simulink model "KUKA_LBR_Simulink_model_flatness_based_control"  (R2017a)
(part 8 of 19)

dblMassInertFullRow5Col2 = -(sin(q1)*(KUKA_LBR_param_.dblLink7InertXY*cos(q4)*sin(q1)*sin(q2) + KUKA_LBR_param_.dblLink7InertXZ*cos(q3)*sin(q2)*sin(q4) + KUKA_LBR_param_.dblLink7InertXX*sin(q1)*sin(q3)*sin(q4) + cos(q2)*(KUKA_LBR_param_.dblLink7InertXZ*cos(q4) - cos(q3)*(KUKA_LBR_param_.dblLink7InertXX*cos(q1) + KUKA_LBR_param_.dblLink7InertXY*sin(q1))*sin(q4)) + cos(q1)*(KUKA_LBR_param_.dblLink7InertXX*cos(q4)*sin(q2) - KUKA_LBR_param_.dblLink7InertXY*sin(q3)*sin(q4)))) + cos(q1)*(KUKA_LBR_param_.dblLink7InertYY*cos(q4)*sin(q1)*sin(q2) + KUKA_LBR_param_.dblLink7InertYZ*cos(q3)*sin(q2)*sin(q4) + KUKA_LBR_param_.dblLink7InertXY*sin(q1)*sin(q3)*sin(q4) + cos(q2)*(KUKA_LBR_param_.dblLink7InertYZ*cos(q4) - cos(q3)*(KUKA_LBR_param_.dblLink7InertXY*cos(q1) + KUKA_LBR_param_.dblLink7InertYY*sin(q1))*sin(q4)) + cos(q1)*(KUKA_LBR_param_.dblLink7InertXY*cos(q4)*sin(q2) - KUKA_LBR_param_.dblLink7InertYY*sin(q3)*sin(q4))) + (-2*KUKA_LBR_param_.dblLink5InertXZ*cos(q2)*cos(q4)*sin(q1) - 2*KUKA_LBR_param_.dblLink5InertXY*cos(q4)*power(sin(q1),2)*sin(q2) + 2*KUKA_LBR_param_.dblLink23Len*KUKA_LBR_param_.dblLink5CogX*KUKA_LBR_param_.dblLink5Mass*cos(q5)*sin(q3) + 2*KUKA_LBR_param_.dblLink45Len*KUKA_LBR_param_.dblLink5CogX*KUKA_LBR_param_.dblLink5Mass*cos(q4)*cos(q5)*sin(q3) + 2*KUKA_LBR_param_.dblLink5CogX*KUKA_LBR_param_.dblLink5CogZ*KUKA_LBR_param_.dblLink5Mass*cos(q4)*cos(q5)*sin(q3) - KUKA_LBR_param_.dblLink5InertXX*sin(q3)*sin(q4) - KUKA_LBR_param_.dblLink5InertYY*sin(q3)*sin(q4) - 2*power(KUKA_LBR_param_.dblLink5CogX,2)*KUKA_LBR_param_.dblLink5Mass*sin(q3)*sin(q4) - 2*power(KUKA_LBR_param_.dblLink5CogY,2)*KUKA_LBR_param_.dblLink5Mass*sin(q3)*sin(q4) - KUKA_LBR_param_.dblLink5InertXX*power(sin(q1),2)*sin(q3)*sin(q4) + KUKA_LBR_param_.dblLink5InertYY*power(sin(q1),2)*sin(q3)*sin(q4) + 2*KUKA_LBR_param_.dblLink5InertXY*sin(2*q1)*sin(q3)*sin(q4) + power(cos(q1),2)*(2*KUKA_LBR_param_.dblLink5InertXY*cos(q4)*sin(q2) + (-2*KUKA_LBR_param_.dblLink5InertXY*cos(q2)*cos(q3) + (KUKA_LBR_param_.dblLink5InertXX - KUKA_LBR_param_.dblLink5InertYY)*sin(q3))*sin(q4)) + 2*cos(q1)*(sin(q2)*(-((KUKA_LBR_param_.dblLink5InertXX - KUKA_LBR_param_.dblLink5InertYY)*cos(q4)*sin(q1)) + KUKA_LBR_param_.dblLink5InertYZ*cos(q3)*sin(q4)) + cos(q2)*(KUKA_LBR_param_.dblLink5InertYZ*cos(q4) + (KUKA_LBR_param_.dblLink5InertXX - KUKA_LBR_param_.dblLink5InertYY)*cos(q3)*sin(q1)*sin(q4))) - 2*KUKA_LBR_param_.dblLink23Len*KUKA_LBR_param_.dblLink5CogY*KUKA_LBR_param_.dblLink5Mass*sin(q3)*sin(q5) - 2*KUKA_LBR_param_.dblLink45Len*KUKA_LBR_param_.dblLink5CogY*KUKA_LBR_param_.dblLink5Mass*cos(q4)*sin(q3)*sin(q5) - 2*KUKA_LBR_param_.dblLink5CogY*KUKA_LBR_param_.dblLink5CogZ*KUKA_LBR_param_.dblLink5Mass*cos(q4)*sin(q3)*sin(q5) + 2*cos(q3)*(KUKA_LBR_param_.dblLink5CogY*KUKA_LBR_param_.dblLink5Mass*(KUKA_LBR_param_.dblLink45Len + KUKA_LBR_param_.dblLink5CogZ + KUKA_LBR_param_.dblLink23Len*cos(q4))*cos(q5) + KUKA_LBR_param_.dblLink5InertXY*cos(q2)*power(sin(q1),2)*sin(q4) - KUKA_LBR_param_.dblLink5InertXZ*sin(q1)*sin(q2)*sin(q4) + KUKA_LBR_param_.dblLink45Len*KUKA_LBR_param_.dblLink5CogX*KUKA_LBR_param_.dblLink5Mass*sin(q5) + KUKA_LBR_param_.dblLink5CogX*KUKA_LBR_param_.dblLink5CogZ*KUKA_LBR_param_.dblLink5Mass*sin(q5) + KUKA_LBR_param_.dblLink23Len*KUKA_LBR_param_.dblLink5CogX*KUKA_LBR_param_.dblLink5Mass*cos(q4)*sin(q5)))/2.0 + (-2*KUKA_LBR_param_.dblLink6InertXZ*cos(q2)*cos(q4)*sin(q1) - 2*KUKA_LBR_param_.dblLink6InertXY*cos(q4)*power(sin(q1),2)*sin(q2) + KUKA_LBR_param_.dblLink6InertYY*cos(q4)*sin(2*q1)*sin(q2) + 2*KUKA_LBR_param_.dblLink23Len*KUKA_LBR_param_.dblLink6CogX*KUKA_LBR_param_.dblLink6Mass*cos(q5)*cos(q6)*sin(q3) + 2*KUKA_LBR_param_.dblLink45Len*KUKA_LBR_param_.dblLink6CogX*KUKA_LBR_param_.dblLink6Mass*cos(q4)*cos(q5)*cos(q6)*sin(q3) + 2*KUKA_LBR_param_.dblLink6CogX*KUKA_LBR_param_.dblLink6CogY*KUKA_LBR_param_.dblLink6Mass*cos(q4)*cos(q5)*power(cos(q6),2)*sin(q3) - KUKA_LBR_param_.dblLink6InertXX*sin(q3)*sin(q4) - KUKA_LBR_param_.dblLink6InertYY*sin(q3)*sin(q4) - power(KUKA_LBR_param_.dblLink6CogX,2)*KUKA_LBR_param_.dblLink6Mass*sin(q3)*sin(q4) - power(KUKA_LBR_param_.dblLink6CogY,2)*KUKA_LBR_param_.dblLink6Mass*sin(q3)*sin(q4) - 2*power(KUKA_LBR_param_.dblLink6CogZ,2)*KUKA_LBR_param_.dblLink6Mass*sin(q3)*sin(q4) - power(KUKA_LBR_param_.dblLink6CogX,2)*KUKA_LBR_param_.dblLink6Mass*power(cos(q6),2)*sin(q3)*sin(q4) + power(KUKA_LBR_param_.dblLink6CogY,2)*KUKA_LBR_param_.dblLink6Mass*power(cos(q6),2)*sin(q3)*sin(q4) - KUKA_LBR_param_.dblLink6InertXX*power(sin(q1),2)*sin(q3)*sin(q4) + KUKA_LBR_param_.dblLink6InertYY*power(sin(q1),2)*sin(q3)*sin(q4) + power(cos(q1),2)*(2*KUKA_LBR_param_.dblLink6InertXY*cos(q4)*sin(q2) + (-2*KUKA_LBR_param_.dblLink6InertXY*cos(q2)*cos(q3) + (KUKA_LBR_param_.dblLink6InertXX - KUKA_LBR_param_.dblLink6InertYY)*sin(q3))*sin(q4)) + 2*cos(q1)*(-(KUKA_LBR_param_.dblLink6InertXX*cos(q4)*sin(q1)*sin(q2)) + KUKA_LBR_param_.dblLink6InertYZ*cos(q3)*sin(q2)*sin(q4) + 2*KUKA_LBR_param_.dblLink6InertXY*sin(q1)*sin(q3)*sin(q4) + cos(q2)*(KUKA_LBR_param_.dblLink6InertYZ*cos(q4) + (KUKA_LBR_param_.dblLink6InertXX - KUKA_LBR_param_.dblLink6InertYY)*cos(q3)*sin(q1)*sin(q4))) + 2*KUKA_LBR_param_.dblLink23Len*KUKA_LBR_param_.dblLink6CogZ*KUKA_LBR_param_.dblLink6Mass*sin(q3)*sin(q5) + 2*KUKA_LBR_param_.dblLink45Len*KUKA_LBR_param_.dblLink6CogZ*KUKA_LBR_param_.dblLink6Mass*cos(q4)*sin(q3)*sin(q5) + 2*KUKA_LBR_param_.dblLink6CogY*KUKA_LBR_param_.dblLink6CogZ*KUKA_LBR_param_.dblLink6Mass*cos(q4)*cos(q6)*sin(q3)*sin(q5) - 2*KUKA_LBR_param_.dblLink23Len*KUKA_LBR_param_.dblLink6CogY*KUKA_LBR_param_.dblLink6Mass*cos(q5)*sin(q3)*sin(q6) - 2*KUKA_LBR_param_.dblLink45Len*KUKA_LBR_param_.dblLink6CogY*KUKA_LBR_param_.dblLink6Mass*cos(q4)*cos(q5)*sin(q3)*sin(q6) - 2*power(KUKA_LBR_param_.dblLink6CogY,2)*KUKA_LBR_param_.dblLink6Mass*cos(q4)*cos(q5)*cos(q6)*sin(q3)*sin(q6) + 4*KUKA_LBR_param_.dblLink6CogX*KUKA_LBR_param_.dblLink6CogY*KUKA_LBR_param_.dblLink6Mass*cos(q6)*sin(q3)*sin(q4)*sin(q6) + 2*KUKA_LBR_param_.dblLink6CogX*KUKA_LBR_param_.dblLink6CogZ*KUKA_LBR_param_.dblLink6Mass*cos(q4)*sin(q3)*sin(q5)*sin(q6) - 2*KUKA_LBR_param_.dblLink6CogX*KUKA_LBR_param_.dblLink6CogY*KUKA_LBR_param_.dblLink6Mass*cos(q4)*cos(q5)*sin(q3)*power(sin(q6),2) + power(KUKA_LBR_param_.dblLink6CogX,2)*KUKA_LBR_param_.dblLink6Mass*sin(q3)*sin(q4)*power(sin(q6),2) - power(KUKA_LBR_param_.dblLink6CogY,2)*KUKA_LBR_param_.dblLink6Mass*sin(q3)*sin(q4)*power(sin(q6),2) + power(KUKA_LBR_param_.dblLink6CogX,2)*KUKA_LBR_param_.dblLink6Mass*cos(q4)*cos(q5)*sin(q3)*sin(2*q6) - cos(q3)*(-2*KUKA_LBR_param_.dblLink6InertXY*cos(q2)*power(sin(q1),2)*sin(q4) + 2*KUKA_LBR_param_.dblLink6InertXZ*sin(q1)*sin(q2)*sin(q4) - 2*KUKA_LBR_param_.dblLink45Len*KUKA_LBR_param_.dblLink6CogX*KUKA_LBR_param_.dblLink6Mass*cos(q6)*sin(q5) - 2*KUKA_LBR_param_.dblLink23Len*KUKA_LBR_param_.dblLink6CogX*KUKA_LBR_param_.dblLink6Mass*cos(q4)*cos(q6)*sin(q5) - 2*KUKA_LBR_param_.dblLink6CogX*KUKA_LBR_param_.dblLink6CogY*KUKA_LBR_param_.dblLink6Mass*power(cos(q6),2)*sin(q5) + 2*KUKA_LBR_param_.dblLink45Len*KUKA_LBR_param_.dblLink6CogY*KUKA_LBR_param_.dblLink6Mass*sin(q5)*sin(q6) + 2*KUKA_LBR_param_.dblLink23Len*KUKA_LBR_param_.dblLink6CogY*KUKA_LBR_param_.dblLink6Mass*cos(q4)*sin(q5)*sin(q6) + 2*KUKA_LBR_param_.dblLink6CogX*KUKA_LBR_param_.dblLink6CogY*KUKA_LBR_param_.dblLink6Mass*sin(q5)*power(sin(q6),2) + 2*KUKA_LBR_param_.dblLink6CogZ*KUKA_LBR_param_.dblLink6Mass*cos(q5)*(KUKA_LBR_param_.dblLink45Len + KUKA_LBR_param_.dblLink23Len*cos(q4) + KUKA_LBR_param_.dblLink6CogY*cos(q6) + KUKA_LBR_param_.dblLink6CogX*sin(q6)) - power(KUKA_LBR_param_.dblLink6CogX,2)*KUKA_LBR_param_.dblLink6Mass*sin(q5)*sin(2*q6) + power(KUKA_LBR_param_.dblLink6CogY,2)*KUKA_LBR_param_.dblLink6Mass*sin(q5)*sin(2*q6)))/2.0 - KUKA_LBR_param_.dblLink7Mass*(cos(q5)*(KUKA_LBR_param_.dblLink7CogZ*sin(q2)*sin(q3)*sin(q6) + cos(q2)*sin(q4)*(KUKA_LBR_param_.dblLink7CogY*cos(q7) + KUKA_LBR_param_.dblLink7CogX*sin(q7)) - cos(q6)*sin(q2)*sin(q3)*(KUKA_LBR_param_.dblLink7CogX*cos(q7) - KUKA_LBR_param_.dblLink7CogY*sin(q7))) + sin(q5)*(cos(q7)*(KUKA_LBR_param_.dblLink7CogY*sin(q2)*sin(q3) + KUKA_LBR_param_.dblLink7CogX*cos(q2)*cos(q6)*sin(q4)) + KUKA_LBR_param_.dblLink7CogX*sin(q2)*sin(q3)*sin(q7) - cos(q2)*sin(q4)*(KUKA_LBR_param_.dblLink7CogZ*sin(q6) + KUKA_LBR_param_.dblLink7CogY*cos(q6)*sin(q7))) - cos(q3)*cos(q4)*sin(q2)*(cos(q5)*(KUKA_LBR_param_.dblLink7CogY*cos(q7) + KUKA_LBR_param_.dblLink7CogX*sin(q7)) - sin(q5)*(KUKA_LBR_param_.dblLink7CogZ*sin(q6) + cos(q6)*(-(KUKA_LBR_param_.dblLink7CogX*cos(q7)) + KUKA_LBR_param_.dblLink7CogY*sin(q7)))))*(sin(q2)*(KUKA_LBR_param_.dblLink23Len + KUKA_LBR_param_.dblLink7CogY*cos(q7)*sin(q4)*sin(q5) + KUKA_LBR_param_.dblLink7CogX*sin(q4)*sin(q5)*sin(q7) + cos(q5)*sin(q4)*(-(KUKA_LBR_param_.dblLink7CogX*cos(q6)*cos(q7)) + KUKA_LBR_param_.dblLink7CogZ*sin(q6) + KUKA_LBR_param_.dblLink7CogY*cos(q6)*sin(q7)) + cos(q4)*(KUKA_LBR_param_.dblLink45Len + KUKA_LBR_param_.dblLink7CogZ*cos(q6) + KUKA_LBR_param_.dblLink7CogX*cos(q7)*sin(q6) - KUKA_LBR_param_.dblLink7CogY*sin(q6)*sin(q7))) + cos(q2)*(sin(q3)*(cos(q5)*(KUKA_LBR_param_.dblLink7CogY*cos(q7) + KUKA_LBR_param_.dblLink7CogX*sin(q7)) + sin(q5)*(KUKA_LBR_param_.dblLink7CogX*cos(q6)*cos(q7) - KUKA_LBR_param_.dblLink7CogZ*sin(q6) - KUKA_LBR_param_.dblLink7CogY*cos(q6)*sin(q7))) + cos(q3)*(-(sin(q4)*(KUKA_LBR_param_.dblLink45Len + KUKA_LBR_param_.dblLink7CogZ*cos(q6) + KUKA_LBR_param_.dblLink7CogX*cos(q7)*sin(q6) - KUKA_LBR_param_.dblLink7CogY*sin(q6)*sin(q7))) + cos(q4)*(sin(q5)*(KUKA_LBR_param_.dblLink7CogY*cos(q7) + KUKA_LBR_param_.dblLink7CogX*sin(q7)) + cos(q5)*(-(KUKA_LBR_param_.dblLink7CogX*cos(q6)*cos(q7)) + KUKA_LBR_param_.dblLink7CogZ*sin(q6) + KUKA_LBR_param_.dblLink7CogY*cos(q6)*sin(q7)))))) + KUKA_LBR_param_.dblLink7Mass*cos(q1)*(cos(q2)*(KUKA_LBR_param_.dblLink23Len + KUKA_LBR_param_.dblLink7CogY*cos(q7)*sin(q4)*sin(q5) + KUKA_LBR_param_.dblLink7CogX*sin(q4)*sin(q5)*sin(q7) + cos(q5)*sin(q4)*(-(KUKA_LBR_param_.dblLink7CogX*cos(q6)*cos(q7)) + KUKA_LBR_param_.dblLink7CogZ*sin(q6) + KUKA_LBR_param_.dblLink7CogY*cos(q6)*sin(q7)) + cos(q4)*(KUKA_LBR_param_.dblLink45Len + KUKA_LBR_param_.dblLink7CogZ*cos(q6) + KUKA_LBR_param_.dblLink7CogX*cos(q7)*sin(q6) - KUKA_LBR_param_.dblLink7CogY*sin(q6)*sin(q7))) + sin(q2)*(-(sin(q3)*(cos(q5)*(KUKA_LBR_param_.dblLink7CogY*cos(q7) + KUKA_LBR_param_.dblLink7CogX*sin(q7)) + sin(q5)*(KUKA_LBR_param_.dblLink7CogX*cos(q6)*cos(q7) - KUKA_LBR_param_.dblLink7CogZ*sin(q6) - KUKA_LBR_param_.dblLink7CogY*cos(q6)*sin(q7)))) + cos(q3)*(sin(q4)*(KUKA_LBR_param_.dblLink45Len + KUKA_LBR_param_.dblLink7CogZ*cos(q6) + KUKA_LBR_param_.dblLink7CogX*cos(q7)*sin(q6) - KUKA_LBR_param_.dblLink7CogY*sin(q6)*sin(q7)) - cos(q4)*(sin(q5)*(KUKA_LBR_param_.dblLink7CogY*cos(q7) + KUKA_LBR_param_.dblLink7CogX*sin(q7)) + cos(q5)*(-(KUKA_LBR_param_.dblLink7CogX*cos(q6)*cos(q7)) + KUKA_LBR_param_.dblLink7CogZ*sin(q6) + KUKA_LBR_param_.dblLink7CogY*cos(q6)*sin(q7))))))*(sin(q1)*(-(cos(q4)*sin(q3)*(cos(q5)*(KUKA_LBR_param_.dblLink7CogY*cos(q7) + KUKA_LBR_param_.dblLink7CogX*sin(q7)) + sin(q5)*(KUKA_LBR_param_.dblLink7CogX*cos(q6)*cos(q7) - KUKA_LBR_param_.dblLink7CogZ*sin(q6) - KUKA_LBR_param_.dblLink7CogY*cos(q6)*sin(q7)))) - cos(q3)*(sin(q5)*(KUKA_LBR_param_.dblLink7CogY*cos(q7) + KUKA_LBR_param_.dblLink7CogX*sin(q7)) + cos(q5)*(-(KUKA_LBR_param_.dblLink7CogX*cos(q6)*cos(q7)) + KUKA_LBR_param_.dblLink7CogZ*sin(q6) + KUKA_LBR_param_.dblLink7CogY*cos(q6)*sin(q7)))) + cos(q1)*(sin(q2)*sin(q4)*(cos(q5)*(KUKA_LBR_param_.dblLink7CogY*cos(q7) + KUKA_LBR_param_.dblLink7CogX*sin(q7)) + sin(q5)*(KUKA_LBR_param_.dblLink7CogX*cos(q6)*cos(q7) - KUKA_LBR_param_.dblLink7CogZ*sin(q6) - KUKA_LBR_param_.dblLink7CogY*cos(q6)*sin(q7))) + cos(q2)*(cos(q3)*cos(q4)*(cos(q5)*(KUKA_LBR_param_.dblLink7CogY*cos(q7) + KUKA_LBR_param_.dblLink7CogX*sin(q7)) + sin(q5)*(KUKA_LBR_param_.dblLink7CogX*cos(q6)*cos(q7) - KUKA_LBR_param_.dblLink7CogZ*sin(q6) - KUKA_LBR_param_.dblLink7CogY*cos(q6)*sin(q7))) - sin(q3)*(sin(q5)*(KUKA_LBR_param_.dblLink7CogY*cos(q7) + KUKA_LBR_param_.dblLink7CogX*sin(q7)) + cos(q5)*(-(KUKA_LBR_param_.dblLink7CogX*cos(q6)*cos(q7)) + KUKA_LBR_param_.dblLink7CogZ*sin(q6) + KUKA_LBR_param_.dblLink7CogY*cos(q6)*sin(q7)))))) + KUKA_LBR_param_.dblLink7Mass*sin(q1)*(cos(q2)*(KUKA_LBR_param_.dblLink23Len + KUKA_LBR_param_.dblLink7CogY*cos(q7)*sin(q4)*sin(q5) + KUKA_LBR_param_.dblLink7CogX*sin(q4)*sin(q5)*sin(q7) + cos(q5)*sin(q4)*(-(KUKA_LBR_param_.dblLink7CogX*cos(q6)*cos(q7)) + KUKA_LBR_param_.dblLink7CogZ*sin(q6) + KUKA_LBR_param_.dblLink7CogY*cos(q6)*sin(q7)) + cos(q4)*(KUKA_LBR_param_.dblLink45Len + KUKA_LBR_param_.dblLink7CogZ*cos(q6) + KUKA_LBR_param_.dblLink7CogX*cos(q7)*sin(q6) - KUKA_LBR_param_.dblLink7CogY*sin(q6)*sin(q7))) + sin(q2)*(-(sin(q3)*(cos(q5)*(KUKA_LBR_param_.dblLink7CogY*cos(q7) + KUKA_LBR_param_.dblLink7CogX*sin(q7)) + sin(q5)*(KUKA_LBR_param_.dblLink7CogX*cos(q6)*cos(q7) - KUKA_LBR_param_.dblLink7CogZ*sin(q6) - KUKA_LBR_param_.dblLink7CogY*cos(q6)*sin(q7)))) + cos(q3)*(sin(q4)*(KUKA_LBR_param_.dblLink45Len + KUKA_LBR_param_.dblLink7CogZ*cos(q6) + KUKA_LBR_param_.dblLink7CogX*cos(q7)*sin(q6) - KUKA_LBR_param_.dblLink7CogY*sin(q6)*sin(q7)) - cos(q4)*(sin(q5)*(KUKA_LBR_param_.dblLink7CogY*cos(q7) + KUKA_LBR_param_.dblLink7CogX*sin(q7)) + cos(q5)*(-(KUKA_LBR_param_.dblLink7CogX*cos(q6)*cos(q7)) + KUKA_LBR_param_.dblLink7CogZ*sin(q6) + KUKA_LBR_param_.dblLink7CogY*cos(q6)*sin(q7))))))*(cos(q1)*(cos(q4)*sin(q3)*(cos(q5)*(KUKA_LBR_param_.dblLink7CogY*cos(q7) + KUKA_LBR_param_.dblLink7CogX*sin(q7)) + sin(q5)*(KUKA_LBR_param_.dblLink7CogX*cos(q6)*cos(q7) - KUKA_LBR_param_.dblLink7CogZ*sin(q6) - KUKA_LBR_param_.dblLink7CogY*cos(q6)*sin(q7))) + cos(q3)*(sin(q5)*(KUKA_LBR_param_.dblLink7CogY*cos(q7) + KUKA_LBR_param_.dblLink7CogX*sin(q7)) + cos(q5)*(-(KUKA_LBR_param_.dblLink7CogX*cos(q6)*cos(q7)) + KUKA_LBR_param_.dblLink7CogZ*sin(q6) + KUKA_LBR_param_.dblLink7CogY*cos(q6)*sin(q7)))) + sin(q1)*(sin(q2)*sin(q4)*(cos(q5)*(KUKA_LBR_param_.dblLink7CogY*cos(q7) + KUKA_LBR_param_.dblLink7CogX*sin(q7)) + sin(q5)*(KUKA_LBR_param_.dblLink7CogX*cos(q6)*cos(q7) - KUKA_LBR_param_.dblLink7CogZ*sin(q6) - KUKA_LBR_param_.dblLink7CogY*cos(q6)*sin(q7))) + cos(q2)*(cos(q3)*cos(q4)*(cos(q5)*(KUKA_LBR_param_.dblLink7CogY*cos(q7) + KUKA_LBR_param_.dblLink7CogX*sin(q7)) + sin(q5)*(KUKA_LBR_param_.dblLink7CogX*cos(q6)*cos(q7) - KUKA_LBR_param_.dblLink7CogZ*sin(q6) - KUKA_LBR_param_.dblLink7CogY*cos(q6)*sin(q7))) - sin(q3)*(sin(q5)*(KUKA_LBR_param_.dblLink7CogY*cos(q7) + KUKA_LBR_param_.dblLink7CogX*sin(q7)) + cos(q5)*(-(KUKA_LBR_param_.dblLink7CogX*cos(q6)*cos(q7)) + KUKA_LBR_param_.dblLink7CogZ*sin(q6) + KUKA_LBR_param_.dblLink7CogY*cos(q6)*sin(q7))))));
dblMassInertFullRow5Col3 = cos(q1)*sin(q2)*(KUKA_LBR_param_.dblLink7InertXY*cos(q4)*sin(q1)*sin(q2) + KUKA_LBR_param_.dblLink7InertXZ*cos(q3)*sin(q2)*sin(q4) + KUKA_LBR_param_.dblLink7InertXX*sin(q1)*sin(q3)*sin(q4) + cos(q2)*(KUKA_LBR_param_.dblLink7InertXZ*cos(q4) - cos(q3)*(KUKA_LBR_param_.dblLink7InertXX*cos(q1) + KUKA_LBR_param_.dblLink7InertXY*sin(q1))*sin(q4)) + cos(q1)*(KUKA_LBR_param_.dblLink7InertXX*cos(q4)*sin(q2) - KUKA_LBR_param_.dblLink7InertXY*sin(q3)*sin(q4))) + sin(q1)*sin(q2)*(KUKA_LBR_param_.dblLink7InertYY*cos(q4)*sin(q1)*sin(q2) + KUKA_LBR_param_.dblLink7InertYZ*cos(q3)*sin(q2)*sin(q4) + KUKA_LBR_param_.dblLink7InertXY*sin(q1)*sin(q3)*sin(q4) + cos(q2)*(KUKA_LBR_param_.dblLink7InertYZ*cos(q4) - cos(q3)*(KUKA_LBR_param_.dblLink7InertXY*cos(q1) + KUKA_LBR_param_.dblLink7InertYY*sin(q1))*sin(q4)) + cos(q1)*(KUKA_LBR_param_.dblLink7InertXY*cos(q4)*sin(q2) - KUKA_LBR_param_.dblLink7InertYY*sin(q3)*sin(q4))) + cos(q2)*(KUKA_LBR_param_.dblLink7InertYZ*cos(q4)*sin(q1)*sin(q2) + KUKA_LBR_param_.dblLink7InertZZ*cos(q3)*sin(q2)*sin(q4) + KUKA_LBR_param_.dblLink7InertXZ*sin(q1)*sin(q3)*sin(q4) + cos(q2)*(KUKA_LBR_param_.dblLink7InertZZ*cos(q4) - cos(q3)*(KUKA_LBR_param_.dblLink7InertXZ*cos(q1) + KUKA_LBR_param_.dblLink7InertYZ*sin(q1))*sin(q4)) + cos(q1)*(KUKA_LBR_param_.dblLink7InertXZ*cos(q4)*sin(q2) - KUKA_LBR_param_.dblLink7InertYZ*sin(q3)*sin(q4))) + (cos(q4)*(2*KUKA_LBR_param_.dblLink5InertXX + 2*KUKA_LBR_param_.dblLink5InertYY + 4*KUKA_LBR_param_.dblLink5InertZZ + 8*power(KUKA_LBR_param_.dblLink5CogX,2)*KUKA_LBR_param_.dblLink5Mass + 8*power(KUKA_LBR_param_.dblLink5CogY,2)*KUKA_LBR_param_.dblLink5Mass + 2*(KUKA_LBR_param_.dblLink5InertXX - KUKA_LBR_param_.dblLink5InertYY)*cos(2*q1) + 4*KUKA_LBR_param_.dblLink5InertYZ*cos(q1 - 2*q2) - KUKA_LBR_param_.dblLink5InertXX*cos(2*(q1 - q2)) + KUKA_LBR_param_.dblLink5InertYY*cos(2*(q1 - q2)) - 2*KUKA_LBR_param_.dblLink5InertXX*cos(2*q2) - 2*KUKA_LBR_param_.dblLink5InertYY*cos(2*q2) + 4*KUKA_LBR_param_.dblLink5InertZZ*cos(2*q2) - KUKA_LBR_param_.dblLink5InertXX*cos(2*(q1 + q2)) + KUKA_LBR_param_.dblLink5InertYY*cos(2*(q1 + q2)) - 4*KUKA_LBR_param_.dblLink5InertYZ*cos(q1 + 2*q2) + 4*KUKA_LBR_param_.dblLink5InertXY*sin(2*q1) - 4*KUKA_LBR_param_.dblLink5InertXZ*sin(q1 - 2*q2) - 2*KUKA_LBR_param_.dblLink5InertXY*sin(2*(q1 - q2)) - 2*KUKA_LBR_param_.dblLink5InertXY*sin(2*(q1 + q2)) + 4*KUKA_LBR_param_.dblLink5InertXZ*sin(q1 + 2*q2)) - 4*sin(q4)*(-2*KUKA_LBR_param_.dblLink5CogX*(KUKA_LBR_param_.dblLink45Len + KUKA_LBR_param_.dblLink5CogZ)*KUKA_LBR_param_.dblLink5Mass*cos(q5) + 2*KUKA_LBR_param_.dblLink5InertYZ*power(cos(q2),2)*cos(q3)*sin(q1) + KUKA_LBR_param_.dblLink5InertXX*cos(q2)*cos(q3)*sin(q2) + KUKA_LBR_param_.dblLink5InertYY*cos(q2)*cos(q3)*sin(q2) - 2*KUKA_LBR_param_.dblLink5InertZZ*cos(q2)*cos(q3)*sin(q2) - KUKA_LBR_param_.dblLink5InertXX*cos(q2)*cos(q3)*power(sin(q1),2)*sin(q2) + KUKA_LBR_param_.dblLink5InertYY*cos(q2)*cos(q3)*power(sin(q1),2)*sin(q2) - 2*KUKA_LBR_param_.dblLink5InertYZ*cos(q3)*sin(q1)*power(sin(q2),2) + KUKA_LBR_param_.dblLink5InertXY*cos(q3)*sin(2*q1)*sin(2*q2) - 2*KUKA_LBR_param_.dblLink5InertXZ*cos(q2)*sin(q1)*sin(q3) - 2*KUKA_LBR_param_.dblLink5InertXY*power(sin(q1),2)*sin(q2)*sin(q3) + KUKA_LBR_param_.dblLink5InertYY*sin(2*q1)*sin(q2)*sin(q3) + power(cos(q1),2)*sin(q2)*((KUKA_LBR_param_.dblLink5InertXX - KUKA_LBR_param_.dblLink5InertYY)*cos(q2)*cos(q3) + 2*KUKA_LBR_param_.dblLink5InertXY*sin(q3)) + 2*cos(q1)*(KUKA_LBR_param_.dblLink5InertXZ*power(cos(q2),2)*cos(q3) + KUKA_LBR_param_.dblLink5InertYZ*cos(q2)*sin(q3) - sin(q2)*(KUKA_LBR_param_.dblLink5InertXZ*cos(q3)*sin(q2) + KUKA_LBR_param_.dblLink5InertXX*sin(q1)*sin(q3))) + 2*KUKA_LBR_param_.dblLink45Len*KUKA_LBR_param_.dblLink5CogY*KUKA_LBR_param_.dblLink5Mass*sin(q5) + 2*KUKA_LBR_param_.dblLink5CogY*KUKA_LBR_param_.dblLink5CogZ*KUKA_LBR_param_.dblLink5Mass*sin(q5)))/8.0 + (2*sin(q4)*(-4*KUKA_LBR_param_.dblLink6InertYZ*power(cos(q2),2)*cos(q3)*sin(q1) - 2*KUKA_LBR_param_.dblLink6InertXX*cos(q2)*cos(q3)*sin(q2) - 2*KUKA_LBR_param_.dblLink6InertYY*cos(q2)*cos(q3)*sin(q2) + 4*KUKA_LBR_param_.dblLink6InertZZ*cos(q2)*cos(q3)*sin(q2) - 2*KUKA_LBR_param_.dblLink6InertYY*cos(q2)*cos(q3)*power(sin(q1),2)*sin(q2) + 4*KUKA_LBR_param_.dblLink6InertYZ*cos(q3)*sin(q1)*power(sin(q2),2) + KUKA_LBR_param_.dblLink6InertXX*cos(q3)*power(sin(q1),2)*sin(2*q2) + 4*KUKA_LBR_param_.dblLink6InertXZ*cos(q2)*sin(q1)*sin(q3) + 4*KUKA_LBR_param_.dblLink6InertXY*power(sin(q1),2)*sin(q2)*sin(q3) + power(cos(q1),2)*(-2*KUKA_LBR_param_.dblLink6InertXX*cos(q2)*cos(q3)*sin(q2) + KUKA_LBR_param_.dblLink6InertYY*cos(q3)*sin(2*q2) - 4*KUKA_LBR_param_.dblLink6InertXY*sin(q2)*sin(q3)) - 4*cos(q1)*(KUKA_LBR_param_.dblLink6InertXZ*power(cos(q2),2)*cos(q3) + cos(q3)*(-(KUKA_LBR_param_.dblLink6InertXZ*power(sin(q2),2)) + KUKA_LBR_param_.dblLink6InertXY*sin(q1)*sin(2*q2)) + KUKA_LBR_param_.dblLink6InertYZ*cos(q2)*sin(q3) + (-KUKA_LBR_param_.dblLink6InertXX + KUKA_LBR_param_.dblLink6InertYY)*sin(q1)*sin(q2)*sin(q3)) + 4*KUKA_LBR_param_.dblLink45Len*KUKA_LBR_param_.dblLink6CogZ*KUKA_LBR_param_.dblLink6Mass*sin(q5) + 4*KUKA_LBR_param_.dblLink6CogY*KUKA_LBR_param_.dblLink6CogZ*KUKA_LBR_param_.dblLink6Mass*cos(q6)*sin(q5) + 4*KUKA_LBR_param_.dblLink6CogX*KUKA_LBR_param_.dblLink6CogZ*KUKA_LBR_param_.dblLink6Mass*sin(q5)*sin(q6) + 4*KUKA_LBR_param_.dblLink6Mass*cos(q5)*(KUKA_LBR_param_.dblLink45Len + KUKA_LBR_param_.dblLink6CogY*cos(q6) + KUKA_LBR_param_.dblLink6CogX*sin(q6))*(KUKA_LBR_param_.dblLink6CogX*cos(q6) - KUKA_LBR_param_.dblLink6CogY*sin(q6))) + cos(q4)*(2*KUKA_LBR_param_.dblLink6InertXX + 2*KUKA_LBR_param_.dblLink6InertYY + 4*KUKA_LBR_param_.dblLink6InertZZ + 4*power(KUKA_LBR_param_.dblLink6CogX,2)*KUKA_LBR_param_.dblLink6Mass + 4*power(KUKA_LBR_param_.dblLink6CogY,2)*KUKA_LBR_param_.dblLink6Mass + 8*power(KUKA_LBR_param_.dblLink6CogZ,2)*KUKA_LBR_param_.dblLink6Mass + 2*(KUKA_LBR_param_.dblLink6InertXX - KUKA_LBR_param_.dblLink6InertYY)*cos(2*q1) + 4*KUKA_LBR_param_.dblLink6InertYZ*cos(q1 - 2*q2) - KUKA_LBR_param_.dblLink6InertXX*cos(2*(q1 - q2)) + KUKA_LBR_param_.dblLink6InertYY*cos(2*(q1 - q2)) - 2*KUKA_LBR_param_.dblLink6InertXX*cos(2*q2) - 2*KUKA_LBR_param_.dblLink6InertYY*cos(2*q2) + 4*KUKA_LBR_param_.dblLink6InertZZ*cos(2*q2) - KUKA_LBR_param_.dblLink6InertXX*cos(2*(q1 + q2)) + KUKA_LBR_param_.dblLink6InertYY*cos(2*(q1 + q2)) - 4*KUKA_LBR_param_.dblLink6InertYZ*cos(q1 + 2*q2) + 4*power(KUKA_LBR_param_.dblLink6CogX,2)*KUKA_LBR_param_.dblLink6Mass*cos(2*q6) - 4*power(KUKA_LBR_param_.dblLink6CogY,2)*KUKA_LBR_param_.dblLink6Mass*cos(2*q6) + 4*KUKA_LBR_param_.dblLink6InertXY*sin(2*q1) - 4*KUKA_LBR_param_.dblLink6InertXZ*sin(q1 - 2*q2) - 2*KUKA_LBR_param_.dblLink6InertXY*sin(2*(q1 - q2)) - 2*KUKA_LBR_param_.dblLink6InertXY*sin(2*(q1 + q2)) + 4*KUKA_LBR_param_.dblLink6InertXZ*sin(q1 + 2*q2) - 8*KUKA_LBR_param_.dblLink6CogX*KUKA_LBR_param_.dblLink6CogY*KUKA_LBR_param_.dblLink6Mass*sin(2*q6)))/8.0 + KUKA_LBR_param_.dblLink7Mass*sin(q2)*(cos(q5)*(KUKA_LBR_param_.dblLink7CogZ*sin(q2)*sin(q3)*sin(q6) + cos(q2)*sin(q4)*(KUKA_LBR_param_.dblLink7CogY*cos(q7) + KUKA_LBR_param_.dblLink7CogX*sin(q7)) - cos(q6)*sin(q2)*sin(q3)*(KUKA_LBR_param_.dblLink7CogX*cos(q7) - KUKA_LBR_param_.dblLink7CogY*sin(q7))) + sin(q5)*(cos(q7)*(KUKA_LBR_param_.dblLink7CogY*sin(q2)*sin(q3) + KUKA_LBR_param_.dblLink7CogX*cos(q2)*cos(q6)*sin(q4)) + KUKA_LBR_param_.dblLink7CogX*sin(q2)*sin(q3)*sin(q7) - cos(q2)*sin(q4)*(KUKA_LBR_param_.dblLink7CogZ*sin(q6) + KUKA_LBR_param_.dblLink7CogY*cos(q6)*sin(q7))) - cos(q3)*cos(q4)*sin(q2)*(cos(q5)*(KUKA_LBR_param_.dblLink7CogY*cos(q7) + KUKA_LBR_param_.dblLink7CogX*sin(q7)) - sin(q5)*(KUKA_LBR_param_.dblLink7CogZ*sin(q6) + cos(q6)*(-(KUKA_LBR_param_.dblLink7CogX*cos(q7)) + KUKA_LBR_param_.dblLink7CogY*sin(q7)))))*(-(cos(q3)*(cos(q5)*(KUKA_LBR_param_.dblLink7CogY*cos(q7) + KUKA_LBR_param_.dblLink7CogX*sin(q7)) + sin(q5)*(KUKA_LBR_param_.dblLink7CogX*cos(q6)*cos(q7) - KUKA_LBR_param_.dblLink7CogZ*sin(q6) - KUKA_LBR_param_.dblLink7CogY*cos(q6)*sin(q7)))) + sin(q3)*(-(sin(q4)*(KUKA_LBR_param_.dblLink45Len + KUKA_LBR_param_.dblLink7CogZ*cos(q6) + KUKA_LBR_param_.dblLink7CogX*cos(q7)*sin(q6) - KUKA_LBR_param_.dblLink7CogY*sin(q6)*sin(q7))) + cos(q4)*(sin(q5)*(KUKA_LBR_param_.dblLink7CogY*cos(q7) + KUKA_LBR_param_.dblLink7CogX*sin(q7)) + cos(q5)*(-(KUKA_LBR_param_.dblLink7CogX*cos(q6)*cos(q7)) + KUKA_LBR_param_.dblLink7CogZ*sin(q6) + KUKA_LBR_param_.dblLink7CogY*cos(q6)*sin(q7))))) + KUKA_LBR_param_.dblLink7Mass*(sin(q1)*(-(sin(q3)*(cos(q5)*(KUKA_LBR_param_.dblLink7CogY*cos(q7) + KUKA_LBR_param_.dblLink7CogX*sin(q7)) + sin(q5)*(KUKA_LBR_param_.dblLink7CogX*cos(q6)*cos(q7) - KUKA_LBR_param_.dblLink7CogZ*sin(q6) - KUKA_LBR_param_.dblLink7CogY*cos(q6)*sin(q7)))) + cos(q3)*(sin(q4)*(KUKA_LBR_param_.dblLink45Len + KUKA_LBR_param_.dblLink7CogZ*cos(q6) + KUKA_LBR_param_.dblLink7CogX*cos(q7)*sin(q6) - KUKA_LBR_param_.dblLink7CogY*sin(q6)*sin(q7)) - cos(q4)*(sin(q5)*(KUKA_LBR_param_.dblLink7CogY*cos(q7) + KUKA_LBR_param_.dblLink7CogX*sin(q7)) + cos(q5)*(-(KUKA_LBR_param_.dblLink7CogX*cos(q6)*cos(q7)) + KUKA_LBR_param_.dblLink7CogZ*sin(q6) + KUKA_LBR_param_.dblLink7CogY*cos(q6)*sin(q7))))) + cos(q1)*cos(q2)*(cos(q3)*(cos(q5)*(KUKA_LBR_param_.dblLink7CogY*cos(q7) + KUKA_LBR_param_.dblLink7CogX*sin(q7)) + sin(q5)*(KUKA_LBR_param_.dblLink7CogX*cos(q6)*cos(q7) - KUKA_LBR_param_.dblLink7CogZ*sin(q6) - KUKA_LBR_param_.dblLink7CogY*cos(q6)*sin(q7))) + sin(q3)*(sin(q4)*(KUKA_LBR_param_.dblLink45Len + KUKA_LBR_param_.dblLink7CogZ*cos(q6) + KUKA_LBR_param_.dblLink7CogX*cos(q7)*sin(q6) - KUKA_LBR_param_.dblLink7CogY*sin(q6)*sin(q7)) - cos(q4)*(sin(q5)*(KUKA_LBR_param_.dblLink7CogY*cos(q7) + KUKA_LBR_param_.dblLink7CogX*sin(q7)) + cos(q5)*(-(KUKA_LBR_param_.dblLink7CogX*cos(q6)*cos(q7)) + KUKA_LBR_param_.dblLink7CogZ*sin(q6) + KUKA_LBR_param_.dblLink7CogY*cos(q6)*sin(q7))))))*(sin(q1)*(-(cos(q4)*sin(q3)*(cos(q5)*(KUKA_LBR_param_.dblLink7CogY*cos(q7) + KUKA_LBR_param_.dblLink7CogX*sin(q7)) + sin(q5)*(KUKA_LBR_param_.dblLink7CogX*cos(q6)*cos(q7) - KUKA_LBR_param_.dblLink7CogZ*sin(q6) - KUKA_LBR_param_.dblLink7CogY*cos(q6)*sin(q7)))) - cos(q3)*(sin(q5)*(KUKA_LBR_param_.dblLink7CogY*cos(q7) + KUKA_LBR_param_.dblLink7CogX*sin(q7)) + cos(q5)*(-(KUKA_LBR_param_.dblLink7CogX*cos(q6)*cos(q7)) + KUKA_LBR_param_.dblLink7CogZ*sin(q6) + KUKA_LBR_param_.dblLink7CogY*cos(q6)*sin(q7)))) + cos(q1)*(sin(q2)*sin(q4)*(cos(q5)*(KUKA_LBR_param_.dblLink7CogY*cos(q7) + KUKA_LBR_param_.dblLink7CogX*sin(q7)) + sin(q5)*(KUKA_LBR_param_.dblLink7CogX*cos(q6)*cos(q7) - KUKA_LBR_param_.dblLink7CogZ*sin(q6) - KUKA_LBR_param_.dblLink7CogY*cos(q6)*sin(q7))) + cos(q2)*(cos(q3)*cos(q4)*(cos(q5)*(KUKA_LBR_param_.dblLink7CogY*cos(q7) + KUKA_LBR_param_.dblLink7CogX*sin(q7)) + sin(q5)*(KUKA_LBR_param_.dblLink7CogX*cos(q6)*cos(q7) - KUKA_LBR_param_.dblLink7CogZ*sin(q6) - KUKA_LBR_param_.dblLink7CogY*cos(q6)*sin(q7))) - sin(q3)*(sin(q5)*(KUKA_LBR_param_.dblLink7CogY*cos(q7) + KUKA_LBR_param_.dblLink7CogX*sin(q7)) + cos(q5)*(-(KUKA_LBR_param_.dblLink7CogX*cos(q6)*cos(q7)) + KUKA_LBR_param_.dblLink7CogZ*sin(q6) + KUKA_LBR_param_.dblLink7CogY*cos(q6)*sin(q7)))))) + KUKA_LBR_param_.dblLink7Mass*(cos(q2)*sin(q1)*(cos(q3)*(cos(q5)*(KUKA_LBR_param_.dblLink7CogY*cos(q7) + KUKA_LBR_param_.dblLink7CogX*sin(q7)) + sin(q5)*(KUKA_LBR_param_.dblLink7CogX*cos(q6)*cos(q7) - KUKA_LBR_param_.dblLink7CogZ*sin(q6) - KUKA_LBR_param_.dblLink7CogY*cos(q6)*sin(q7))) + sin(q3)*(sin(q4)*(KUKA_LBR_param_.dblLink45Len + KUKA_LBR_param_.dblLink7CogZ*cos(q6) + KUKA_LBR_param_.dblLink7CogX*cos(q7)*sin(q6) - KUKA_LBR_param_.dblLink7CogY*sin(q6)*sin(q7)) - cos(q4)*(sin(q5)*(KUKA_LBR_param_.dblLink7CogY*cos(q7) + KUKA_LBR_param_.dblLink7CogX*sin(q7)) + cos(q5)*(-(KUKA_LBR_param_.dblLink7CogX*cos(q6)*cos(q7)) + KUKA_LBR_param_.dblLink7CogZ*sin(q6) + KUKA_LBR_param_.dblLink7CogY*cos(q6)*sin(q7))))) + cos(q1)*(sin(q3)*(cos(q5)*(KUKA_LBR_param_.dblLink7CogY*cos(q7) + KUKA_LBR_param_.dblLink7CogX*sin(q7)) + sin(q5)*(KUKA_LBR_param_.dblLink7CogX*cos(q6)*cos(q7) - KUKA_LBR_param_.dblLink7CogZ*sin(q6) - KUKA_LBR_param_.dblLink7CogY*cos(q6)*sin(q7))) + cos(q3)*(-(sin(q4)*(KUKA_LBR_param_.dblLink45Len + KUKA_LBR_param_.dblLink7CogZ*cos(q6) + KUKA_LBR_param_.dblLink7CogX*cos(q7)*sin(q6) - KUKA_LBR_param_.dblLink7CogY*sin(q6)*sin(q7))) + cos(q4)*(sin(q5)*(KUKA_LBR_param_.dblLink7CogY*cos(q7) + KUKA_LBR_param_.dblLink7CogX*sin(q7)) + cos(q5)*(-(KUKA_LBR_param_.dblLink7CogX*cos(q6)*cos(q7)) + KUKA_LBR_param_.dblLink7CogZ*sin(q6) + KUKA_LBR_param_.dblLink7CogY*cos(q6)*sin(q7))))))*(cos(q1)*(cos(q4)*sin(q3)*(cos(q5)*(KUKA_LBR_param_.dblLink7CogY*cos(q7) + KUKA_LBR_param_.dblLink7CogX*sin(q7)) + sin(q5)*(KUKA_LBR_param_.dblLink7CogX*cos(q6)*cos(q7) - KUKA_LBR_param_.dblLink7CogZ*sin(q6) - KUKA_LBR_param_.dblLink7CogY*cos(q6)*sin(q7))) + cos(q3)*(sin(q5)*(KUKA_LBR_param_.dblLink7CogY*cos(q7) + KUKA_LBR_param_.dblLink7CogX*sin(q7)) + cos(q5)*(-(KUKA_LBR_param_.dblLink7CogX*cos(q6)*cos(q7)) + KUKA_LBR_param_.dblLink7CogZ*sin(q6) + KUKA_LBR_param_.dblLink7CogY*cos(q6)*sin(q7)))) + sin(q1)*(sin(q2)*sin(q4)*(cos(q5)*(KUKA_LBR_param_.dblLink7CogY*cos(q7) + KUKA_LBR_param_.dblLink7CogX*sin(q7)) + sin(q5)*(KUKA_LBR_param_.dblLink7CogX*cos(q6)*cos(q7) - KUKA_LBR_param_.dblLink7CogZ*sin(q6) - KUKA_LBR_param_.dblLink7CogY*cos(q6)*sin(q7))) + cos(q2)*(cos(q3)*cos(q4)*(cos(q5)*(KUKA_LBR_param_.dblLink7CogY*cos(q7) + KUKA_LBR_param_.dblLink7CogX*sin(q7)) + sin(q5)*(KUKA_LBR_param_.dblLink7CogX*cos(q6)*cos(q7) - KUKA_LBR_param_.dblLink7CogZ*sin(q6) - KUKA_LBR_param_.dblLink7CogY*cos(q6)*sin(q7))) - sin(q3)*(sin(q5)*(KUKA_LBR_param_.dblLink7CogY*cos(q7) + KUKA_LBR_param_.dblLink7CogX*sin(q7)) + cos(q5)*(-(KUKA_LBR_param_.dblLink7CogX*cos(q6)*cos(q7)) + KUKA_LBR_param_.dblLink7CogZ*sin(q6) + KUKA_LBR_param_.dblLink7CogY*cos(q6)*sin(q7))))));
dblMassInertFullRow5Col4 = (cos(q3)*sin(q1) + cos(q1)*cos(q2)*sin(q3))*(KUKA_LBR_param_.dblLink7InertXY*cos(q4)*sin(q1)*sin(q2) + KUKA_LBR_param_.dblLink7InertXZ*cos(q3)*sin(q2)*sin(q4) + KUKA_LBR_param_.dblLink7InertXX*sin(q1)*sin(q3)*sin(q4) + cos(q2)*(KUKA_LBR_param_.dblLink7InertXZ*cos(q4) - cos(q3)*(KUKA_LBR_param_.dblLink7InertXX*cos(q1) + KUKA_LBR_param_.dblLink7InertXY*sin(q1))*sin(q4)) + cos(q1)*(KUKA_LBR_param_.dblLink7InertXX*cos(q4)*sin(q2) - KUKA_LBR_param_.dblLink7InertXY*sin(q3)*sin(q4))) + (-(cos(q1)*cos(q3)) + cos(q2)*sin(q1)*sin(q3))*(KUKA_LBR_param_.dblLink7InertYY*cos(q4)*sin(q1)*sin(q2) + KUKA_LBR_param_.dblLink7InertYZ*cos(q3)*sin(q2)*sin(q4) + KUKA_LBR_param_.dblLink7InertXY*sin(q1)*sin(q3)*sin(q4) + cos(q2)*(KUKA_LBR_param_.dblLink7InertYZ*cos(q4) - cos(q3)*(KUKA_LBR_param_.dblLink7InertXY*cos(q1) + KUKA_LBR_param_.dblLink7InertYY*sin(q1))*sin(q4)) + cos(q1)*(KUKA_LBR_param_.dblLink7InertXY*cos(q4)*sin(q2) - KUKA_LBR_param_.dblLink7InertYY*sin(q3)*sin(q4))) - sin(q2)*sin(q3)*(KUKA_LBR_param_.dblLink7InertYZ*cos(q4)*sin(q1)*sin(q2) + KUKA_LBR_param_.dblLink7InertZZ*cos(q3)*sin(q2)*sin(q4) + KUKA_LBR_param_.dblLink7InertXZ*sin(q1)*sin(q3)*sin(q4) + cos(q2)*(KUKA_LBR_param_.dblLink7InertZZ*cos(q4) - cos(q3)*(KUKA_LBR_param_.dblLink7InertXZ*cos(q1) + KUKA_LBR_param_.dblLink7InertYZ*sin(q1))*sin(q4)) + cos(q1)*(KUKA_LBR_param_.dblLink7InertXZ*cos(q4)*sin(q2) - KUKA_LBR_param_.dblLink7InertYZ*sin(q3)*sin(q4))) + (-4*KUKA_LBR_param_.dblLink5CogY*(KUKA_LBR_param_.dblLink45Len + KUKA_LBR_param_.dblLink5CogZ)*KUKA_LBR_param_.dblLink5Mass*cos(q5) + 4*KUKA_LBR_param_.dblLink5InertXZ*cos(q2)*cos(q3)*cos(q4)*sin(q1) + 4*KUKA_LBR_param_.dblLink5InertXY*cos(q3)*cos(q4)*power(sin(q1),2)*sin(q2) + 4*KUKA_LBR_param_.dblLink5InertYZ*power(cos(q2),2)*cos(q4)*sin(q1)*sin(q3) - 4*KUKA_LBR_param_.dblLink5InertZZ*cos(q2)*cos(q4)*sin(q2)*sin(q3) - 2*KUKA_LBR_param_.dblLink5InertXX*cos(q2)*cos(q4)*power(sin(q1),2)*sin(q2)*sin(q3) - 4*KUKA_LBR_param_.dblLink5InertYZ*cos(q4)*sin(q1)*power(sin(q2),2)*sin(q3) + KUKA_LBR_param_.dblLink5InertXX*cos(q4)*sin(2*q2)*sin(q3) + KUKA_LBR_param_.dblLink5InertYY*cos(q4)*sin(2*q2)*sin(q3) + KUKA_LBR_param_.dblLink5InertYY*cos(q4)*power(sin(q1),2)*sin(2*q2)*sin(q3) - 4*KUKA_LBR_param_.dblLink5InertXY*cos(q2)*power(cos(q3),2)*power(sin(q1),2)*sin(q4) + 4*KUKA_LBR_param_.dblLink5InertXZ*power(cos(q3),2)*sin(q1)*sin(q2)*sin(q4) + KUKA_LBR_param_.dblLink5InertXX*cos(q3)*sin(q3)*sin(q4) + KUKA_LBR_param_.dblLink5InertYY*cos(q3)*sin(q3)*sin(q4) - 2*KUKA_LBR_param_.dblLink5InertZZ*cos(q3)*sin(q3)*sin(q4) - KUKA_LBR_param_.dblLink5InertXX*power(cos(q2),2)*cos(q3)*sin(q3)*sin(q4) - KUKA_LBR_param_.dblLink5InertYY*power(cos(q2),2)*cos(q3)*sin(q3)*sin(q4) + 3*KUKA_LBR_param_.dblLink5InertXX*cos(q3)*power(sin(q1),2)*sin(q3)*sin(q4) - 3*KUKA_LBR_param_.dblLink5InertYY*cos(q3)*power(sin(q1),2)*sin(q3)*sin(q4) + KUKA_LBR_param_.dblLink5InertXX*power(cos(q2),2)*cos(q3)*power(sin(q1),2)*sin(q3)*sin(q4) - KUKA_LBR_param_.dblLink5InertYY*power(cos(q2),2)*cos(q3)*power(sin(q1),2)*sin(q3)*sin(q4) + 8*KUKA_LBR_param_.dblLink5InertYZ*cos(q2)*cos(q3)*sin(q1)*sin(q2)*sin(q3)*sin(q4) + KUKA_LBR_param_.dblLink5InertXX*cos(q3)*power(sin(q2),2)*sin(q3)*sin(q4) + KUKA_LBR_param_.dblLink5InertYY*cos(q3)*power(sin(q2),2)*sin(q3)*sin(q4) - 2*KUKA_LBR_param_.dblLink5InertZZ*cos(q3)*power(sin(q2),2)*sin(q3)*sin(q4) - KUKA_LBR_param_.dblLink5InertXX*cos(q3)*power(sin(q1),2)*power(sin(q2),2)*sin(q3)*sin(q4) + KUKA_LBR_param_.dblLink5InertYY*cos(q3)*power(sin(q1),2)*power(sin(q2),2)*sin(q3)*sin(q4) + 4*KUKA_LBR_param_.dblLink5InertXY*cos(q2)*power(sin(q1),2)*power(sin(q3),2)*sin(q4) - 4*KUKA_LBR_param_.dblLink5InertXZ*sin(q1)*sin(q2)*power(sin(q3),2)*sin(q4) + KUKA_LBR_param_.dblLink5InertZZ*power(cos(q2),2)*sin(2*q3)*sin(q4) - 3*KUKA_LBR_param_.dblLink5InertXY*sin(2*q1)*sin(2*q3)*sin(q4) + KUKA_LBR_param_.dblLink5InertXY*sin(2*q1)*power(sin(q2),2)*sin(2*q3)*sin(q4) + power(cos(q1),2)*(4*KUKA_LBR_param_.dblLink5InertXY*cos(q2)*power(cos(q3),2)*sin(q4) + cos(q3)*(-4*KUKA_LBR_param_.dblLink5InertXY*cos(q4)*sin(q2) - (KUKA_LBR_param_.dblLink5InertXX - KUKA_LBR_param_.dblLink5InertYY)*(3 + cos(2*q2))*sin(q3)*sin(q4)) + sin(q3)*(KUKA_LBR_param_.dblLink5InertXX*cos(q4)*sin(2*q2) - 2*cos(q2)*(KUKA_LBR_param_.dblLink5InertYY*cos(q4)*sin(q2) + 2*KUKA_LBR_param_.dblLink5InertXY*sin(q3)*sin(q4)))) - 4*cos(q1)*(power(cos(q2),2)*sin(q3)*(-(KUKA_LBR_param_.dblLink5InertXZ*cos(q4)) + KUKA_LBR_param_.dblLink5InertXY*cos(q3)*sin(q1)*sin(q4)) + sin(q2)*(-((KUKA_LBR_param_.dblLink5InertXX - KUKA_LBR_param_.dblLink5InertYY)*cos(q3)*cos(q4)*sin(q1)) + KUKA_LBR_param_.dblLink5InertYZ*power(cos(q3),2)*sin(q4) + sin(q3)*(KUKA_LBR_param_.dblLink5InertXZ*cos(q4)*sin(q2) - KUKA_LBR_param_.dblLink5InertYZ*sin(q3)*sin(q4))) + cos(q2)*((KUKA_LBR_param_.dblLink5InertXX - KUKA_LBR_param_.dblLink5InertYY)*power(cos(q3),2)*sin(q1)*sin(q4) + sin(q1)*sin(q3)*(-2*KUKA_LBR_param_.dblLink5InertXY*cos(q4)*sin(q2) + (-KUKA_LBR_param_.dblLink5InertXX + KUKA_LBR_param_.dblLink5InertYY)*sin(q3)*sin(q4)) + cos(q3)*(KUKA_LBR_param_.dblLink5InertYZ*cos(q4) - 2*KUKA_LBR_param_.dblLink5InertXZ*sin(q2)*sin(q3)*sin(q4)))) - 4*KUKA_LBR_param_.dblLink45Len*KUKA_LBR_param_.dblLink5CogX*KUKA_LBR_param_.dblLink5Mass*sin(q5) - 4*KUKA_LBR_param_.dblLink5CogX*KUKA_LBR_param_.dblLink5CogZ*KUKA_LBR_param_.dblLink5Mass*sin(q5))/4.0 + (4*KUKA_LBR_param_.dblLink6InertXZ*cos(q2)*cos(q3)*cos(q4)*sin(q1) + 4*KUKA_LBR_param_.dblLink6InertXY*cos(q3)*cos(q4)*power(sin(q1),2)*sin(q2) + 4*KUKA_LBR_param_.dblLink6InertYZ*power(cos(q2),2)*cos(q4)*sin(q1)*sin(q3) - 4*KUKA_LBR_param_.dblLink6InertZZ*cos(q2)*cos(q4)*sin(q2)*sin(q3) - 2*KUKA_LBR_param_.dblLink6InertXX*cos(q2)*cos(q4)*power(sin(q1),2)*sin(q2)*sin(q3) - 4*KUKA_LBR_param_.dblLink6InertYZ*cos(q4)*sin(q1)*power(sin(q2),2)*sin(q3) + KUKA_LBR_param_.dblLink6InertXX*cos(q4)*sin(2*q2)*sin(q3) + KUKA_LBR_param_.dblLink6InertYY*cos(q4)*sin(2*q2)*sin(q3) + KUKA_LBR_param_.dblLink6InertYY*cos(q4)*power(sin(q1),2)*sin(2*q2)*sin(q3) - 4*KUKA_LBR_param_.dblLink6InertXY*cos(q2)*power(cos(q3),2)*power(sin(q1),2)*sin(q4) + 4*KUKA_LBR_param_.dblLink6InertXZ*power(cos(q3),2)*sin(q1)*sin(q2)*sin(q4) + KUKA_LBR_param_.dblLink6InertXX*cos(q3)*sin(q3)*sin(q4) + KUKA_LBR_param_.dblLink6InertYY*cos(q3)*sin(q3)*sin(q4) - 2*KUKA_LBR_param_.dblLink6InertZZ*cos(q3)*sin(q3)*sin(q4) - KUKA_LBR_param_.dblLink6InertXX*power(cos(q2),2)*cos(q3)*sin(q3)*sin(q4) - KUKA_LBR_param_.dblLink6InertYY*power(cos(q2),2)*cos(q3)*sin(q3)*sin(q4) + 3*KUKA_LBR_param_.dblLink6InertXX*cos(q3)*power(sin(q1),2)*sin(q3)*sin(q4) - 3*KUKA_LBR_param_.dblLink6InertYY*cos(q3)*power(sin(q1),2)*sin(q3)*sin(q4) + KUKA_LBR_param_.dblLink6InertXX*power(cos(q2),2)*cos(q3)*power(sin(q1),2)*sin(q3)*sin(q4) - KUKA_LBR_param_.dblLink6InertYY*power(cos(q2),2)*cos(q3)*power(sin(q1),2)*sin(q3)*sin(q4) + 8*KUKA_LBR_param_.dblLink6InertYZ*cos(q2)*cos(q3)*sin(q1)*sin(q2)*sin(q3)*sin(q4) + KUKA_LBR_param_.dblLink6InertXX*cos(q3)*power(sin(q2),2)*sin(q3)*sin(q4) + KUKA_LBR_param_.dblLink6InertYY*cos(q3)*power(sin(q2),2)*sin(q3)*sin(q4) - 2*KUKA_LBR_param_.dblLink6InertZZ*cos(q3)*power(sin(q2),2)*sin(q3)*sin(q4) - KUKA_LBR_param_.dblLink6InertXX*cos(q3)*power(sin(q1),2)*power(sin(q2),2)*sin(q3)*sin(q4) + KUKA_LBR_param_.dblLink6InertYY*cos(q3)*power(sin(q1),2)*power(sin(q2),2)*sin(q3)*sin(q4) + 4*KUKA_LBR_param_.dblLink6InertXY*cos(q2)*power(sin(q1),2)*power(sin(q3),2)*sin(q4) - 4*KUKA_LBR_param_.dblLink6InertXZ*sin(q1)*sin(q2)*power(sin(q3),2)*sin(q4) + KUKA_LBR_param_.dblLink6InertZZ*power(cos(q2),2)*sin(2*q3)*sin(q4) - 3*KUKA_LBR_param_.dblLink6InertXY*sin(2*q1)*sin(2*q3)*sin(q4) + KUKA_LBR_param_.dblLink6InertXY*sin(2*q1)*power(sin(q2),2)*sin(2*q3)*sin(q4) + power(cos(q1),2)*(4*KUKA_LBR_param_.dblLink6InertXY*cos(q2)*power(cos(q3),2)*sin(q4) + cos(q3)*(-4*KUKA_LBR_param_.dblLink6InertXY*cos(q4)*sin(q2) - (KUKA_LBR_param_.dblLink6InertXX - KUKA_LBR_param_.dblLink6InertYY)*(3 + cos(2*q2))*sin(q3)*sin(q4)) + sin(q3)*(KUKA_LBR_param_.dblLink6InertXX*cos(q4)*sin(2*q2) - 2*cos(q2)*(KUKA_LBR_param_.dblLink6InertYY*cos(q4)*sin(q2) + 2*KUKA_LBR_param_.dblLink6InertXY*sin(q3)*sin(q4)))) - 4*cos(q1)*(power(cos(q2),2)*sin(q3)*(-(KUKA_LBR_param_.dblLink6InertXZ*cos(q4)) + KUKA_LBR_param_.dblLink6InertXY*cos(q3)*sin(q1)*sin(q4)) + sin(q2)*(-((KUKA_LBR_param_.dblLink6InertXX - KUKA_LBR_param_.dblLink6InertYY)*cos(q3)*cos(q4)*sin(q1)) + KUKA_LBR_param_.dblLink6InertYZ*power(cos(q3),2)*sin(q4) + sin(q3)*(KUKA_LBR_param_.dblLink6InertXZ*cos(q4)*sin(q2) - KUKA_LBR_param_.dblLink6InertYZ*sin(q3)*sin(q4))) + cos(q2)*((KUKA_LBR_param_.dblLink6InertXX - KUKA_LBR_param_.dblLink6InertYY)*power(cos(q3),2)*sin(q1)*sin(q4) + sin(q1)*sin(q3)*(-2*KUKA_LBR_param_.dblLink6InertXY*cos(q4)*sin(q2) + (-KUKA_LBR_param_.dblLink6InertXX + KUKA_LBR_param_.dblLink6InertYY)*sin(q3)*sin(q4)) + cos(q3)*(KUKA_LBR_param_.dblLink6InertYZ*cos(q4) - 2*KUKA_LBR_param_.dblLink6InertXZ*sin(q2)*sin(q3)*sin(q4)))) - 4*KUKA_LBR_param_.dblLink45Len*KUKA_LBR_param_.dblLink6CogX*KUKA_LBR_param_.dblLink6Mass*cos(q6)*sin(q5) - 4*KUKA_LBR_param_.dblLink6CogX*KUKA_LBR_param_.dblLink6CogY*KUKA_LBR_param_.dblLink6Mass*power(cos(q6),2)*sin(q5) + 4*KUKA_LBR_param_.dblLink45Len*KUKA_LBR_param_.dblLink6CogY*KUKA_LBR_param_.dblLink6Mass*sin(q5)*sin(q6) - 4*power(KUKA_LBR_param_.dblLink6CogX,2)*KUKA_LBR_param_.dblLink6Mass*cos(q6)*sin(q5)*sin(q6) + 4*power(KUKA_LBR_param_.dblLink6CogY,2)*KUKA_LBR_param_.dblLink6Mass*cos(q6)*sin(q5)*sin(q6) + 4*KUKA_LBR_param_.dblLink6CogX*KUKA_LBR_param_.dblLink6CogY*KUKA_LBR_param_.dblLink6Mass*sin(q5)*power(sin(q6),2) + 4*KUKA_LBR_param_.dblLink6CogZ*KUKA_LBR_param_.dblLink6Mass*cos(q5)*(KUKA_LBR_param_.dblLink45Len + KUKA_LBR_param_.dblLink6CogY*cos(q6) + KUKA_LBR_param_.dblLink6CogX*sin(q6)))/4.0 + KUKA_LBR_param_.dblLink7Mass*(cos(q5)*(KUKA_LBR_param_.dblLink7CogZ*sin(q2)*sin(q3)*sin(q6) + cos(q2)*sin(q4)*(KUKA_LBR_param_.dblLink7CogY*cos(q7) + KUKA_LBR_param_.dblLink7CogX*sin(q7)) - cos(q6)*sin(q2)*sin(q3)*(KUKA_LBR_param_.dblLink7CogX*cos(q7) - KUKA_LBR_param_.dblLink7CogY*sin(q7))) + sin(q5)*(cos(q7)*(KUKA_LBR_param_.dblLink7CogY*sin(q2)*sin(q3) + KUKA_LBR_param_.dblLink7CogX*cos(q2)*cos(q6)*sin(q4)) + KUKA_LBR_param_.dblLink7CogX*sin(q2)*sin(q3)*sin(q7) - cos(q2)*sin(q4)*(KUKA_LBR_param_.dblLink7CogZ*sin(q6) + KUKA_LBR_param_.dblLink7CogY*cos(q6)*sin(q7))) - cos(q3)*cos(q4)*sin(q2)*(cos(q5)*(KUKA_LBR_param_.dblLink7CogY*cos(q7) + KUKA_LBR_param_.dblLink7CogX*sin(q7)) - sin(q5)*(KUKA_LBR_param_.dblLink7CogZ*sin(q6) + cos(q6)*(-(KUKA_LBR_param_.dblLink7CogX*cos(q7)) + KUKA_LBR_param_.dblLink7CogY*sin(q7)))))*(cos(q2)*(-(sin(q4)*(KUKA_LBR_param_.dblLink45Len + KUKA_LBR_param_.dblLink7CogZ*cos(q6) + KUKA_LBR_param_.dblLink7CogX*cos(q7)*sin(q6) - KUKA_LBR_param_.dblLink7CogY*sin(q6)*sin(q7))) + cos(q4)*(sin(q5)*(KUKA_LBR_param_.dblLink7CogY*cos(q7) + KUKA_LBR_param_.dblLink7CogX*sin(q7)) + cos(q5)*(-(KUKA_LBR_param_.dblLink7CogX*cos(q6)*cos(q7)) + KUKA_LBR_param_.dblLink7CogZ*sin(q6) + KUKA_LBR_param_.dblLink7CogY*cos(q6)*sin(q7)))) + cos(q3)*sin(q2)*(cos(q4)*(KUKA_LBR_param_.dblLink45Len + KUKA_LBR_param_.dblLink7CogZ*cos(q6) + KUKA_LBR_param_.dblLink7CogX*cos(q7)*sin(q6) - KUKA_LBR_param_.dblLink7CogY*sin(q6)*sin(q7)) + sin(q4)*(sin(q5)*(KUKA_LBR_param_.dblLink7CogY*cos(q7) + KUKA_LBR_param_.dblLink7CogX*sin(q7)) + cos(q5)*(-(KUKA_LBR_param_.dblLink7CogX*cos(q6)*cos(q7)) + KUKA_LBR_param_.dblLink7CogZ*sin(q6) + KUKA_LBR_param_.dblLink7CogY*cos(q6)*sin(q7))))) + KUKA_LBR_param_.dblLink7Mass*(cos(q4)*(-(sin(q1)*sin(q2)*sin(q5)*(KUKA_LBR_param_.dblLink7CogY*cos(q7) + KUKA_LBR_param_.dblLink7CogX*sin(q7))) + cos(q1)*sin(q3)*(KUKA_LBR_param_.dblLink45Len + KUKA_LBR_param_.dblLink7CogZ*cos(q6) + KUKA_LBR_param_.dblLink7CogX*cos(q7)*sin(q6) - KUKA_LBR_param_.dblLink7CogY*sin(q6)*sin(q7)) - cos(q5)*sin(q1)*sin(q2)*(KUKA_LBR_param_.dblLink7CogZ*sin(q6) + cos(q6)*(-(KUKA_LBR_param_.dblLink7CogX*cos(q7)) + KUKA_LBR_param_.dblLink7CogY*sin(q7)))) + sin(q4)*(sin(q1)*sin(q2)*(KUKA_LBR_param_.dblLink45Len + KUKA_LBR_param_.dblLink7CogZ*cos(q6) + KUKA_LBR_param_.dblLink7CogX*cos(q7)*sin(q6) - KUKA_LBR_param_.dblLink7CogY*sin(q6)*sin(q7)) + cos(q1)*sin(q3)*(sin(q5)*(KUKA_LBR_param_.dblLink7CogY*cos(q7) + KUKA_LBR_param_.dblLink7CogX*sin(q7)) + cos(q5)*(-(KUKA_LBR_param_.dblLink7CogX*cos(q6)*cos(q7)) + KUKA_LBR_param_.dblLink7CogZ*sin(q6) + KUKA_LBR_param_.dblLink7CogY*cos(q6)*sin(q7)))) + cos(q2)*cos(q3)*sin(q1)*(cos(q4)*(KUKA_LBR_param_.dblLink45Len + KUKA_LBR_param_.dblLink7CogZ*cos(q6) + KUKA_LBR_param_.dblLink7CogX*cos(q7)*sin(q6) - KUKA_LBR_param_.dblLink7CogY*sin(q6)*sin(q7)) + sin(q4)*(sin(q5)*(KUKA_LBR_param_.dblLink7CogY*cos(q7) + KUKA_LBR_param_.dblLink7CogX*sin(q7)) + cos(q5)*(-(KUKA_LBR_param_.dblLink7CogX*cos(q6)*cos(q7)) + KUKA_LBR_param_.dblLink7CogZ*sin(q6) + KUKA_LBR_param_.dblLink7CogY*cos(q6)*sin(q7)))))*(cos(q1)*(-(cos(q4)*sin(q3)*(cos(q5)*(KUKA_LBR_param_.dblLink7CogY*cos(q7) + KUKA_LBR_param_.dblLink7CogX*sin(q7)) + sin(q5)*(KUKA_LBR_param_.dblLink7CogX*cos(q6)*cos(q7) - KUKA_LBR_param_.dblLink7CogZ*sin(q6) - KUKA_LBR_param_.dblLink7CogY*cos(q6)*sin(q7)))) - cos(q3)*(sin(q5)*(KUKA_LBR_param_.dblLink7CogY*cos(q7) + KUKA_LBR_param_.dblLink7CogX*sin(q7)) + cos(q5)*(-(KUKA_LBR_param_.dblLink7CogX*cos(q6)*cos(q7)) + KUKA_LBR_param_.dblLink7CogZ*sin(q6) + KUKA_LBR_param_.dblLink7CogY*cos(q6)*sin(q7)))) + sin(q1)*(-(sin(q2)*sin(q4)*(cos(q5)*(KUKA_LBR_param_.dblLink7CogY*cos(q7) + KUKA_LBR_param_.dblLink7CogX*sin(q7)) + sin(q5)*(KUKA_LBR_param_.dblLink7CogX*cos(q6)*cos(q7) - KUKA_LBR_param_.dblLink7CogZ*sin(q6) - KUKA_LBR_param_.dblLink7CogY*cos(q6)*sin(q7)))) + cos(q2)*(-(cos(q3)*cos(q4)*(cos(q5)*(KUKA_LBR_param_.dblLink7CogY*cos(q7) + KUKA_LBR_param_.dblLink7CogX*sin(q7)) + sin(q5)*(KUKA_LBR_param_.dblLink7CogX*cos(q6)*cos(q7) - KUKA_LBR_param_.dblLink7CogZ*sin(q6) - KUKA_LBR_param_.dblLink7CogY*cos(q6)*sin(q7)))) + sin(q3)*(sin(q5)*(KUKA_LBR_param_.dblLink7CogY*cos(q7) + KUKA_LBR_param_.dblLink7CogX*sin(q7)) + cos(q5)*(-(KUKA_LBR_param_.dblLink7CogX*cos(q6)*cos(q7)) + KUKA_LBR_param_.dblLink7CogZ*sin(q6) + KUKA_LBR_param_.dblLink7CogY*cos(q6)*sin(q7)))))) + KUKA_LBR_param_.dblLink7Mass*(sin(q1)*(-(cos(q4)*sin(q3)*(cos(q5)*(KUKA_LBR_param_.dblLink7CogY*cos(q7) + KUKA_LBR_param_.dblLink7CogX*sin(q7)) + sin(q5)*(KUKA_LBR_param_.dblLink7CogX*cos(q6)*cos(q7) - KUKA_LBR_param_.dblLink7CogZ*sin(q6) - KUKA_LBR_param_.dblLink7CogY*cos(q6)*sin(q7)))) - cos(q3)*(sin(q5)*(KUKA_LBR_param_.dblLink7CogY*cos(q7) + KUKA_LBR_param_.dblLink7CogX*sin(q7)) + cos(q5)*(-(KUKA_LBR_param_.dblLink7CogX*cos(q6)*cos(q7)) + KUKA_LBR_param_.dblLink7CogZ*sin(q6) + KUKA_LBR_param_.dblLink7CogY*cos(q6)*sin(q7)))) + cos(q1)*(sin(q2)*sin(q4)*(cos(q5)*(KUKA_LBR_param_.dblLink7CogY*cos(q7) + KUKA_LBR_param_.dblLink7CogX*sin(q7)) + sin(q5)*(KUKA_LBR_param_.dblLink7CogX*cos(q6)*cos(q7) - KUKA_LBR_param_.dblLink7CogZ*sin(q6) - KUKA_LBR_param_.dblLink7CogY*cos(q6)*sin(q7))) + cos(q2)*(cos(q3)*cos(q4)*(cos(q5)*(KUKA_LBR_param_.dblLink7CogY*cos(q7) + KUKA_LBR_param_.dblLink7CogX*sin(q7)) + sin(q5)*(KUKA_LBR_param_.dblLink7CogX*cos(q6)*cos(q7) - KUKA_LBR_param_.dblLink7CogZ*sin(q6) - KUKA_LBR_param_.dblLink7CogY*cos(q6)*sin(q7))) - sin(q3)*(sin(q5)*(KUKA_LBR_param_.dblLink7CogY*cos(q7) + KUKA_LBR_param_.dblLink7CogX*sin(q7)) + cos(q5)*(-(KUKA_LBR_param_.dblLink7CogX*cos(q6)*cos(q7)) + KUKA_LBR_param_.dblLink7CogZ*sin(q6) + KUKA_LBR_param_.dblLink7CogY*cos(q6)*sin(q7))))))*(sin(q1)*sin(q3)*(cos(q4)*(KUKA_LBR_param_.dblLink45Len + KUKA_LBR_param_.dblLink7CogZ*cos(q6) + KUKA_LBR_param_.dblLink7CogX*cos(q7)*sin(q6) - KUKA_LBR_param_.dblLink7CogY*sin(q6)*sin(q7)) + sin(q4)*(sin(q5)*(KUKA_LBR_param_.dblLink7CogY*cos(q7) + KUKA_LBR_param_.dblLink7CogX*sin(q7)) + cos(q5)*(-(KUKA_LBR_param_.dblLink7CogX*cos(q6)*cos(q7)) + KUKA_LBR_param_.dblLink7CogZ*sin(q6) + KUKA_LBR_param_.dblLink7CogY*cos(q6)*sin(q7)))) - cos(q1)*(sin(q2)*(sin(q4)*(KUKA_LBR_param_.dblLink45Len + KUKA_LBR_param_.dblLink7CogZ*cos(q6) + KUKA_LBR_param_.dblLink7CogX*cos(q7)*sin(q6) - KUKA_LBR_param_.dblLink7CogY*sin(q6)*sin(q7)) - cos(q4)*(sin(q5)*(KUKA_LBR_param_.dblLink7CogY*cos(q7) + KUKA_LBR_param_.dblLink7CogX*sin(q7)) + cos(q5)*(-(KUKA_LBR_param_.dblLink7CogX*cos(q6)*cos(q7)) + KUKA_LBR_param_.dblLink7CogZ*sin(q6) + KUKA_LBR_param_.dblLink7CogY*cos(q6)*sin(q7)))) + cos(q2)*cos(q3)*(cos(q4)*(KUKA_LBR_param_.dblLink45Len + KUKA_LBR_param_.dblLink7CogZ*cos(q6) + KUKA_LBR_param_.dblLink7CogX*cos(q7)*sin(q6) - KUKA_LBR_param_.dblLink7CogY*sin(q6)*sin(q7)) + sin(q4)*(sin(q5)*(KUKA_LBR_param_.dblLink7CogY*cos(q7) + KUKA_LBR_param_.dblLink7CogX*sin(q7)) + cos(q5)*(-(KUKA_LBR_param_.dblLink7CogX*cos(q6)*cos(q7)) + KUKA_LBR_param_.dblLink7CogZ*sin(q6) + KUKA_LBR_param_.dblLink7CogY*cos(q6)*sin(q7))))));
dblMassInertFullRow5Col5 = (sin(q1)*sin(q3)*sin(q4) + cos(q1)*(cos(q4)*sin(q2) - cos(q2)*cos(q3)*sin(q4)))*(KUKA_LBR_param_.dblLink5InertXY*cos(q4)*sin(q1)*sin(q2) + KUKA_LBR_param_.dblLink5InertXZ*cos(q3)*sin(q2)*sin(q4) + KUKA_LBR_param_.dblLink5InertXX*sin(q1)*sin(q3)*sin(q4) + cos(q2)*(KUKA_LBR_param_.dblLink5InertXZ*cos(q4) - cos(q3)*(KUKA_LBR_param_.dblLink5InertXX*cos(q1) + KUKA_LBR_param_.dblLink5InertXY*sin(q1))*sin(q4)) + cos(q1)*(KUKA_LBR_param_.dblLink5InertXX*cos(q4)*sin(q2) - KUKA_LBR_param_.dblLink5InertXY*sin(q3)*sin(q4))) + (cos(q4)*sin(q1)*sin(q2) - (cos(q2)*cos(q3)*sin(q1) + cos(q1)*sin(q3))*sin(q4))*(KUKA_LBR_param_.dblLink5InertYY*cos(q4)*sin(q1)*sin(q2) + KUKA_LBR_param_.dblLink5InertYZ*cos(q3)*sin(q2)*sin(q4) + KUKA_LBR_param_.dblLink5InertXY*sin(q1)*sin(q3)*sin(q4) + cos(q2)*(KUKA_LBR_param_.dblLink5InertYZ*cos(q4) - cos(q3)*(KUKA_LBR_param_.dblLink5InertXY*cos(q1) + KUKA_LBR_param_.dblLink5InertYY*sin(q1))*sin(q4)) + cos(q1)*(KUKA_LBR_param_.dblLink5InertXY*cos(q4)*sin(q2) - KUKA_LBR_param_.dblLink5InertYY*sin(q3)*sin(q4))) + (cos(q2)*cos(q4) + cos(q3)*sin(q2)*sin(q4))*(KUKA_LBR_param_.dblLink5InertYZ*cos(q4)*sin(q1)*sin(q2) + KUKA_LBR_param_.dblLink5InertZZ*cos(q3)*sin(q2)*sin(q4) + KUKA_LBR_param_.dblLink5InertXZ*sin(q1)*sin(q3)*sin(q4) + cos(q2)*(KUKA_LBR_param_.dblLink5InertZZ*cos(q4) - cos(q3)*(KUKA_LBR_param_.dblLink5InertXZ*cos(q1) + KUKA_LBR_param_.dblLink5InertYZ*sin(q1))*sin(q4)) + cos(q1)*(KUKA_LBR_param_.dblLink5InertXZ*cos(q4)*sin(q2) - KUKA_LBR_param_.dblLink5InertYZ*sin(q3)*sin(q4))) + (sin(q1)*sin(q3)*sin(q4) + cos(q1)*(cos(q4)*sin(q2) - cos(q2)*cos(q3)*sin(q4)))*(KUKA_LBR_param_.dblLink6InertXY*cos(q4)*sin(q1)*sin(q2) + KUKA_LBR_param_.dblLink6InertXZ*cos(q3)*sin(q2)*sin(q4) + KUKA_LBR_param_.dblLink6InertXX*sin(q1)*sin(q3)*sin(q4) + cos(q2)*(KUKA_LBR_param_.dblLink6InertXZ*cos(q4) - cos(q3)*(KUKA_LBR_param_.dblLink6InertXX*cos(q1) + KUKA_LBR_param_.dblLink6InertXY*sin(q1))*sin(q4)) + cos(q1)*(KUKA_LBR_param_.dblLink6InertXX*cos(q4)*sin(q2) - KUKA_LBR_param_.dblLink6InertXY*sin(q3)*sin(q4))) + (cos(q4)*sin(q1)*sin(q2) - (cos(q2)*cos(q3)*sin(q1) + cos(q1)*sin(q3))*sin(q4))*(KUKA_LBR_param_.dblLink6InertYY*cos(q4)*sin(q1)*sin(q2) + KUKA_LBR_param_.dblLink6InertYZ*cos(q3)*sin(q2)*sin(q4) + KUKA_LBR_param_.dblLink6InertXY*sin(q1)*sin(q3)*sin(q4) + cos(q2)*(KUKA_LBR_param_.dblLink6InertYZ*cos(q4) - cos(q3)*(KUKA_LBR_param_.dblLink6InertXY*cos(q1) + KUKA_LBR_param_.dblLink6InertYY*sin(q1))*sin(q4)) + cos(q1)*(KUKA_LBR_param_.dblLink6InertXY*cos(q4)*sin(q2) - KUKA_LBR_param_.dblLink6InertYY*sin(q3)*sin(q4))) + (cos(q2)*cos(q4) + cos(q3)*sin(q2)*sin(q4))*(KUKA_LBR_param_.dblLink6InertYZ*cos(q4)*sin(q1)*sin(q2) + KUKA_LBR_param_.dblLink6InertZZ*cos(q3)*sin(q2)*sin(q4) + KUKA_LBR_param_.dblLink6InertXZ*sin(q1)*sin(q3)*sin(q4) + cos(q2)*(KUKA_LBR_param_.dblLink6InertZZ*cos(q4) - cos(q3)*(KUKA_LBR_param_.dblLink6InertXZ*cos(q1) + KUKA_LBR_param_.dblLink6InertYZ*sin(q1))*sin(q4)) + cos(q1)*(KUKA_LBR_param_.dblLink6InertXZ*cos(q4)*sin(q2) - KUKA_LBR_param_.dblLink6InertYZ*sin(q3)*sin(q4))) + (sin(q1)*sin(q3)*sin(q4) + cos(q1)*(cos(q4)*sin(q2) - cos(q2)*cos(q3)*sin(q4)))*(KUKA_LBR_param_.dblLink7InertXY*cos(q4)*sin(q1)*sin(q2) + KUKA_LBR_param_.dblLink7InertXZ*cos(q3)*sin(q2)*sin(q4) + KUKA_LBR_param_.dblLink7InertXX*sin(q1)*sin(q3)*sin(q4) + cos(q2)*(KUKA_LBR_param_.dblLink7InertXZ*cos(q4) - cos(q3)*(KUKA_LBR_param_.dblLink7InertXX*cos(q1) + KUKA_LBR_param_.dblLink7InertXY*sin(q1))*sin(q4)) + cos(q1)*(KUKA_LBR_param_.dblLink7InertXX*cos(q4)*sin(q2) - KUKA_LBR_param_.dblLink7InertXY*sin(q3)*sin(q4))) + (cos(q4)*sin(q1)*sin(q2) - (cos(q2)*cos(q3)*sin(q1) + cos(q1)*sin(q3))*sin(q4))*(KUKA_LBR_param_.dblLink7InertYY*cos(q4)*sin(q1)*sin(q2) + KUKA_LBR_param_.dblLink7InertYZ*cos(q3)*sin(q2)*sin(q4) + KUKA_LBR_param_.dblLink7InertXY*sin(q1)*sin(q3)*sin(q4) + cos(q2)*(KUKA_LBR_param_.dblLink7InertYZ*cos(q4) - cos(q3)*(KUKA_LBR_param_.dblLink7InertXY*cos(q1) + KUKA_LBR_param_.dblLink7InertYY*sin(q1))*sin(q4)) + cos(q1)*(KUKA_LBR_param_.dblLink7InertXY*cos(q4)*sin(q2) - KUKA_LBR_param_.dblLink7InertYY*sin(q3)*sin(q4))) + (cos(q2)*cos(q4) + cos(q3)*sin(q2)*sin(q4))*(KUKA_LBR_param_.dblLink7InertYZ*cos(q4)*sin(q1)*sin(q2) + KUKA_LBR_param_.dblLink7InertZZ*cos(q3)*sin(q2)*sin(q4) + KUKA_LBR_param_.dblLink7InertXZ*sin(q1)*sin(q3)*sin(q4) + cos(q2)*(KUKA_LBR_param_.dblLink7InertZZ*cos(q4) - cos(q3)*(KUKA_LBR_param_.dblLink7InertXZ*cos(q1) + KUKA_LBR_param_.dblLink7InertYZ*sin(q1))*sin(q4)) + cos(q1)*(KUKA_LBR_param_.dblLink7InertXZ*cos(q4)*sin(q2) - KUKA_LBR_param_.dblLink7InertYZ*sin(q3)*sin(q4))) + KUKA_LBR_param_.dblLink5Mass*power(cos(q5)*(-(KUKA_LBR_param_.dblLink5CogX*sin(q2)*sin(q3)) + KUKA_LBR_param_.dblLink5CogY*cos(q2)*sin(q4)) + (KUKA_LBR_param_.dblLink5CogY*sin(q2)*sin(q3) + KUKA_LBR_param_.dblLink5CogX*cos(q2)*sin(q4))*sin(q5) - cos(q3)*cos(q4)*sin(q2)*(KUKA_LBR_param_.dblLink5CogY*cos(q5) + KUKA_LBR_param_.dblLink5CogX*sin(q5)),2) + KUKA_LBR_param_.dblLink5Mass*power(sin(q1)*(-(cos(q4)*sin(q3)*(KUKA_LBR_param_.dblLink5CogY*cos(q5) + KUKA_LBR_param_.dblLink5CogX*sin(q5))) + cos(q3)*(KUKA_LBR_param_.dblLink5CogX*cos(q5) - KUKA_LBR_param_.dblLink5CogY*sin(q5))) + cos(q1)*(sin(q2)*sin(q4)*(KUKA_LBR_param_.dblLink5CogY*cos(q5) + KUKA_LBR_param_.dblLink5CogX*sin(q5)) + cos(q2)*(cos(q3)*cos(q4)*(KUKA_LBR_param_.dblLink5CogY*cos(q5) + KUKA_LBR_param_.dblLink5CogX*sin(q5)) + sin(q3)*(KUKA_LBR_param_.dblLink5CogX*cos(q5) - KUKA_LBR_param_.dblLink5CogY*sin(q5)))),2) + KUKA_LBR_param_.dblLink5Mass*power(cos(q1)*(cos(q4)*sin(q3)*(KUKA_LBR_param_.dblLink5CogY*cos(q5) + KUKA_LBR_param_.dblLink5CogX*sin(q5)) + cos(q3)*(-(KUKA_LBR_param_.dblLink5CogX*cos(q5)) + KUKA_LBR_param_.dblLink5CogY*sin(q5))) + sin(q1)*(sin(q2)*sin(q4)*(KUKA_LBR_param_.dblLink5CogY*cos(q5) + KUKA_LBR_param_.dblLink5CogX*sin(q5)) + cos(q2)*(cos(q3)*cos(q4)*(KUKA_LBR_param_.dblLink5CogY*cos(q5) + KUKA_LBR_param_.dblLink5CogX*sin(q5)) + sin(q3)*(KUKA_LBR_param_.dblLink5CogX*cos(q5) - KUKA_LBR_param_.dblLink5CogY*sin(q5)))),2) + KUKA_LBR_param_.dblLink6Mass*power(cos(q5)*(KUKA_LBR_param_.dblLink6CogX*cos(q6)*sin(q2)*sin(q3) + KUKA_LBR_param_.dblLink6CogZ*cos(q2)*sin(q4) - KUKA_LBR_param_.dblLink6CogY*sin(q2)*sin(q3)*sin(q6)) + sin(q5)*(KUKA_LBR_param_.dblLink6CogZ*sin(q2)*sin(q3) + cos(q2)*sin(q4)*(-(KUKA_LBR_param_.dblLink6CogX*cos(q6)) + KUKA_LBR_param_.dblLink6CogY*sin(q6))) - cos(q3)*cos(q4)*sin(q2)*(KUKA_LBR_param_.dblLink6CogZ*cos(q5) + sin(q5)*(-(KUKA_LBR_param_.dblLink6CogX*cos(q6)) + KUKA_LBR_param_.dblLink6CogY*sin(q6))),2) + KUKA_LBR_param_.dblLink6Mass*power(sin(q1)*(cos(q3)*(KUKA_LBR_param_.dblLink6CogX*cos(q5)*cos(q6) + KUKA_LBR_param_.dblLink6CogZ*sin(q5) - KUKA_LBR_param_.dblLink6CogY*cos(q5)*sin(q6)) + cos(q4)*sin(q3)*(KUKA_LBR_param_.dblLink6CogZ*cos(q5) - KUKA_LBR_param_.dblLink6CogX*cos(q6)*sin(q5) + KUKA_LBR_param_.dblLink6CogY*sin(q5)*sin(q6))) - cos(q1)*(sin(q2)*sin(q4)*(KUKA_LBR_param_.dblLink6CogZ*cos(q5) + sin(q5)*(-(KUKA_LBR_param_.dblLink6CogX*cos(q6)) + KUKA_LBR_param_.dblLink6CogY*sin(q6))) + cos(q2)*(-(sin(q3)*(KUKA_LBR_param_.dblLink6CogX*cos(q5)*cos(q6) + KUKA_LBR_param_.dblLink6CogZ*sin(q5) - KUKA_LBR_param_.dblLink6CogY*cos(q5)*sin(q6))) + cos(q3)*cos(q4)*(KUKA_LBR_param_.dblLink6CogZ*cos(q5) - KUKA_LBR_param_.dblLink6CogX*cos(q6)*sin(q5) + KUKA_LBR_param_.dblLink6CogY*sin(q5)*sin(q6)))),2) + KUKA_LBR_param_.dblLink6Mass*power(cos(q1)*(cos(q3)*(KUKA_LBR_param_.dblLink6CogX*cos(q5)*cos(q6) + KUKA_LBR_param_.dblLink6CogZ*sin(q5) - KUKA_LBR_param_.dblLink6CogY*cos(q5)*sin(q6)) + cos(q4)*sin(q3)*(KUKA_LBR_param_.dblLink6CogZ*cos(q5) - KUKA_LBR_param_.dblLink6CogX*cos(q6)*sin(q5) + KUKA_LBR_param_.dblLink6CogY*sin(q5)*sin(q6))) + sin(q1)*(sin(q2)*sin(q4)*(KUKA_LBR_param_.dblLink6CogZ*cos(q5) + sin(q5)*(-(KUKA_LBR_param_.dblLink6CogX*cos(q6)) + KUKA_LBR_param_.dblLink6CogY*sin(q6))) + cos(q2)*(-(sin(q3)*(KUKA_LBR_param_.dblLink6CogX*cos(q5)*cos(q6) + KUKA_LBR_param_.dblLink6CogZ*sin(q5) - KUKA_LBR_param_.dblLink6CogY*cos(q5)*sin(q6))) + cos(q3)*cos(q4)*(KUKA_LBR_param_.dblLink6CogZ*cos(q5) - KUKA_LBR_param_.dblLink6CogX*cos(q6)*sin(q5) + KUKA_LBR_param_.dblLink6CogY*sin(q5)*sin(q6)))),2) + KUKA_LBR_param_.dblLink7Mass*power(cos(q5)*(KUKA_LBR_param_.dblLink7CogZ*sin(q2)*sin(q3)*sin(q6) + cos(q2)*sin(q4)*(KUKA_LBR_param_.dblLink7CogY*cos(q7) + KUKA_LBR_param_.dblLink7CogX*sin(q7)) - cos(q6)*sin(q2)*sin(q3)*(KUKA_LBR_param_.dblLink7CogX*cos(q7) - KUKA_LBR_param_.dblLink7CogY*sin(q7))) + sin(q5)*(cos(q7)*(KUKA_LBR_param_.dblLink7CogY*sin(q2)*sin(q3) + KUKA_LBR_param_.dblLink7CogX*cos(q2)*cos(q6)*sin(q4)) + KUKA_LBR_param_.dblLink7CogX*sin(q2)*sin(q3)*sin(q7) - cos(q2)*sin(q4)*(KUKA_LBR_param_.dblLink7CogZ*sin(q6) + KUKA_LBR_param_.dblLink7CogY*cos(q6)*sin(q7))) - cos(q3)*cos(q4)*sin(q2)*(cos(q5)*(KUKA_LBR_param_.dblLink7CogY*cos(q7) + KUKA_LBR_param_.dblLink7CogX*sin(q7)) - sin(q5)*(KUKA_LBR_param_.dblLink7CogZ*sin(q6) + cos(q6)*(-(KUKA_LBR_param_.dblLink7CogX*cos(q7)) + KUKA_LBR_param_.dblLink7CogY*sin(q7)))),2) + KUKA_LBR_param_.dblLink7Mass*power(sin(q1)*(-(cos(q4)*sin(q3)*(cos(q5)*(KUKA_LBR_param_.dblLink7CogY*cos(q7) + KUKA_LBR_param_.dblLink7CogX*sin(q7)) + sin(q5)*(KUKA_LBR_param_.dblLink7CogX*cos(q6)*cos(q7) - KUKA_LBR_param_.dblLink7CogZ*sin(q6) - KUKA_LBR_param_.dblLink7CogY*cos(q6)*sin(q7)))) - cos(q3)*(sin(q5)*(KUKA_LBR_param_.dblLink7CogY*cos(q7) + KUKA_LBR_param_.dblLink7CogX*sin(q7)) + cos(q5)*(-(KUKA_LBR_param_.dblLink7CogX*cos(q6)*cos(q7)) + KUKA_LBR_param_.dblLink7CogZ*sin(q6) + KUKA_LBR_param_.dblLink7CogY*cos(q6)*sin(q7)))) + cos(q1)*(sin(q2)*sin(q4)*(cos(q5)*(KUKA_LBR_param_.dblLink7CogY*cos(q7) + KUKA_LBR_param_.dblLink7CogX*sin(q7)) + sin(q5)*(KUKA_LBR_param_.dblLink7CogX*cos(q6)*cos(q7) - KUKA_LBR_param_.dblLink7CogZ*sin(q6) - KUKA_LBR_param_.dblLink7CogY*cos(q6)*sin(q7))) + cos(q2)*(cos(q3)*cos(q4)*(cos(q5)*(KUKA_LBR_param_.dblLink7CogY*cos(q7) + KUKA_LBR_param_.dblLink7CogX*sin(q7)) + sin(q5)*(KUKA_LBR_param_.dblLink7CogX*cos(q6)*cos(q7) - KUKA_LBR_param_.dblLink7CogZ*sin(q6) - KUKA_LBR_param_.dblLink7CogY*cos(q6)*sin(q7))) - sin(q3)*(sin(q5)*(KUKA_LBR_param_.dblLink7CogY*cos(q7) + KUKA_LBR_param_.dblLink7CogX*sin(q7)) + cos(q5)*(-(KUKA_LBR_param_.dblLink7CogX*cos(q6)*cos(q7)) + KUKA_LBR_param_.dblLink7CogZ*sin(q6) + KUKA_LBR_param_.dblLink7CogY*cos(q6)*sin(q7))))),2) + KUKA_LBR_param_.dblLink7Mass*power(cos(q1)*(cos(q4)*sin(q3)*(cos(q5)*(KUKA_LBR_param_.dblLink7CogY*cos(q7) + KUKA_LBR_param_.dblLink7CogX*sin(q7)) + sin(q5)*(KUKA_LBR_param_.dblLink7CogX*cos(q6)*cos(q7) - KUKA_LBR_param_.dblLink7CogZ*sin(q6) - KUKA_LBR_param_.dblLink7CogY*cos(q6)*sin(q7))) + cos(q3)*(sin(q5)*(KUKA_LBR_param_.dblLink7CogY*cos(q7) + KUKA_LBR_param_.dblLink7CogX*sin(q7)) + cos(q5)*(-(KUKA_LBR_param_.dblLink7CogX*cos(q6)*cos(q7)) + KUKA_LBR_param_.dblLink7CogZ*sin(q6) + KUKA_LBR_param_.dblLink7CogY*cos(q6)*sin(q7)))) + sin(q1)*(sin(q2)*sin(q4)*(cos(q5)*(KUKA_LBR_param_.dblLink7CogY*cos(q7) + KUKA_LBR_param_.dblLink7CogX*sin(q7)) + sin(q5)*(KUKA_LBR_param_.dblLink7CogX*cos(q6)*cos(q7) - KUKA_LBR_param_.dblLink7CogZ*sin(q6) - KUKA_LBR_param_.dblLink7CogY*cos(q6)*sin(q7))) + cos(q2)*(cos(q3)*cos(q4)*(cos(q5)*(KUKA_LBR_param_.dblLink7CogY*cos(q7) + KUKA_LBR_param_.dblLink7CogX*sin(q7)) + sin(q5)*(KUKA_LBR_param_.dblLink7CogX*cos(q6)*cos(q7) - KUKA_LBR_param_.dblLink7CogZ*sin(q6) - KUKA_LBR_param_.dblLink7CogY*cos(q6)*sin(q7))) - sin(q3)*(sin(q5)*(KUKA_LBR_param_.dblLink7CogY*cos(q7) + KUKA_LBR_param_.dblLink7CogX*sin(q7)) + cos(q5)*(-(KUKA_LBR_param_.dblLink7CogX*cos(q6)*cos(q7)) + KUKA_LBR_param_.dblLink7CogZ*sin(q6) + KUKA_LBR_param_.dblLink7CogY*cos(q6)*sin(q7))))),2);
dblMassInertFullRow5Col6 = (KUKA_LBR_param_.dblLink7InertYZ*cos(q4)*sin(q1)*sin(q2) + KUKA_LBR_param_.dblLink7InertZZ*cos(q3)*sin(q2)*sin(q4) + KUKA_LBR_param_.dblLink7InertXZ*sin(q1)*sin(q3)*sin(q4) + cos(q2)*(KUKA_LBR_param_.dblLink7InertZZ*cos(q4) - cos(q3)*(KUKA_LBR_param_.dblLink7InertXZ*cos(q1) + KUKA_LBR_param_.dblLink7InertYZ*sin(q1))*sin(q4)) + cos(q1)*(KUKA_LBR_param_.dblLink7InertXZ*cos(q4)*sin(q2) - KUKA_LBR_param_.dblLink7InertYZ*sin(q3)*sin(q4)))*(cos(q5)*sin(q2)*sin(q3) + (cos(q3)*cos(q4)*sin(q2) - cos(q2)*sin(q4))*sin(q5)) + (KUKA_LBR_param_.dblLink7InertXY*cos(q4)*sin(q1)*sin(q2) + KUKA_LBR_param_.dblLink7InertXZ*cos(q3)*sin(q2)*sin(q4) + KUKA_LBR_param_.dblLink7InertXX*sin(q1)*sin(q3)*sin(q4) + cos(q2)*(KUKA_LBR_param_.dblLink7InertXZ*cos(q4) - cos(q3)*(KUKA_LBR_param_.dblLink7InertXX*cos(q1) + KUKA_LBR_param_.dblLink7InertXY*sin(q1))*sin(q4)) + cos(q1)*(KUKA_LBR_param_.dblLink7InertXX*cos(q4)*sin(q2) - KUKA_LBR_param_.dblLink7InertXY*sin(q3)*sin(q4)))*(-(cos(q5)*(cos(q3)*sin(q1) + cos(q1)*cos(q2)*sin(q3))) + (cos(q4)*sin(q1)*sin(q3) - cos(q1)*(cos(q2)*cos(q3)*cos(q4) + sin(q2)*sin(q4)))*sin(q5)) + (KUKA_LBR_param_.dblLink7InertYY*cos(q4)*sin(q1)*sin(q2) + KUKA_LBR_param_.dblLink7InertYZ*cos(q3)*sin(q2)*sin(q4) + KUKA_LBR_param_.dblLink7InertXY*sin(q1)*sin(q3)*sin(q4) + cos(q2)*(KUKA_LBR_param_.dblLink7InertYZ*cos(q4) - cos(q3)*(KUKA_LBR_param_.dblLink7InertXY*cos(q1) + KUKA_LBR_param_.dblLink7InertYY*sin(q1))*sin(q4)) + cos(q1)*(KUKA_LBR_param_.dblLink7InertXY*cos(q4)*sin(q2) - KUKA_LBR_param_.dblLink7InertYY*sin(q3)*sin(q4)))*(cos(q1)*(cos(q3)*cos(q5) - cos(q4)*sin(q3)*sin(q5)) - sin(q1)*(sin(q2)*sin(q4)*sin(q5) + cos(q2)*(cos(q5)*sin(q3) + cos(q3)*cos(q4)*sin(q5)))) + (power(cos(q1),2)*(32*KUKA_LBR_param_.dblLink6InertXY*cos(q2)*cos(q5)*power(sin(q3),2)*sin(q4) + 10*KUKA_LBR_param_.dblLink6InertXX*cos(q5)*sin(2*q3)*sin(q4) - 14*KUKA_LBR_param_.dblLink6InertYY*cos(q5)*sin(2*q3)*sin(q4) + 4*KUKA_LBR_param_.dblLink6InertXX*power(cos(q2),2)*cos(q5)*sin(2*q3)*sin(q4) + 2*KUKA_LBR_param_.dblLink6InertXX*cos(2*q2)*cos(q5)*sin(2*q3)*sin(q4) - 2*KUKA_LBR_param_.dblLink6InertYY*cos(2*q2)*cos(q5)*sin(2*q3)*sin(q4) + 4*KUKA_LBR_param_.dblLink6InertYY*cos(q5)*power(sin(q2),2)*sin(2*q3)*sin(q4) - 32*KUKA_LBR_param_.dblLink6InertXY*power(cos(q4),2)*sin(q2)*sin(q3)*sin(q5) + 32*KUKA_LBR_param_.dblLink6InertXY*sin(q2)*sin(q3)*power(sin(q4),2)*sin(q5) - 6*KUKA_LBR_param_.dblLink6InertXX*sin(2*q4)*sin(q5) + 6*KUKA_LBR_param_.dblLink6InertYY*sin(2*q4)*sin(q5) + 5*KUKA_LBR_param_.dblLink6InertXX*power(cos(q2),2)*sin(2*q4)*sin(q5) - 5*KUKA_LBR_param_.dblLink6InertYY*power(cos(q2),2)*sin(2*q4)*sin(q5) + KUKA_LBR_param_.dblLink6InertXX*power(cos(q2),2)*cos(2*q3)*sin(2*q4)*sin(q5) - KUKA_LBR_param_.dblLink6InertYY*power(cos(q2),2)*cos(2*q3)*sin(2*q4)*sin(q5) - 6*KUKA_LBR_param_.dblLink6InertXX*power(sin(q2),2)*sin(2*q4)*sin(q5) + 6*KUKA_LBR_param_.dblLink6InertYY*power(sin(q2),2)*sin(2*q4)*sin(q5) - 6*KUKA_LBR_param_.dblLink6InertXX*power(sin(q3),2)*sin(2*q4)*sin(q5) + 6*KUKA_LBR_param_.dblLink6InertYY*power(sin(q3),2)*sin(2*q4)*sin(q5) - 2*KUKA_LBR_param_.dblLink6InertYY*power(sin(q2),2)*power(sin(q3),2)*sin(2*q4)*sin(q5) + 16*KUKA_LBR_param_.dblLink6InertXY*cos(q2)*sin(2*q3)*sin(2*q4)*sin(q5) - 2*power(cos(q3),2)*sin(q4)*(16*KUKA_LBR_param_.dblLink6InertXY*cos(q2)*cos(q5) - 2*(KUKA_LBR_param_.dblLink6InertXX - KUKA_LBR_param_.dblLink6InertYY)*power(cos(q2),2)*cos(q4)*sin(q5) - (KUKA_LBR_param_.dblLink6InertXX - KUKA_LBR_param_.dblLink6InertYY)*(5 + cos(2*q2))*cos(q4)*sin(q5)) + 4*cos(q4)*sin(q3)*(-2*(KUKA_LBR_param_.dblLink6InertXX - KUKA_LBR_param_.dblLink6InertYY)*cos(q5)*sin(2*q2) + KUKA_LBR_param_.dblLink6InertXX*power(sin(q2),2)*sin(q3)*sin(q4)*sin(q5)) + 8*cos(q3)*(4*KUKA_LBR_param_.dblLink6InertXY*cos(q4)*cos(q5)*sin(q2) - (KUKA_LBR_param_.dblLink6InertXX - KUKA_LBR_param_.dblLink6InertYY)*power(cos(q4),2)*sin(2*q2)*sin(q5) + (KUKA_LBR_param_.dblLink6InertXX - KUKA_LBR_param_.dblLink6InertYY)*sin(2*q2)*power(sin(q4),2)*sin(q5))) + 8*cos(q1)*(4*KUKA_LBR_param_.dblLink6InertXZ*cos(q4)*cos(q5)*power(sin(q2),2)*sin(q3) + 4*KUKA_LBR_param_.dblLink6InertYZ*power(cos(q3),2)*cos(q5)*sin(q2)*sin(q4) - 4*KUKA_LBR_param_.dblLink6InertYZ*cos(q5)*sin(q2)*power(sin(q3),2)*sin(q4) - 2*KUKA_LBR_param_.dblLink6InertXZ*cos(q5)*sin(2*q2)*sin(2*q3)*sin(q4) + 4*KUKA_LBR_param_.dblLink6InertXX*power(cos(q4),2)*sin(q1)*sin(q2)*sin(q3)*sin(q5) - 4*KUKA_LBR_param_.dblLink6InertYY*power(cos(q4),2)*sin(q1)*sin(q2)*sin(q3)*sin(q5) - 4*KUKA_LBR_param_.dblLink6InertXX*sin(q1)*sin(q2)*sin(q3)*power(sin(q4),2)*sin(q5) + 4*KUKA_LBR_param_.dblLink6InertYY*sin(q1)*sin(q2)*sin(q3)*power(sin(q4),2)*sin(q5) - 3*KUKA_LBR_param_.dblLink6InertXZ*sin(2*q2)*sin(2*q4)*sin(q5) + KUKA_LBR_param_.dblLink6InertXZ*sin(2*q2)*power(sin(q3),2)*sin(2*q4)*sin(q5) - 2*KUKA_LBR_param_.dblLink6InertYZ*sin(q2)*sin(2*q3)*sin(2*q4)*sin(q5) - 4*KUKA_LBR_param_.dblLink6InertXZ*power(cos(q2),2)*(cos(q4)*cos(q5)*sin(q3) + cos(q3)*power(cos(q4),2)*sin(q5) - cos(q3)*power(sin(q4),2)*sin(q5)) + 4*cos(q3)*sin(q2)*(-((KUKA_LBR_param_.dblLink6InertXX - KUKA_LBR_param_.dblLink6InertYY)*cos(q4)*cos(q5)*sin(q1)) + KUKA_LBR_param_.dblLink6InertXZ*power(cos(q4),2)*sin(q2)*sin(q5) - KUKA_LBR_param_.dblLink6InertXZ*sin(q2)*power(sin(q4),2)*sin(q5)) + 4*cos(q2)*(KUKA_LBR_param_.dblLink6InertYZ*cos(q3)*cos(q4)*cos(q5) - sin(q3)*((KUKA_LBR_param_.dblLink6InertXX - KUKA_LBR_param_.dblLink6InertYY)*cos(q5)*sin(q1)*sin(q3)*sin(q4) + KUKA_LBR_param_.dblLink6InertYZ*cos(2*q4)*sin(q5)) + power(cos(q3),2)*sin(q4)*((KUKA_LBR_param_.dblLink6InertXX - KUKA_LBR_param_.dblLink6InertYY)*cos(q5)*sin(q1) - KUKA_LBR_param_.dblLink6InertXZ*cos(q4)*sin(q2)*sin(q5)))) - 2*(16*KUKA_LBR_param_.dblLink6CogY*KUKA_LBR_param_.dblLink6CogZ*KUKA_LBR_param_.dblLink6Mass*cos(q6) + 16*KUKA_LBR_param_.dblLink6InertXY*cos(q3)*cos(q4)*cos(q5)*power(sin(q1),2)*sin(q2) - 16*KUKA_LBR_param_.dblLink6InertYZ*cos(q4)*cos(q5)*sin(q1)*power(sin(q2),2)*sin(q3) + 4*KUKA_LBR_param_.dblLink6InertXX*cos(q4)*cos(q5)*sin(2*q2)*sin(q3) + 4*KUKA_LBR_param_.dblLink6InertYY*cos(q4)*cos(q5)*sin(2*q2)*sin(q3) - 8*KUKA_LBR_param_.dblLink6InertZZ*cos(q4)*cos(q5)*sin(2*q2)*sin(q3) - 4*KUKA_LBR_param_.dblLink6InertXX*cos(q4)*cos(q5)*power(sin(q1),2)*sin(2*q2)*sin(q3) + 4*KUKA_LBR_param_.dblLink6InertYY*cos(q4)*cos(q5)*power(sin(q1),2)*sin(2*q2)*sin(q3) + 8*KUKA_LBR_param_.dblLink6InertXY*cos(q4)*cos(q5)*sin(2*q1)*sin(2*q2)*sin(q3) + 16*KUKA_LBR_param_.dblLink6InertXZ*power(cos(q3),2)*cos(q5)*sin(q1)*sin(q2)*sin(q4) + 4*KUKA_LBR_param_.dblLink6InertXX*cos(q3)*cos(q5)*sin(q3)*sin(q4) + 4*KUKA_LBR_param_.dblLink6InertYY*cos(q3)*cos(q5)*sin(q3)*sin(q4) + 4*KUKA_LBR_param_.dblLink6InertXX*cos(q3)*cos(q5)*power(sin(q2),2)*sin(q3)*sin(q4) + 4*KUKA_LBR_param_.dblLink6InertYY*cos(q3)*cos(q5)*power(sin(q2),2)*sin(q3)*sin(q4) + 4*KUKA_LBR_param_.dblLink6InertYY*cos(q3)*cos(q5)*power(sin(q1),2)*power(sin(q2),2)*sin(q3)*sin(q4) - 16*KUKA_LBR_param_.dblLink6InertXZ*cos(q5)*sin(q1)*sin(q2)*power(sin(q3),2)*sin(q4) - 4*KUKA_LBR_param_.dblLink6InertZZ*cos(q5)*sin(2*q3)*sin(q4) + 6*KUKA_LBR_param_.dblLink6InertXX*cos(q5)*power(sin(q1),2)*sin(2*q3)*sin(q4) - 6*KUKA_LBR_param_.dblLink6InertYY*cos(q5)*power(sin(q1),2)*sin(2*q3)*sin(q4) - 12*KUKA_LBR_param_.dblLink6InertXY*cos(q5)*sin(2*q1)*sin(2*q3)*sin(q4) - 4*KUKA_LBR_param_.dblLink6InertZZ*cos(q5)*power(sin(q2),2)*sin(2*q3)*sin(q4) - 2*KUKA_LBR_param_.dblLink6InertXX*cos(q5)*power(sin(q1),2)*power(sin(q2),2)*sin(2*q3)*sin(q4) + 4*KUKA_LBR_param_.dblLink6InertXY*cos(q5)*sin(2*q1)*power(sin(q2),2)*sin(2*q3)*sin(q4) + 8*KUKA_LBR_param_.dblLink6InertYZ*cos(q5)*sin(q1)*sin(2*q2)*sin(2*q3)*sin(q4) - 16*KUKA_LBR_param_.dblLink6InertYZ*cos(q3)*power(cos(q4),2)*sin(q1)*power(sin(q2),2)*sin(q5) + 4*KUKA_LBR_param_.dblLink6InertXX*cos(q3)*power(cos(q4),2)*sin(2*q2)*sin(q5) + 4*KUKA_LBR_param_.dblLink6InertYY*cos(q3)*power(cos(q4),2)*sin(2*q2)*sin(q5) - 8*KUKA_LBR_param_.dblLink6InertZZ*cos(q3)*power(cos(q4),2)*sin(2*q2)*sin(q5) - 4*KUKA_LBR_param_.dblLink6InertXX*cos(q3)*power(cos(q4),2)*power(sin(q1),2)*sin(2*q2)*sin(q5) + 4*KUKA_LBR_param_.dblLink6InertYY*cos(q3)*power(cos(q4),2)*power(sin(q1),2)*sin(2*q2)*sin(q5) + 8*KUKA_LBR_param_.dblLink6InertXY*cos(q3)*power(cos(q4),2)*sin(2*q1)*sin(2*q2)*sin(q5) - 16*KUKA_LBR_param_.dblLink6InertXY*power(cos(q4),2)*power(sin(q1),2)*sin(q2)*sin(q3)*sin(q5) - 2*KUKA_LBR_param_.dblLink6InertXX*cos(q4)*sin(q4)*sin(q5) - 2*KUKA_LBR_param_.dblLink6InertYY*cos(q4)*sin(q4)*sin(q5) + 4*KUKA_LBR_param_.dblLink6InertZZ*cos(q4)*sin(q4)*sin(q5) - 2*KUKA_LBR_param_.dblLink6InertXX*power(cos(q3),2)*cos(q4)*power(sin(q1),2)*power(sin(q2),2)*sin(q4)*sin(q5) - 2*KUKA_LBR_param_.dblLink6InertXX*cos(q4)*power(sin(q3),2)*sin(q4)*sin(q5) - 2*KUKA_LBR_param_.dblLink6InertYY*cos(q4)*power(sin(q3),2)*sin(q4)*sin(q5) + 4*KUKA_LBR_param_.dblLink6InertZZ*cos(q4)*power(sin(q3),2)*sin(q4)*sin(q5) - 2*KUKA_LBR_param_.dblLink6InertXX*cos(q4)*power(sin(q2),2)*power(sin(q3),2)*sin(q4)*sin(q5) - 2*KUKA_LBR_param_.dblLink6InertYY*cos(q4)*power(sin(q2),2)*power(sin(q3),2)*sin(q4)*sin(q5) + 4*KUKA_LBR_param_.dblLink6InertZZ*cos(q4)*power(sin(q2),2)*power(sin(q3),2)*sin(q4)*sin(q5) - 2*KUKA_LBR_param_.dblLink6InertYY*cos(q4)*power(sin(q1),2)*power(sin(q2),2)*power(sin(q3),2)*sin(q4)*sin(q5) + 16*KUKA_LBR_param_.dblLink6InertYZ*cos(q3)*sin(q1)*power(sin(q2),2)*power(sin(q4),2)*sin(q5) - 4*KUKA_LBR_param_.dblLink6InertXX*cos(q3)*sin(2*q2)*power(sin(q4),2)*sin(q5) - 4*KUKA_LBR_param_.dblLink6InertYY*cos(q3)*sin(2*q2)*power(sin(q4),2)*sin(q5) + 8*KUKA_LBR_param_.dblLink6InertZZ*cos(q3)*sin(2*q2)*power(sin(q4),2)*sin(q5) + 4*KUKA_LBR_param_.dblLink6InertXX*cos(q3)*power(sin(q1),2)*sin(2*q2)*power(sin(q4),2)*sin(q5) - 4*KUKA_LBR_param_.dblLink6InertYY*cos(q3)*power(sin(q1),2)*sin(2*q2)*power(sin(q4),2)*sin(q5) - 8*KUKA_LBR_param_.dblLink6InertXY*cos(q3)*sin(2*q1)*sin(2*q2)*power(sin(q4),2)*sin(q5) + 16*KUKA_LBR_param_.dblLink6InertXY*power(sin(q1),2)*sin(q2)*sin(q3)*power(sin(q4),2)*sin(q5) + KUKA_LBR_param_.dblLink6InertXX*power(cos(q3),2)*sin(2*q4)*sin(q5) + KUKA_LBR_param_.dblLink6InertYY*power(cos(q3),2)*sin(2*q4)*sin(q5) - 2*KUKA_LBR_param_.dblLink6InertZZ*power(cos(q3),2)*sin(2*q4)*sin(q5) - 3*KUKA_LBR_param_.dblLink6InertXX*power(sin(q1),2)*sin(2*q4)*sin(q5) + 3*KUKA_LBR_param_.dblLink6InertYY*power(sin(q1),2)*sin(2*q4)*sin(q5) + 3*KUKA_LBR_param_.dblLink6InertXX*power(cos(q3),2)*power(sin(q1),2)*sin(2*q4)*sin(q5) - 3*KUKA_LBR_param_.dblLink6InertYY*power(cos(q3),2)*power(sin(q1),2)*sin(2*q4)*sin(q5) + 6*KUKA_LBR_param_.dblLink6InertXY*sin(2*q1)*sin(2*q4)*sin(q5) - 6*KUKA_LBR_param_.dblLink6InertXY*power(cos(q3),2)*sin(2*q1)*sin(2*q4)*sin(q5) + 3*KUKA_LBR_param_.dblLink6InertXX*power(sin(q2),2)*sin(2*q4)*sin(q5) + 3*KUKA_LBR_param_.dblLink6InertYY*power(sin(q2),2)*sin(2*q4)*sin(q5) - 6*KUKA_LBR_param_.dblLink6InertZZ*power(sin(q2),2)*sin(2*q4)*sin(q5) + KUKA_LBR_param_.dblLink6InertXX*power(cos(q3),2)*power(sin(q2),2)*sin(2*q4)*sin(q5) + KUKA_LBR_param_.dblLink6InertYY*power(cos(q3),2)*power(sin(q2),2)*sin(2*q4)*sin(q5) - 2*KUKA_LBR_param_.dblLink6InertZZ*power(cos(q3),2)*power(sin(q2),2)*sin(2*q4)*sin(q5) - 3*KUKA_LBR_param_.dblLink6InertXX*power(sin(q1),2)*power(sin(q2),2)*sin(2*q4)*sin(q5) + 3*KUKA_LBR_param_.dblLink6InertYY*power(sin(q1),2)*power(sin(q2),2)*sin(2*q4)*sin(q5) + KUKA_LBR_param_.dblLink6InertYY*power(cos(q3),2)*power(sin(q1),2)*power(sin(q2),2)*sin(2*q4)*sin(q5) + 6*KUKA_LBR_param_.dblLink6InertXY*sin(2*q1)*power(sin(q2),2)*sin(2*q4)*sin(q5) + 2*KUKA_LBR_param_.dblLink6InertXY*power(cos(q3),2)*sin(2*q1)*power(sin(q2),2)*sin(2*q4)*sin(q5) + 12*KUKA_LBR_param_.dblLink6InertYZ*sin(q1)*sin(2*q2)*sin(2*q4)*sin(q5) + 4*KUKA_LBR_param_.dblLink6InertYZ*power(cos(q3),2)*sin(q1)*sin(2*q2)*sin(2*q4)*sin(q5) - 3*KUKA_LBR_param_.dblLink6InertXX*power(sin(q1),2)*power(sin(q3),2)*sin(2*q4)*sin(q5) + 3*KUKA_LBR_param_.dblLink6InertYY*power(sin(q1),2)*power(sin(q3),2)*sin(2*q4)*sin(q5) + 6*KUKA_LBR_param_.dblLink6InertXY*sin(2*q1)*power(sin(q3),2)*sin(2*q4)*sin(q5) + KUKA_LBR_param_.dblLink6InertXX*power(sin(q1),2)*power(sin(q2),2)*power(sin(q3),2)*sin(2*q4)*sin(q5) - 2*KUKA_LBR_param_.dblLink6InertXY*sin(2*q1)*power(sin(q2),2)*power(sin(q3),2)*sin(2*q4)*sin(q5) - 4*KUKA_LBR_param_.dblLink6InertYZ*sin(q1)*sin(2*q2)*power(sin(q3),2)*sin(2*q4)*sin(q5) - 8*KUKA_LBR_param_.dblLink6InertXZ*sin(q1)*sin(q2)*sin(2*q3)*sin(2*q4)*sin(q5) + 4*cos(q2)*(4*KUKA_LBR_param_.dblLink6InertXZ*cos(q3)*cos(q4)*cos(q5)*sin(q1) - 4*KUKA_LBR_param_.dblLink6InertXY*power(cos(q3),2)*cos(q5)*power(sin(q1),2)*sin(q4) + 4*KUKA_LBR_param_.dblLink6InertXY*cos(q5)*power(sin(q1),2)*power(sin(q3),2)*sin(q4) + (-4*KUKA_LBR_param_.dblLink6InertXZ*power(cos(q4),2)*sin(q1)*sin(q3) + 4*KUKA_LBR_param_.dblLink6InertXZ*sin(q1)*sin(q3)*power(sin(q4),2) + 2*KUKA_LBR_param_.dblLink6InertXY*power(sin(q1),2)*sin(2*q3)*sin(2*q4) + (KUKA_LBR_param_.dblLink6InertXX - KUKA_LBR_param_.dblLink6InertYY)*sin(2*q1)*sin(2*q3)*sin(2*q4))*sin(q5)) + power(cos(q2),2)*(-2*KUKA_LBR_param_.dblLink6InertXX*cos(q5)*sin(2*q3)*sin(q4) - 2*KUKA_LBR_param_.dblLink6InertYY*cos(q5)*sin(2*q3)*sin(q4) + 4*KUKA_LBR_param_.dblLink6InertZZ*cos(q5)*sin(2*q3)*sin(q4) - 2*KUKA_LBR_param_.dblLink6InertYY*cos(q5)*power(sin(q1),2)*sin(2*q3)*sin(q4) - 4*KUKA_LBR_param_.dblLink6InertXY*cos(q5)*sin(2*q1)*sin(2*q3)*sin(q4) + 16*KUKA_LBR_param_.dblLink6InertYZ*cos(q3)*power(cos(q4),2)*sin(q1)*sin(q5) - 3*KUKA_LBR_param_.dblLink6InertXX*sin(2*q4)*sin(q5) - 3*KUKA_LBR_param_.dblLink6InertYY*sin(2*q4)*sin(q5) + 6*KUKA_LBR_param_.dblLink6InertZZ*sin(2*q4)*sin(q5) + 3*KUKA_LBR_param_.dblLink6InertXX*power(sin(q1),2)*sin(2*q4)*sin(q5) - 3*KUKA_LBR_param_.dblLink6InertYY*power(sin(q1),2)*sin(2*q4)*sin(q5) + power(cos(q3),2)*sin(q1)*(-4*KUKA_LBR_param_.dblLink6InertXY*cos(q1) + KUKA_LBR_param_.dblLink6InertXX*sin(q1))*sin(2*q4)*sin(q5) - 6*KUKA_LBR_param_.dblLink6InertXY*sin(2*q1)*sin(2*q4)*sin(q5) + KUKA_LBR_param_.dblLink6InertXX*power(sin(q3),2)*sin(2*q4)*sin(q5) + KUKA_LBR_param_.dblLink6InertYY*power(sin(q3),2)*sin(2*q4)*sin(q5) - 2*KUKA_LBR_param_.dblLink6InertZZ*power(sin(q3),2)*sin(2*q4)*sin(q5) + KUKA_LBR_param_.dblLink6InertYY*power(sin(q1),2)*power(sin(q3),2)*sin(2*q4)*sin(q5) + 2*KUKA_LBR_param_.dblLink6InertXY*sin(2*q1)*power(sin(q3),2)*sin(2*q4)*sin(q5) + 4*cos(q3)*sin(q1)*sin(q4)*(KUKA_LBR_param_.dblLink6InertXX*cos(q5)*sin(q1)*sin(q3) - 4*KUKA_LBR_param_.dblLink6InertYZ*sin(q4)*sin(q5)) + 2*cos(q4)*(8*KUKA_LBR_param_.dblLink6InertYZ*cos(q5)*sin(q1)*sin(q3) - (power(cos(q3),2)*(KUKA_LBR_param_.dblLink6InertXX + KUKA_LBR_param_.dblLink6InertYY - 2*KUKA_LBR_param_.dblLink6InertZZ + KUKA_LBR_param_.dblLink6InertYY*power(sin(q1),2)) + KUKA_LBR_param_.dblLink6InertXX*power(sin(q1),2)*power(sin(q3),2))*sin(q4)*sin(q5))) + 16*KUKA_LBR_param_.dblLink6CogX*KUKA_LBR_param_.dblLink6CogZ*KUKA_LBR_param_.dblLink6Mass*sin(q6)))/32.0 - KUKA_LBR_param_.dblLink7Mass*(cos(q5)*(KUKA_LBR_param_.dblLink7CogZ*sin(q2)*sin(q3)*sin(q6) + cos(q2)*sin(q4)*(KUKA_LBR_param_.dblLink7CogY*cos(q7) + KUKA_LBR_param_.dblLink7CogX*sin(q7)) - cos(q6)*sin(q2)*sin(q3)*(KUKA_LBR_param_.dblLink7CogX*cos(q7) - KUKA_LBR_param_.dblLink7CogY*sin(q7))) + sin(q5)*(cos(q7)*(KUKA_LBR_param_.dblLink7CogY*sin(q2)*sin(q3) + KUKA_LBR_param_.dblLink7CogX*cos(q2)*cos(q6)*sin(q4)) + KUKA_LBR_param_.dblLink7CogX*sin(q2)*sin(q3)*sin(q7) - cos(q2)*sin(q4)*(KUKA_LBR_param_.dblLink7CogZ*sin(q6) + KUKA_LBR_param_.dblLink7CogY*cos(q6)*sin(q7))) - cos(q3)*cos(q4)*sin(q2)*(cos(q5)*(KUKA_LBR_param_.dblLink7CogY*cos(q7) + KUKA_LBR_param_.dblLink7CogX*sin(q7)) - sin(q5)*(KUKA_LBR_param_.dblLink7CogZ*sin(q6) + cos(q6)*(-(KUKA_LBR_param_.dblLink7CogX*cos(q7)) + KUKA_LBR_param_.dblLink7CogY*sin(q7)))))*(cos(q2)*(cos(q4)*(-(KUKA_LBR_param_.dblLink7CogX*cos(q6)*cos(q7)) + KUKA_LBR_param_.dblLink7CogZ*sin(q6) + KUKA_LBR_param_.dblLink7CogY*cos(q6)*sin(q7)) - cos(q5)*sin(q4)*(KUKA_LBR_param_.dblLink7CogZ*cos(q6) + KUKA_LBR_param_.dblLink7CogX*cos(q7)*sin(q6) - KUKA_LBR_param_.dblLink7CogY*sin(q6)*sin(q7))) + sin(q2)*(-(sin(q3)*sin(q5)*(KUKA_LBR_param_.dblLink7CogZ*cos(q6) + sin(q6)*(KUKA_LBR_param_.dblLink7CogX*cos(q7) - KUKA_LBR_param_.dblLink7CogY*sin(q7)))) + cos(q3)*(sin(q4)*(-(KUKA_LBR_param_.dblLink7CogX*cos(q6)*cos(q7)) + KUKA_LBR_param_.dblLink7CogZ*sin(q6) + KUKA_LBR_param_.dblLink7CogY*cos(q6)*sin(q7)) + cos(q4)*cos(q5)*(KUKA_LBR_param_.dblLink7CogZ*cos(q6) + KUKA_LBR_param_.dblLink7CogX*cos(q7)*sin(q6) - KUKA_LBR_param_.dblLink7CogY*sin(q6)*sin(q7))))) + KUKA_LBR_param_.dblLink7Mass*(KUKA_LBR_param_.dblLink7CogZ*cos(q5)*cos(q6)*sin(q1)*sin(q2)*sin(q4) - KUKA_LBR_param_.dblLink7CogX*cos(q1)*cos(q6)*cos(q7)*sin(q3)*sin(q4) + KUKA_LBR_param_.dblLink7CogZ*cos(q1)*cos(q3)*cos(q6)*sin(q5) + KUKA_LBR_param_.dblLink7CogX*cos(q5)*cos(q7)*sin(q1)*sin(q2)*sin(q4)*sin(q6) + KUKA_LBR_param_.dblLink7CogZ*cos(q1)*sin(q3)*sin(q4)*sin(q6) + KUKA_LBR_param_.dblLink7CogX*cos(q1)*cos(q3)*cos(q7)*sin(q5)*sin(q6) + KUKA_LBR_param_.dblLink7CogY*cos(q1)*cos(q6)*sin(q3)*sin(q4)*sin(q7) - KUKA_LBR_param_.dblLink7CogY*cos(q5)*sin(q1)*sin(q2)*sin(q4)*sin(q6)*sin(q7) - KUKA_LBR_param_.dblLink7CogY*cos(q1)*cos(q3)*sin(q5)*sin(q6)*sin(q7) + cos(q4)*(cos(q6)*(KUKA_LBR_param_.dblLink7CogX*cos(q7)*sin(q1)*sin(q2) + KUKA_LBR_param_.dblLink7CogZ*cos(q1)*cos(q5)*sin(q3) - KUKA_LBR_param_.dblLink7CogY*sin(q1)*sin(q2)*sin(q7)) - sin(q6)*(KUKA_LBR_param_.dblLink7CogZ*sin(q1)*sin(q2) + cos(q1)*cos(q5)*sin(q3)*(-(KUKA_LBR_param_.dblLink7CogX*cos(q7)) + KUKA_LBR_param_.dblLink7CogY*sin(q7)))) + cos(q2)*sin(q1)*(-(sin(q3)*sin(q5)*(KUKA_LBR_param_.dblLink7CogZ*cos(q6) + sin(q6)*(KUKA_LBR_param_.dblLink7CogX*cos(q7) - KUKA_LBR_param_.dblLink7CogY*sin(q7)))) + cos(q3)*(sin(q4)*(-(KUKA_LBR_param_.dblLink7CogX*cos(q6)*cos(q7)) + KUKA_LBR_param_.dblLink7CogZ*sin(q6) + KUKA_LBR_param_.dblLink7CogY*cos(q6)*sin(q7)) + cos(q4)*cos(q5)*(KUKA_LBR_param_.dblLink7CogZ*cos(q6) + KUKA_LBR_param_.dblLink7CogX*cos(q7)*sin(q6) - KUKA_LBR_param_.dblLink7CogY*sin(q6)*sin(q7)))))*(cos(q1)*(cos(q4)*sin(q3)*(cos(q5)*(KUKA_LBR_param_.dblLink7CogY*cos(q7) + KUKA_LBR_param_.dblLink7CogX*sin(q7)) + sin(q5)*(KUKA_LBR_param_.dblLink7CogX*cos(q6)*cos(q7) - KUKA_LBR_param_.dblLink7CogZ*sin(q6) - KUKA_LBR_param_.dblLink7CogY*cos(q6)*sin(q7))) + cos(q3)*(sin(q5)*(KUKA_LBR_param_.dblLink7CogY*cos(q7) + KUKA_LBR_param_.dblLink7CogX*sin(q7)) + cos(q5)*(-(KUKA_LBR_param_.dblLink7CogX*cos(q6)*cos(q7)) + KUKA_LBR_param_.dblLink7CogZ*sin(q6) + KUKA_LBR_param_.dblLink7CogY*cos(q6)*sin(q7)))) + sin(q1)*(sin(q2)*sin(q4)*(cos(q5)*(KUKA_LBR_param_.dblLink7CogY*cos(q7) + KUKA_LBR_param_.dblLink7CogX*sin(q7)) + sin(q5)*(KUKA_LBR_param_.dblLink7CogX*cos(q6)*cos(q7) - KUKA_LBR_param_.dblLink7CogZ*sin(q6) - KUKA_LBR_param_.dblLink7CogY*cos(q6)*sin(q7))) + cos(q2)*(cos(q3)*cos(q4)*(cos(q5)*(KUKA_LBR_param_.dblLink7CogY*cos(q7) + KUKA_LBR_param_.dblLink7CogX*sin(q7)) + sin(q5)*(KUKA_LBR_param_.dblLink7CogX*cos(q6)*cos(q7) - KUKA_LBR_param_.dblLink7CogZ*sin(q6) - KUKA_LBR_param_.dblLink7CogY*cos(q6)*sin(q7))) - sin(q3)*(sin(q5)*(KUKA_LBR_param_.dblLink7CogY*cos(q7) + KUKA_LBR_param_.dblLink7CogX*sin(q7)) + cos(q5)*(-(KUKA_LBR_param_.dblLink7CogX*cos(q6)*cos(q7)) + KUKA_LBR_param_.dblLink7CogZ*sin(q6) + KUKA_LBR_param_.dblLink7CogY*cos(q6)*sin(q7)))))) - KUKA_LBR_param_.dblLink7Mass*(sin(q1)*(-(cos(q4)*sin(q3)*(cos(q5)*(KUKA_LBR_param_.dblLink7CogY*cos(q7) + KUKA_LBR_param_.dblLink7CogX*sin(q7)) + sin(q5)*(KUKA_LBR_param_.dblLink7CogX*cos(q6)*cos(q7) - KUKA_LBR_param_.dblLink7CogZ*sin(q6) - KUKA_LBR_param_.dblLink7CogY*cos(q6)*sin(q7)))) - cos(q3)*(sin(q5)*(KUKA_LBR_param_.dblLink7CogY*cos(q7) + KUKA_LBR_param_.dblLink7CogX*sin(q7)) + cos(q5)*(-(KUKA_LBR_param_.dblLink7CogX*cos(q6)*cos(q7)) + KUKA_LBR_param_.dblLink7CogZ*sin(q6) + KUKA_LBR_param_.dblLink7CogY*cos(q6)*sin(q7)))) + cos(q1)*(sin(q2)*sin(q4)*(cos(q5)*(KUKA_LBR_param_.dblLink7CogY*cos(q7) + KUKA_LBR_param_.dblLink7CogX*sin(q7)) + sin(q5)*(KUKA_LBR_param_.dblLink7CogX*cos(q6)*cos(q7) - KUKA_LBR_param_.dblLink7CogZ*sin(q6) - KUKA_LBR_param_.dblLink7CogY*cos(q6)*sin(q7))) + cos(q2)*(cos(q3)*cos(q4)*(cos(q5)*(KUKA_LBR_param_.dblLink7CogY*cos(q7) + KUKA_LBR_param_.dblLink7CogX*sin(q7)) + sin(q5)*(KUKA_LBR_param_.dblLink7CogX*cos(q6)*cos(q7) - KUKA_LBR_param_.dblLink7CogZ*sin(q6) - KUKA_LBR_param_.dblLink7CogY*cos(q6)*sin(q7))) - sin(q3)*(sin(q5)*(KUKA_LBR_param_.dblLink7CogY*cos(q7) + KUKA_LBR_param_.dblLink7CogX*sin(q7)) + cos(q5)*(-(KUKA_LBR_param_.dblLink7CogX*cos(q6)*cos(q7)) + KUKA_LBR_param_.dblLink7CogZ*sin(q6) + KUKA_LBR_param_.dblLink7CogY*cos(q6)*sin(q7))))))*(sin(q1)*(cos(q6)*(-(KUKA_LBR_param_.dblLink7CogX*cos(q7)*sin(q3)*sin(q4)) + KUKA_LBR_param_.dblLink7CogZ*cos(q3)*sin(q5) + KUKA_LBR_param_.dblLink7CogY*sin(q3)*sin(q4)*sin(q7)) + sin(q6)*(KUKA_LBR_param_.dblLink7CogZ*sin(q3)*sin(q4) + cos(q3)*sin(q5)*(KUKA_LBR_param_.dblLink7CogX*cos(q7) - KUKA_LBR_param_.dblLink7CogY*sin(q7))) + cos(q4)*cos(q5)*sin(q3)*(KUKA_LBR_param_.dblLink7CogZ*cos(q6) + sin(q6)*(KUKA_LBR_param_.dblLink7CogX*cos(q7) - KUKA_LBR_param_.dblLink7CogY*sin(q7)))) - cos(q1)*(sin(q2)*(cos(q4)*(KUKA_LBR_param_.dblLink7CogX*cos(q6)*cos(q7) - KUKA_LBR_param_.dblLink7CogZ*sin(q6) - KUKA_LBR_param_.dblLink7CogY*cos(q6)*sin(q7)) + cos(q5)*sin(q4)*(KUKA_LBR_param_.dblLink7CogZ*cos(q6) + KUKA_LBR_param_.dblLink7CogX*cos(q7)*sin(q6) - KUKA_LBR_param_.dblLink7CogY*sin(q6)*sin(q7))) + cos(q2)*(-(sin(q3)*sin(q5)*(KUKA_LBR_param_.dblLink7CogZ*cos(q6) + sin(q6)*(KUKA_LBR_param_.dblLink7CogX*cos(q7) - KUKA_LBR_param_.dblLink7CogY*sin(q7)))) + cos(q3)*(sin(q4)*(-(KUKA_LBR_param_.dblLink7CogX*cos(q6)*cos(q7)) + KUKA_LBR_param_.dblLink7CogZ*sin(q6) + KUKA_LBR_param_.dblLink7CogY*cos(q6)*sin(q7)) + cos(q4)*cos(q5)*(KUKA_LBR_param_.dblLink7CogZ*cos(q6) + KUKA_LBR_param_.dblLink7CogX*cos(q7)*sin(q6) - KUKA_LBR_param_.dblLink7CogY*sin(q6)*sin(q7))))));
dblMassInertFullRow5Col7 = (KUKA_LBR_param_.dblLink7InertXY*cos(q4)*sin(q1)*sin(q2) + KUKA_LBR_param_.dblLink7InertXZ*cos(q3)*sin(q2)*sin(q4) + KUKA_LBR_param_.dblLink7InertXX*sin(q1)*sin(q3)*sin(q4) + cos(q2)*(KUKA_LBR_param_.dblLink7InertXZ*cos(q4) - cos(q3)*(KUKA_LBR_param_.dblLink7InertXX*cos(q1) + KUKA_LBR_param_.dblLink7InertXY*sin(q1))*sin(q4)) + cos(q1)*(KUKA_LBR_param_.dblLink7InertXX*cos(q4)*sin(q2) - KUKA_LBR_param_.dblLink7InertXY*sin(q3)*sin(q4)))*(cos(q6)*(sin(q1)*sin(q3)*sin(q4) + cos(q1)*(cos(q4)*sin(q2) - cos(q2)*cos(q3)*sin(q4))) - (cos(q5)*(cos(q4)*sin(q1)*sin(q3) - cos(q1)*(cos(q2)*cos(q3)*cos(q4) + sin(q2)*sin(q4))) + (cos(q3)*sin(q1) + cos(q1)*cos(q2)*sin(q3))*sin(q5))*sin(q6)) + (KUKA_LBR_param_.dblLink7InertYY*cos(q4)*sin(q1)*sin(q2) + KUKA_LBR_param_.dblLink7InertYZ*cos(q3)*sin(q2)*sin(q4) + KUKA_LBR_param_.dblLink7InertXY*sin(q1)*sin(q3)*sin(q4) + cos(q2)*(KUKA_LBR_param_.dblLink7InertYZ*cos(q4) - cos(q3)*(KUKA_LBR_param_.dblLink7InertXY*cos(q1) + KUKA_LBR_param_.dblLink7InertYY*sin(q1))*sin(q4)) + cos(q1)*(KUKA_LBR_param_.dblLink7InertXY*cos(q4)*sin(q2) - KUKA_LBR_param_.dblLink7InertYY*sin(q3)*sin(q4)))*(cos(q6)*(cos(q4)*sin(q1)*sin(q2) - (cos(q2)*cos(q3)*sin(q1) + cos(q1)*sin(q3))*sin(q4)) + (cos(q5)*sin(q1)*sin(q2)*sin(q4) + cos(q1)*(cos(q4)*cos(q5)*sin(q3) + cos(q3)*sin(q5)) + cos(q2)*sin(q1)*(cos(q3)*cos(q4)*cos(q5) - sin(q3)*sin(q5)))*sin(q6)) + (KUKA_LBR_param_.dblLink7InertYZ*cos(q4)*sin(q1)*sin(q2) + KUKA_LBR_param_.dblLink7InertZZ*cos(q3)*sin(q2)*sin(q4) + KUKA_LBR_param_.dblLink7InertXZ*sin(q1)*sin(q3)*sin(q4) + cos(q2)*(KUKA_LBR_param_.dblLink7InertZZ*cos(q4) - cos(q3)*(KUKA_LBR_param_.dblLink7InertXZ*cos(q1) + KUKA_LBR_param_.dblLink7InertYZ*sin(q1))*sin(q4)) + cos(q1)*(KUKA_LBR_param_.dblLink7InertXZ*cos(q4)*sin(q2) - KUKA_LBR_param_.dblLink7InertYZ*sin(q3)*sin(q4)))*(cos(q2)*(cos(q4)*cos(q6) + cos(q5)*sin(q4)*sin(q6)) + sin(q2)*(sin(q3)*sin(q5)*sin(q6) + cos(q3)*(cos(q6)*sin(q4) - cos(q4)*cos(q5)*sin(q6)))) - KUKA_LBR_param_.dblLink7Mass*(-(KUKA_LBR_param_.dblLink7CogY*cos(q6)*cos(q7)*sin(q2)*sin(q3)*sin(q5)) - KUKA_LBR_param_.dblLink7CogX*cos(q2)*cos(q7)*sin(q4)*sin(q5) + KUKA_LBR_param_.dblLink7CogY*cos(q2)*cos(q4)*cos(q7)*sin(q6) - KUKA_LBR_param_.dblLink7CogX*cos(q6)*sin(q2)*sin(q3)*sin(q5)*sin(q7) + KUKA_LBR_param_.dblLink7CogY*cos(q2)*sin(q4)*sin(q5)*sin(q7) + KUKA_LBR_param_.dblLink7CogX*cos(q2)*cos(q4)*sin(q6)*sin(q7) + cos(q5)*(cos(q7)*(KUKA_LBR_param_.dblLink7CogX*sin(q2)*sin(q3) - KUKA_LBR_param_.dblLink7CogY*cos(q2)*cos(q6)*sin(q4)) - (KUKA_LBR_param_.dblLink7CogY*sin(q2)*sin(q3) + KUKA_LBR_param_.dblLink7CogX*cos(q2)*cos(q6)*sin(q4))*sin(q7)) + cos(q3)*sin(q2)*(sin(q4)*sin(q6)*(KUKA_LBR_param_.dblLink7CogY*cos(q7) + KUKA_LBR_param_.dblLink7CogX*sin(q7)) + cos(q4)*(cos(q5)*cos(q6)*(KUKA_LBR_param_.dblLink7CogY*cos(q7) + KUKA_LBR_param_.dblLink7CogX*sin(q7)) + sin(q5)*(KUKA_LBR_param_.dblLink7CogX*cos(q7) - KUKA_LBR_param_.dblLink7CogY*sin(q7)))))*(cos(q5)*(KUKA_LBR_param_.dblLink7CogZ*sin(q2)*sin(q3)*sin(q6) + cos(q2)*sin(q4)*(KUKA_LBR_param_.dblLink7CogY*cos(q7) + KUKA_LBR_param_.dblLink7CogX*sin(q7)) - cos(q6)*sin(q2)*sin(q3)*(KUKA_LBR_param_.dblLink7CogX*cos(q7) - KUKA_LBR_param_.dblLink7CogY*sin(q7))) + sin(q5)*(cos(q7)*(KUKA_LBR_param_.dblLink7CogY*sin(q2)*sin(q3) + KUKA_LBR_param_.dblLink7CogX*cos(q2)*cos(q6)*sin(q4)) + KUKA_LBR_param_.dblLink7CogX*sin(q2)*sin(q3)*sin(q7) - cos(q2)*sin(q4)*(KUKA_LBR_param_.dblLink7CogZ*sin(q6) + KUKA_LBR_param_.dblLink7CogY*cos(q6)*sin(q7))) - cos(q3)*cos(q4)*sin(q2)*(cos(q5)*(KUKA_LBR_param_.dblLink7CogY*cos(q7) + KUKA_LBR_param_.dblLink7CogX*sin(q7)) - sin(q5)*(KUKA_LBR_param_.dblLink7CogZ*sin(q6) + cos(q6)*(-(KUKA_LBR_param_.dblLink7CogX*cos(q7)) + KUKA_LBR_param_.dblLink7CogY*sin(q7))))) + KUKA_LBR_param_.dblLink7Mass*(sin(q1)*(-(cos(q4)*sin(q3)*(cos(q5)*(KUKA_LBR_param_.dblLink7CogY*cos(q7) + KUKA_LBR_param_.dblLink7CogX*sin(q7)) + sin(q5)*(KUKA_LBR_param_.dblLink7CogX*cos(q6)*cos(q7) - KUKA_LBR_param_.dblLink7CogZ*sin(q6) - KUKA_LBR_param_.dblLink7CogY*cos(q6)*sin(q7)))) - cos(q3)*(sin(q5)*(KUKA_LBR_param_.dblLink7CogY*cos(q7) + KUKA_LBR_param_.dblLink7CogX*sin(q7)) + cos(q5)*(-(KUKA_LBR_param_.dblLink7CogX*cos(q6)*cos(q7)) + KUKA_LBR_param_.dblLink7CogZ*sin(q6) + KUKA_LBR_param_.dblLink7CogY*cos(q6)*sin(q7)))) + cos(q1)*(sin(q2)*sin(q4)*(cos(q5)*(KUKA_LBR_param_.dblLink7CogY*cos(q7) + KUKA_LBR_param_.dblLink7CogX*sin(q7)) + sin(q5)*(KUKA_LBR_param_.dblLink7CogX*cos(q6)*cos(q7) - KUKA_LBR_param_.dblLink7CogZ*sin(q6) - KUKA_LBR_param_.dblLink7CogY*cos(q6)*sin(q7))) + cos(q2)*(cos(q3)*cos(q4)*(cos(q5)*(KUKA_LBR_param_.dblLink7CogY*cos(q7) + KUKA_LBR_param_.dblLink7CogX*sin(q7)) + sin(q5)*(KUKA_LBR_param_.dblLink7CogX*cos(q6)*cos(q7) - KUKA_LBR_param_.dblLink7CogZ*sin(q6) - KUKA_LBR_param_.dblLink7CogY*cos(q6)*sin(q7))) - sin(q3)*(sin(q5)*(KUKA_LBR_param_.dblLink7CogY*cos(q7) + KUKA_LBR_param_.dblLink7CogX*sin(q7)) + cos(q5)*(-(KUKA_LBR_param_.dblLink7CogX*cos(q6)*cos(q7)) + KUKA_LBR_param_.dblLink7CogZ*sin(q6) + KUKA_LBR_param_.dblLink7CogY*cos(q6)*sin(q7))))))*(sin(q1)*(cos(q3)*(-(cos(q6)*sin(q5)*(KUKA_LBR_param_.dblLink7CogY*cos(q7) + KUKA_LBR_param_.dblLink7CogX*sin(q7))) + cos(q5)*(KUKA_LBR_param_.dblLink7CogX*cos(q7) - KUKA_LBR_param_.dblLink7CogY*sin(q7))) - sin(q3)*(sin(q4)*sin(q6)*(KUKA_LBR_param_.dblLink7CogY*cos(q7) + KUKA_LBR_param_.dblLink7CogX*sin(q7)) + cos(q4)*(cos(q5)*cos(q6)*(KUKA_LBR_param_.dblLink7CogY*cos(q7) + KUKA_LBR_param_.dblLink7CogX*sin(q7)) + sin(q5)*(KUKA_LBR_param_.dblLink7CogX*cos(q7) - KUKA_LBR_param_.dblLink7CogY*sin(q7))))) + cos(q1)*(sin(q2)*(cos(q7)*(KUKA_LBR_param_.dblLink7CogX*sin(q4)*sin(q5) - KUKA_LBR_param_.dblLink7CogY*cos(q4)*sin(q6)) - (KUKA_LBR_param_.dblLink7CogY*sin(q4)*sin(q5) + KUKA_LBR_param_.dblLink7CogX*cos(q4)*sin(q6))*sin(q7) + cos(q5)*cos(q6)*sin(q4)*(KUKA_LBR_param_.dblLink7CogY*cos(q7) + KUKA_LBR_param_.dblLink7CogX*sin(q7))) + cos(q2)*(sin(q3)*(-(cos(q6)*sin(q5)*(KUKA_LBR_param_.dblLink7CogY*cos(q7) + KUKA_LBR_param_.dblLink7CogX*sin(q7))) + cos(q5)*(KUKA_LBR_param_.dblLink7CogX*cos(q7) - KUKA_LBR_param_.dblLink7CogY*sin(q7))) + cos(q3)*(sin(q4)*sin(q6)*(KUKA_LBR_param_.dblLink7CogY*cos(q7) + KUKA_LBR_param_.dblLink7CogX*sin(q7)) + cos(q4)*(cos(q5)*cos(q6)*(KUKA_LBR_param_.dblLink7CogY*cos(q7) + KUKA_LBR_param_.dblLink7CogX*sin(q7)) + sin(q5)*(KUKA_LBR_param_.dblLink7CogX*cos(q7) - KUKA_LBR_param_.dblLink7CogY*sin(q7))))))) + KUKA_LBR_param_.dblLink7Mass*(cos(q1)*(cos(q4)*sin(q3)*(cos(q5)*(KUKA_LBR_param_.dblLink7CogY*cos(q7) + KUKA_LBR_param_.dblLink7CogX*sin(q7)) + sin(q5)*(KUKA_LBR_param_.dblLink7CogX*cos(q6)*cos(q7) - KUKA_LBR_param_.dblLink7CogZ*sin(q6) - KUKA_LBR_param_.dblLink7CogY*cos(q6)*sin(q7))) + cos(q3)*(sin(q5)*(KUKA_LBR_param_.dblLink7CogY*cos(q7) + KUKA_LBR_param_.dblLink7CogX*sin(q7)) + cos(q5)*(-(KUKA_LBR_param_.dblLink7CogX*cos(q6)*cos(q7)) + KUKA_LBR_param_.dblLink7CogZ*sin(q6) + KUKA_LBR_param_.dblLink7CogY*cos(q6)*sin(q7)))) + sin(q1)*(sin(q2)*sin(q4)*(cos(q5)*(KUKA_LBR_param_.dblLink7CogY*cos(q7) + KUKA_LBR_param_.dblLink7CogX*sin(q7)) + sin(q5)*(KUKA_LBR_param_.dblLink7CogX*cos(q6)*cos(q7) - KUKA_LBR_param_.dblLink7CogZ*sin(q6) - KUKA_LBR_param_.dblLink7CogY*cos(q6)*sin(q7))) + cos(q2)*(cos(q3)*cos(q4)*(cos(q5)*(KUKA_LBR_param_.dblLink7CogY*cos(q7) + KUKA_LBR_param_.dblLink7CogX*sin(q7)) + sin(q5)*(KUKA_LBR_param_.dblLink7CogX*cos(q6)*cos(q7) - KUKA_LBR_param_.dblLink7CogZ*sin(q6) - KUKA_LBR_param_.dblLink7CogY*cos(q6)*sin(q7))) - sin(q3)*(sin(q5)*(KUKA_LBR_param_.dblLink7CogY*cos(q7) + KUKA_LBR_param_.dblLink7CogX*sin(q7)) + cos(q5)*(-(KUKA_LBR_param_.dblLink7CogX*cos(q6)*cos(q7)) + KUKA_LBR_param_.dblLink7CogZ*sin(q6) + KUKA_LBR_param_.dblLink7CogY*cos(q6)*sin(q7))))))*(cos(q1)*(cos(q3)*(cos(q6)*sin(q5)*(KUKA_LBR_param_.dblLink7CogY*cos(q7) + KUKA_LBR_param_.dblLink7CogX*sin(q7)) + cos(q5)*(-(KUKA_LBR_param_.dblLink7CogX*cos(q7)) + KUKA_LBR_param_.dblLink7CogY*sin(q7))) + sin(q3)*(sin(q4)*sin(q6)*(KUKA_LBR_param_.dblLink7CogY*cos(q7) + KUKA_LBR_param_.dblLink7CogX*sin(q7)) + cos(q4)*(cos(q5)*cos(q6)*(KUKA_LBR_param_.dblLink7CogY*cos(q7) + KUKA_LBR_param_.dblLink7CogX*sin(q7)) + sin(q5)*(KUKA_LBR_param_.dblLink7CogX*cos(q7) - KUKA_LBR_param_.dblLink7CogY*sin(q7))))) + sin(q1)*(sin(q2)*(cos(q7)*(KUKA_LBR_param_.dblLink7CogX*sin(q4)*sin(q5) - KUKA_LBR_param_.dblLink7CogY*cos(q4)*sin(q6)) - (KUKA_LBR_param_.dblLink7CogY*sin(q4)*sin(q5) + KUKA_LBR_param_.dblLink7CogX*cos(q4)*sin(q6))*sin(q7) + cos(q5)*cos(q6)*sin(q4)*(KUKA_LBR_param_.dblLink7CogY*cos(q7) + KUKA_LBR_param_.dblLink7CogX*sin(q7))) + cos(q2)*(sin(q3)*(-(cos(q6)*sin(q5)*(KUKA_LBR_param_.dblLink7CogY*cos(q7) + KUKA_LBR_param_.dblLink7CogX*sin(q7))) + cos(q5)*(KUKA_LBR_param_.dblLink7CogX*cos(q7) - KUKA_LBR_param_.dblLink7CogY*sin(q7))) + cos(q3)*(sin(q4)*sin(q6)*(KUKA_LBR_param_.dblLink7CogY*cos(q7) + KUKA_LBR_param_.dblLink7CogX*sin(q7)) + cos(q4)*(cos(q5)*cos(q6)*(KUKA_LBR_param_.dblLink7CogY*cos(q7) + KUKA_LBR_param_.dblLink7CogX*sin(q7)) + sin(q5)*(KUKA_LBR_param_.dblLink7CogX*cos(q7) - KUKA_LBR_param_.dblLink7CogY*sin(q7)))))));
dblMassInertFullRow6Col1 = -(KUKA_LBR_param_.dblLink6InertXZ*cos(q3)*cos(q5)*sin(q1)) - KUKA_LBR_param_.dblLink6CogX*KUKA_LBR_param_.dblLink6CogZ*KUKA_LBR_param_.dblLink6Mass*cos(q3)*cos(q4)*cos(q5)*cos(q6)*sin(q2) + KUKA_LBR_param_.dblLink6InertZZ*cos(q5)*sin(q2)*sin(q3) + power(KUKA_LBR_param_.dblLink6CogX,2)*KUKA_LBR_param_.dblLink6Mass*cos(q5)*sin(q2)*sin(q3) + power(KUKA_LBR_param_.dblLink6CogY,2)*KUKA_LBR_param_.dblLink6Mass*cos(q5)*sin(q2)*sin(q3) + KUKA_LBR_param_.dblLink45Len*KUKA_LBR_param_.dblLink6CogY*KUKA_LBR_param_.dblLink6Mass*cos(q5)*cos(q6)*sin(q2)*sin(q3) + KUKA_LBR_param_.dblLink23Len*KUKA_LBR_param_.dblLink6CogY*KUKA_LBR_param_.dblLink6Mass*cos(q4)*cos(q5)*cos(q6)*sin(q2)*sin(q3) - KUKA_LBR_param_.dblLink6CogY*KUKA_LBR_param_.dblLink6CogZ*KUKA_LBR_param_.dblLink6Mass*cos(q3)*cos(q6)*sin(q2)*sin(q4) - KUKA_LBR_param_.dblLink23Len*KUKA_LBR_param_.dblLink6CogX*KUKA_LBR_param_.dblLink6Mass*cos(q6)*sin(q2)*sin(q3)*sin(q4) + KUKA_LBR_param_.dblLink6InertZZ*cos(q3)*cos(q4)*sin(q2)*sin(q5) + power(KUKA_LBR_param_.dblLink6CogX,2)*KUKA_LBR_param_.dblLink6Mass*cos(q3)*cos(q4)*sin(q2)*sin(q5) + power(KUKA_LBR_param_.dblLink6CogY,2)*KUKA_LBR_param_.dblLink6Mass*cos(q3)*cos(q4)*sin(q2)*sin(q5) + KUKA_LBR_param_.dblLink23Len*KUKA_LBR_param_.dblLink6CogY*KUKA_LBR_param_.dblLink6Mass*cos(q3)*cos(q6)*sin(q2)*sin(q5) + KUKA_LBR_param_.dblLink45Len*KUKA_LBR_param_.dblLink6CogY*KUKA_LBR_param_.dblLink6Mass*cos(q3)*cos(q4)*cos(q6)*sin(q2)*sin(q5) + KUKA_LBR_param_.dblLink6InertXZ*cos(q4)*sin(q1)*sin(q3)*sin(q5) + KUKA_LBR_param_.dblLink6CogX*KUKA_LBR_param_.dblLink6CogZ*KUKA_LBR_param_.dblLink6Mass*cos(q6)*sin(q2)*sin(q3)*sin(q5) - KUKA_LBR_param_.dblLink6InertYZ*sin(q1)*sin(q2)*sin(q4)*sin(q5) + KUKA_LBR_param_.dblLink7InertZZ*(cos(q5)*sin(q2)*sin(q3) + (cos(q3)*cos(q4)*sin(q2) - cos(q2)*sin(q4))*sin(q5)) + KUKA_LBR_param_.dblLink7InertXZ*(-(cos(q5)*(cos(q3)*sin(q1) + cos(q1)*cos(q2)*sin(q3))) + (cos(q4)*sin(q1)*sin(q3) - cos(q1)*(cos(q2)*cos(q3)*cos(q4) + sin(q2)*sin(q4)))*sin(q5)) - cos(q1)*(KUKA_LBR_param_.dblLink6InertXZ*cos(q2)*cos(q5)*sin(q3) + (KUKA_LBR_param_.dblLink6InertYZ*cos(q4)*sin(q3) + KUKA_LBR_param_.dblLink6InertXZ*sin(q2)*sin(q4))*sin(q5) + cos(q3)*(-(KUKA_LBR_param_.dblLink6InertYZ*cos(q5)) + KUKA_LBR_param_.dblLink6InertXZ*cos(q2)*cos(q4)*sin(q5))) + KUKA_LBR_param_.dblLink7InertYZ*(cos(q1)*(cos(q3)*cos(q5) - cos(q4)*sin(q3)*sin(q5)) - sin(q1)*(sin(q2)*sin(q4)*sin(q5) + cos(q2)*(cos(q5)*sin(q3) + cos(q3)*cos(q4)*sin(q5)))) + KUKA_LBR_param_.dblLink6CogY*KUKA_LBR_param_.dblLink6CogZ*KUKA_LBR_param_.dblLink6Mass*cos(q3)*cos(q4)*cos(q5)*sin(q2)*sin(q6) + KUKA_LBR_param_.dblLink45Len*KUKA_LBR_param_.dblLink6CogX*KUKA_LBR_param_.dblLink6Mass*cos(q5)*sin(q2)*sin(q3)*sin(q6) + KUKA_LBR_param_.dblLink23Len*KUKA_LBR_param_.dblLink6CogX*KUKA_LBR_param_.dblLink6Mass*cos(q4)*cos(q5)*sin(q2)*sin(q3)*sin(q6) - KUKA_LBR_param_.dblLink6CogX*KUKA_LBR_param_.dblLink6CogZ*KUKA_LBR_param_.dblLink6Mass*cos(q3)*sin(q2)*sin(q4)*sin(q6) + KUKA_LBR_param_.dblLink23Len*KUKA_LBR_param_.dblLink6CogY*KUKA_LBR_param_.dblLink6Mass*sin(q2)*sin(q3)*sin(q4)*sin(q6) + KUKA_LBR_param_.dblLink23Len*KUKA_LBR_param_.dblLink6CogX*KUKA_LBR_param_.dblLink6Mass*cos(q3)*sin(q2)*sin(q5)*sin(q6) + KUKA_LBR_param_.dblLink45Len*KUKA_LBR_param_.dblLink6CogX*KUKA_LBR_param_.dblLink6Mass*cos(q3)*cos(q4)*sin(q2)*sin(q5)*sin(q6) - KUKA_LBR_param_.dblLink6CogY*KUKA_LBR_param_.dblLink6CogZ*KUKA_LBR_param_.dblLink6Mass*sin(q2)*sin(q3)*sin(q5)*sin(q6) - cos(q2)*(sin(q4)*sin(q5)*(KUKA_LBR_param_.dblLink6InertZZ + power(KUKA_LBR_param_.dblLink6CogX,2)*KUKA_LBR_param_.dblLink6Mass + power(KUKA_LBR_param_.dblLink6CogY,2)*KUKA_LBR_param_.dblLink6Mass + KUKA_LBR_param_.dblLink45Len*KUKA_LBR_param_.dblLink6CogY*KUKA_LBR_param_.dblLink6Mass*cos(q6) + KUKA_LBR_param_.dblLink45Len*KUKA_LBR_param_.dblLink6CogX*KUKA_LBR_param_.dblLink6Mass*sin(q6)) + cos(q4)*(KUKA_LBR_param_.dblLink6CogY*KUKA_LBR_param_.dblLink6CogZ*KUKA_LBR_param_.dblLink6Mass*cos(q6) + KUKA_LBR_param_.dblLink6InertYZ*cos(q3)*sin(q1)*sin(q5) + KUKA_LBR_param_.dblLink6CogX*KUKA_LBR_param_.dblLink6CogZ*KUKA_LBR_param_.dblLink6Mass*sin(q6)) + cos(q5)*(KUKA_LBR_param_.dblLink6InertYZ*sin(q1)*sin(q3) + KUKA_LBR_param_.dblLink6CogZ*KUKA_LBR_param_.dblLink6Mass*sin(q4)*(-(KUKA_LBR_param_.dblLink6CogX*cos(q6)) + KUKA_LBR_param_.dblLink6CogY*sin(q6)))) - KUKA_LBR_param_.dblLink7Mass*(sin(q1)*(cos(q6)*(-(KUKA_LBR_param_.dblLink7CogX*cos(q7)*sin(q3)*sin(q4)) + KUKA_LBR_param_.dblLink7CogZ*cos(q3)*sin(q5) + KUKA_LBR_param_.dblLink7CogY*sin(q3)*sin(q4)*sin(q7)) + sin(q6)*(KUKA_LBR_param_.dblLink7CogZ*sin(q3)*sin(q4) + cos(q3)*sin(q5)*(KUKA_LBR_param_.dblLink7CogX*cos(q7) - KUKA_LBR_param_.dblLink7CogY*sin(q7))) + cos(q4)*cos(q5)*sin(q3)*(KUKA_LBR_param_.dblLink7CogZ*cos(q6) + sin(q6)*(KUKA_LBR_param_.dblLink7CogX*cos(q7) - KUKA_LBR_param_.dblLink7CogY*sin(q7)))) - cos(q1)*(sin(q2)*(cos(q4)*(KUKA_LBR_param_.dblLink7CogX*cos(q6)*cos(q7) - KUKA_LBR_param_.dblLink7CogZ*sin(q6) - KUKA_LBR_param_.dblLink7CogY*cos(q6)*sin(q7)) + cos(q5)*sin(q4)*(KUKA_LBR_param_.dblLink7CogZ*cos(q6) + KUKA_LBR_param_.dblLink7CogX*cos(q7)*sin(q6) - KUKA_LBR_param_.dblLink7CogY*sin(q6)*sin(q7))) + cos(q2)*(-(sin(q3)*sin(q5)*(KUKA_LBR_param_.dblLink7CogZ*cos(q6) + sin(q6)*(KUKA_LBR_param_.dblLink7CogX*cos(q7) - KUKA_LBR_param_.dblLink7CogY*sin(q7)))) + cos(q3)*(sin(q4)*(-(KUKA_LBR_param_.dblLink7CogX*cos(q6)*cos(q7)) + KUKA_LBR_param_.dblLink7CogZ*sin(q6) + KUKA_LBR_param_.dblLink7CogY*cos(q6)*sin(q7)) + cos(q4)*cos(q5)*(KUKA_LBR_param_.dblLink7CogZ*cos(q6) + KUKA_LBR_param_.dblLink7CogX*cos(q7)*sin(q6) - KUKA_LBR_param_.dblLink7CogY*sin(q6)*sin(q7))))))*(cos(q1)*(cos(q3)*(cos(q5)*(KUKA_LBR_param_.dblLink7CogY*cos(q7) + KUKA_LBR_param_.dblLink7CogX*sin(q7)) + sin(q5)*(KUKA_LBR_param_.dblLink7CogX*cos(q6)*cos(q7) - KUKA_LBR_param_.dblLink7CogZ*sin(q6) - KUKA_LBR_param_.dblLink7CogY*cos(q6)*sin(q7))) + sin(q3)*(sin(q4)*(KUKA_LBR_param_.dblLink45Len + KUKA_LBR_param_.dblLink7CogZ*cos(q6) + KUKA_LBR_param_.dblLink7CogX*cos(q7)*sin(q6) - KUKA_LBR_param_.dblLink7CogY*sin(q6)*sin(q7)) - cos(q4)*(sin(q5)*(KUKA_LBR_param_.dblLink7CogY*cos(q7) + KUKA_LBR_param_.dblLink7CogX*sin(q7)) + cos(q5)*(-(KUKA_LBR_param_.dblLink7CogX*cos(q6)*cos(q7)) + KUKA_LBR_param_.dblLink7CogZ*sin(q6) + KUKA_LBR_param_.dblLink7CogY*cos(q6)*sin(q7))))) + sin(q1)*(-(sin(q2)*(KUKA_LBR_param_.dblLink23Len + KUKA_LBR_param_.dblLink7CogY*cos(q7)*sin(q4)*sin(q5) + KUKA_LBR_param_.dblLink7CogX*sin(q4)*sin(q5)*sin(q7) + cos(q5)*sin(q4)*(-(KUKA_LBR_param_.dblLink7CogX*cos(q6)*cos(q7)) + KUKA_LBR_param_.dblLink7CogZ*sin(q6) + KUKA_LBR_param_.dblLink7CogY*cos(q6)*sin(q7)) + cos(q4)*(KUKA_LBR_param_.dblLink45Len + KUKA_LBR_param_.dblLink7CogZ*cos(q6) + KUKA_LBR_param_.dblLink7CogX*cos(q7)*sin(q6) - KUKA_LBR_param_.dblLink7CogY*sin(q6)*sin(q7)))) + cos(q2)*(-(sin(q3)*(cos(q5)*(KUKA_LBR_param_.dblLink7CogY*cos(q7) + KUKA_LBR_param_.dblLink7CogX*sin(q7)) + sin(q5)*(KUKA_LBR_param_.dblLink7CogX*cos(q6)*cos(q7) - KUKA_LBR_param_.dblLink7CogZ*sin(q6) - KUKA_LBR_param_.dblLink7CogY*cos(q6)*sin(q7)))) + cos(q3)*(sin(q4)*(KUKA_LBR_param_.dblLink45Len + KUKA_LBR_param_.dblLink7CogZ*cos(q6) + KUKA_LBR_param_.dblLink7CogX*cos(q7)*sin(q6) - KUKA_LBR_param_.dblLink7CogY*sin(q6)*sin(q7)) - cos(q4)*(sin(q5)*(KUKA_LBR_param_.dblLink7CogY*cos(q7) + KUKA_LBR_param_.dblLink7CogX*sin(q7)) + cos(q5)*(-(KUKA_LBR_param_.dblLink7CogX*cos(q6)*cos(q7)) + KUKA_LBR_param_.dblLink7CogZ*sin(q6) + KUKA_LBR_param_.dblLink7CogY*cos(q6)*sin(q7))))))) + KUKA_LBR_param_.dblLink7Mass*(KUKA_LBR_param_.dblLink7CogZ*cos(q5)*cos(q6)*sin(q1)*sin(q2)*sin(q4) - KUKA_LBR_param_.dblLink7CogX*cos(q1)*cos(q6)*cos(q7)*sin(q3)*sin(q4) + KUKA_LBR_param_.dblLink7CogZ*cos(q1)*cos(q3)*cos(q6)*sin(q5) + KUKA_LBR_param_.dblLink7CogX*cos(q5)*cos(q7)*sin(q1)*sin(q2)*sin(q4)*sin(q6) + KUKA_LBR_param_.dblLink7CogZ*cos(q1)*sin(q3)*sin(q4)*sin(q6) + KUKA_LBR_param_.dblLink7CogX*cos(q1)*cos(q3)*cos(q7)*sin(q5)*sin(q6) + KUKA_LBR_param_.dblLink7CogY*cos(q1)*cos(q6)*sin(q3)*sin(q4)*sin(q7) - KUKA_LBR_param_.dblLink7CogY*cos(q5)*sin(q1)*sin(q2)*sin(q4)*sin(q6)*sin(q7) - KUKA_LBR_param_.dblLink7CogY*cos(q1)*cos(q3)*sin(q5)*sin(q6)*sin(q7) + cos(q4)*(cos(q6)*(KUKA_LBR_param_.dblLink7CogX*cos(q7)*sin(q1)*sin(q2) + KUKA_LBR_param_.dblLink7CogZ*cos(q1)*cos(q5)*sin(q3) - KUKA_LBR_param_.dblLink7CogY*sin(q1)*sin(q2)*sin(q7)) - sin(q6)*(KUKA_LBR_param_.dblLink7CogZ*sin(q1)*sin(q2) + cos(q1)*cos(q5)*sin(q3)*(-(KUKA_LBR_param_.dblLink7CogX*cos(q7)) + KUKA_LBR_param_.dblLink7CogY*sin(q7)))) + cos(q2)*sin(q1)*(-(sin(q3)*sin(q5)*(KUKA_LBR_param_.dblLink7CogZ*cos(q6) + sin(q6)*(KUKA_LBR_param_.dblLink7CogX*cos(q7) - KUKA_LBR_param_.dblLink7CogY*sin(q7)))) + cos(q3)*(sin(q4)*(-(KUKA_LBR_param_.dblLink7CogX*cos(q6)*cos(q7)) + KUKA_LBR_param_.dblLink7CogZ*sin(q6) + KUKA_LBR_param_.dblLink7CogY*cos(q6)*sin(q7)) + cos(q4)*cos(q5)*(KUKA_LBR_param_.dblLink7CogZ*cos(q6) + KUKA_LBR_param_.dblLink7CogX*cos(q7)*sin(q6) - KUKA_LBR_param_.dblLink7CogY*sin(q6)*sin(q7)))))*(sin(q1)*(cos(q3)*(cos(q5)*(KUKA_LBR_param_.dblLink7CogY*cos(q7) + KUKA_LBR_param_.dblLink7CogX*sin(q7)) + sin(q5)*(KUKA_LBR_param_.dblLink7CogX*cos(q6)*cos(q7) - KUKA_LBR_param_.dblLink7CogZ*sin(q6) - KUKA_LBR_param_.dblLink7CogY*cos(q6)*sin(q7))) + sin(q3)*(sin(q4)*(KUKA_LBR_param_.dblLink45Len + KUKA_LBR_param_.dblLink7CogZ*cos(q6) + KUKA_LBR_param_.dblLink7CogX*cos(q7)*sin(q6) - KUKA_LBR_param_.dblLink7CogY*sin(q6)*sin(q7)) - cos(q4)*(sin(q5)*(KUKA_LBR_param_.dblLink7CogY*cos(q7) + KUKA_LBR_param_.dblLink7CogX*sin(q7)) + cos(q5)*(-(KUKA_LBR_param_.dblLink7CogX*cos(q6)*cos(q7)) + KUKA_LBR_param_.dblLink7CogZ*sin(q6) + KUKA_LBR_param_.dblLink7CogY*cos(q6)*sin(q7))))) + cos(q1)*(sin(q2)*(KUKA_LBR_param_.dblLink23Len + KUKA_LBR_param_.dblLink7CogY*cos(q7)*sin(q4)*sin(q5) + KUKA_LBR_param_.dblLink7CogX*sin(q4)*sin(q5)*sin(q7) + cos(q5)*sin(q4)*(-(KUKA_LBR_param_.dblLink7CogX*cos(q6)*cos(q7)) + KUKA_LBR_param_.dblLink7CogZ*sin(q6) + KUKA_LBR_param_.dblLink7CogY*cos(q6)*sin(q7)) + cos(q4)*(KUKA_LBR_param_.dblLink45Len + KUKA_LBR_param_.dblLink7CogZ*cos(q6) + KUKA_LBR_param_.dblLink7CogX*cos(q7)*sin(q6) - KUKA_LBR_param_.dblLink7CogY*sin(q6)*sin(q7))) + cos(q2)*(sin(q3)*(cos(q5)*(KUKA_LBR_param_.dblLink7CogY*cos(q7) + KUKA_LBR_param_.dblLink7CogX*sin(q7)) + sin(q5)*(KUKA_LBR_param_.dblLink7CogX*cos(q6)*cos(q7) - KUKA_LBR_param_.dblLink7CogZ*sin(q6) - KUKA_LBR_param_.dblLink7CogY*cos(q6)*sin(q7))) + cos(q3)*(-(sin(q4)*(KUKA_LBR_param_.dblLink45Len + KUKA_LBR_param_.dblLink7CogZ*cos(q6) + KUKA_LBR_param_.dblLink7CogX*cos(q7)*sin(q6) - KUKA_LBR_param_.dblLink7CogY*sin(q6)*sin(q7))) + cos(q4)*(sin(q5)*(KUKA_LBR_param_.dblLink7CogY*cos(q7) + KUKA_LBR_param_.dblLink7CogX*sin(q7)) + cos(q5)*(-(KUKA_LBR_param_.dblLink7CogX*cos(q6)*cos(q7)) + KUKA_LBR_param_.dblLink7CogZ*sin(q6) + KUKA_LBR_param_.dblLink7CogY*cos(q6)*sin(q7)))))));
dblMassInertFullRow6Col2 = -(sin(q1)*(KUKA_LBR_param_.dblLink7InertXZ*(cos(q5)*sin(q2)*sin(q3) + (cos(q3)*cos(q4)*sin(q2) - cos(q2)*sin(q4))*sin(q5)) + KUKA_LBR_param_.dblLink7InertXX*(-(cos(q5)*(cos(q3)*sin(q1) + cos(q1)*cos(q2)*sin(q3))) + (cos(q4)*sin(q1)*sin(q3) - cos(q1)*(cos(q2)*cos(q3)*cos(q4) + sin(q2)*sin(q4)))*sin(q5)) + KUKA_LBR_param_.dblLink7InertXY*(cos(q1)*(cos(q3)*cos(q5) - cos(q4)*sin(q3)*sin(q5)) - sin(q1)*(sin(q2)*sin(q4)*sin(q5) + cos(q2)*(cos(q5)*sin(q3) + cos(q3)*cos(q4)*sin(q5)))))) + cos(q1)*(KUKA_LBR_param_.dblLink7InertYZ*(cos(q5)*sin(q2)*sin(q3) + (cos(q3)*cos(q4)*sin(q2) - cos(q2)*sin(q4))*sin(q5)) + KUKA_LBR_param_.dblLink7InertXY*(-(cos(q5)*(cos(q3)*sin(q1) + cos(q1)*cos(q2)*sin(q3))) + (cos(q4)*sin(q1)*sin(q3) - cos(q1)*(cos(q2)*cos(q3)*cos(q4) + sin(q2)*sin(q4)))*sin(q5)) + KUKA_LBR_param_.dblLink7InertYY*(cos(q1)*(cos(q3)*cos(q5) - cos(q4)*sin(q3)*sin(q5)) - sin(q1)*(sin(q2)*sin(q4)*sin(q5) + cos(q2)*(cos(q5)*sin(q3) + cos(q3)*cos(q4)*sin(q5))))) + (2*KUKA_LBR_param_.dblLink6CogX*KUKA_LBR_param_.dblLink6CogZ*KUKA_LBR_param_.dblLink6Mass*cos(q4)*cos(q5)*cos(q6)*sin(q3) + 2*KUKA_LBR_param_.dblLink6InertXY*cos(q2)*cos(q5)*power(sin(q1),2)*sin(q3) + KUKA_LBR_param_.dblLink6InertXX*cos(q2)*cos(q5)*sin(2*q1)*sin(q3) - 2*KUKA_LBR_param_.dblLink6InertXZ*cos(q5)*sin(q1)*sin(q2)*sin(q3) + 2*KUKA_LBR_param_.dblLink6CogY*KUKA_LBR_param_.dblLink6CogZ*KUKA_LBR_param_.dblLink6Mass*cos(q6)*sin(q3)*sin(q4) - KUKA_LBR_param_.dblLink6InertXX*cos(q4)*sin(q3)*sin(q5) - KUKA_LBR_param_.dblLink6InertYY*cos(q4)*sin(q3)*sin(q5) - 2*power(KUKA_LBR_param_.dblLink6CogX,2)*KUKA_LBR_param_.dblLink6Mass*cos(q4)*sin(q3)*sin(q5) - 2*power(KUKA_LBR_param_.dblLink6CogY,2)*KUKA_LBR_param_.dblLink6Mass*cos(q4)*sin(q3)*sin(q5) - 2*KUKA_LBR_param_.dblLink23Len*KUKA_LBR_param_.dblLink6CogY*KUKA_LBR_param_.dblLink6Mass*cos(q6)*sin(q3)*sin(q5) - 2*KUKA_LBR_param_.dblLink45Len*KUKA_LBR_param_.dblLink6CogY*KUKA_LBR_param_.dblLink6Mass*cos(q4)*cos(q6)*sin(q3)*sin(q5) - KUKA_LBR_param_.dblLink6InertXX*cos(q4)*power(sin(q1),2)*sin(q3)*sin(q5) + KUKA_LBR_param_.dblLink6InertYY*cos(q4)*power(sin(q1),2)*sin(q3)*sin(q5) + 2*KUKA_LBR_param_.dblLink6InertXZ*cos(q2)*sin(q1)*sin(q4)*sin(q5) + 2*KUKA_LBR_param_.dblLink6InertXY*power(sin(q1),2)*sin(q2)*sin(q4)*sin(q5) + KUKA_LBR_param_.dblLink6InertXX*sin(2*q1)*sin(q2)*sin(q4)*sin(q5) - power(cos(q1),2)*(2*KUKA_LBR_param_.dblLink6InertXY*cos(q2)*cos(q5)*sin(q3) + (-((KUKA_LBR_param_.dblLink6InertXX - KUKA_LBR_param_.dblLink6InertYY)*cos(q4)*sin(q3)) + 2*KUKA_LBR_param_.dblLink6InertXY*sin(q2)*sin(q4))*sin(q5)) - 2*cos(q1)*(-(KUKA_LBR_param_.dblLink6InertYZ*cos(q5)*sin(q2)*sin(q3)) + sin(q1)*(-2*KUKA_LBR_param_.dblLink6InertXY*cos(q4)*sin(q3) + KUKA_LBR_param_.dblLink6InertYY*sin(q2)*sin(q4))*sin(q5) + cos(q2)*(KUKA_LBR_param_.dblLink6InertYY*cos(q5)*sin(q1)*sin(q3) + KUKA_LBR_param_.dblLink6InertYZ*sin(q4)*sin(q5))) - 2*KUKA_LBR_param_.dblLink6CogY*KUKA_LBR_param_.dblLink6CogZ*KUKA_LBR_param_.dblLink6Mass*cos(q4)*cos(q5)*sin(q3)*sin(q6) + 2*KUKA_LBR_param_.dblLink6CogX*KUKA_LBR_param_.dblLink6CogZ*KUKA_LBR_param_.dblLink6Mass*sin(q3)*sin(q4)*sin(q6) - 2*KUKA_LBR_param_.dblLink23Len*KUKA_LBR_param_.dblLink6CogX*KUKA_LBR_param_.dblLink6Mass*sin(q3)*sin(q5)*sin(q6) - 2*KUKA_LBR_param_.dblLink45Len*KUKA_LBR_param_.dblLink6CogX*KUKA_LBR_param_.dblLink6Mass*cos(q4)*sin(q3)*sin(q5)*sin(q6) + cos(q3)*(cos(q5)*(KUKA_LBR_param_.dblLink6InertXX + KUKA_LBR_param_.dblLink6InertYY + 2*power(KUKA_LBR_param_.dblLink6CogX,2)*KUKA_LBR_param_.dblLink6Mass + 2*power(KUKA_LBR_param_.dblLink6CogY,2)*KUKA_LBR_param_.dblLink6Mass + (-KUKA_LBR_param_.dblLink6InertXX + KUKA_LBR_param_.dblLink6InertYY)*power(cos(q1),2) + 2*KUKA_LBR_param_.dblLink6CogY*KUKA_LBR_param_.dblLink6Mass*(KUKA_LBR_param_.dblLink45Len + KUKA_LBR_param_.dblLink23Len*cos(q4))*cos(q6) - 4*KUKA_LBR_param_.dblLink6InertXY*cos(q1)*sin(q1) + KUKA_LBR_param_.dblLink6InertXX*power(sin(q1),2) - KUKA_LBR_param_.dblLink6InertYY*power(sin(q1),2) + 2*KUKA_LBR_param_.dblLink45Len*KUKA_LBR_param_.dblLink6CogX*KUKA_LBR_param_.dblLink6Mass*sin(q6) + 2*KUKA_LBR_param_.dblLink23Len*KUKA_LBR_param_.dblLink6CogX*KUKA_LBR_param_.dblLink6Mass*cos(q4)*sin(q6)) - 2*(KUKA_LBR_param_.dblLink6InertXY*power(cos(q1),2)*cos(q2)*cos(q4)*sin(q5) - KUKA_LBR_param_.dblLink6InertXY*cos(q2)*cos(q4)*power(sin(q1),2)*sin(q5) + KUKA_LBR_param_.dblLink6InertXZ*cos(q4)*sin(q1)*sin(q2)*sin(q5) - cos(q1)*cos(q4)*((KUKA_LBR_param_.dblLink6InertXX - KUKA_LBR_param_.dblLink6InertYY)*cos(q2)*sin(q1) + KUKA_LBR_param_.dblLink6InertYZ*sin(q2))*sin(q5) + KUKA_LBR_param_.dblLink6CogX*KUKA_LBR_param_.dblLink6Mass*cos(q6)*(KUKA_LBR_param_.dblLink23Len*sin(q4) - KUKA_LBR_param_.dblLink6CogZ*sin(q5)) - KUKA_LBR_param_.dblLink23Len*KUKA_LBR_param_.dblLink6CogY*KUKA_LBR_param_.dblLink6Mass*sin(q4)*sin(q6) + KUKA_LBR_param_.dblLink6CogY*KUKA_LBR_param_.dblLink6CogZ*KUKA_LBR_param_.dblLink6Mass*sin(q5)*sin(q6))))/2.0 + KUKA_LBR_param_.dblLink7Mass*(cos(q2)*(cos(q4)*(KUKA_LBR_param_.dblLink7CogX*cos(q6)*cos(q7) - KUKA_LBR_param_.dblLink7CogZ*sin(q6) - KUKA_LBR_param_.dblLink7CogY*cos(q6)*sin(q7)) + cos(q5)*sin(q4)*(KUKA_LBR_param_.dblLink7CogZ*cos(q6) + KUKA_LBR_param_.dblLink7CogX*cos(q7)*sin(q6) - KUKA_LBR_param_.dblLink7CogY*sin(q6)*sin(q7))) - sin(q2)*(-(sin(q3)*sin(q5)*(KUKA_LBR_param_.dblLink7CogZ*cos(q6) + sin(q6)*(KUKA_LBR_param_.dblLink7CogX*cos(q7) - KUKA_LBR_param_.dblLink7CogY*sin(q7)))) + cos(q3)*(sin(q4)*(-(KUKA_LBR_param_.dblLink7CogX*cos(q6)*cos(q7)) + KUKA_LBR_param_.dblLink7CogZ*sin(q6) + KUKA_LBR_param_.dblLink7CogY*cos(q6)*sin(q7)) + cos(q4)*cos(q5)*(KUKA_LBR_param_.dblLink7CogZ*cos(q6) + KUKA_LBR_param_.dblLink7CogX*cos(q7)*sin(q6) - KUKA_LBR_param_.dblLink7CogY*sin(q6)*sin(q7)))))*(-(sin(q2)*(KUKA_LBR_param_.dblLink23Len + KUKA_LBR_param_.dblLink7CogY*cos(q7)*sin(q4)*sin(q5) + KUKA_LBR_param_.dblLink7CogX*sin(q4)*sin(q5)*sin(q7) + cos(q5)*sin(q4)*(-(KUKA_LBR_param_.dblLink7CogX*cos(q6)*cos(q7)) + KUKA_LBR_param_.dblLink7CogZ*sin(q6) + KUKA_LBR_param_.dblLink7CogY*cos(q6)*sin(q7)) + cos(q4)*(KUKA_LBR_param_.dblLink45Len + KUKA_LBR_param_.dblLink7CogZ*cos(q6) + KUKA_LBR_param_.dblLink7CogX*cos(q7)*sin(q6) - KUKA_LBR_param_.dblLink7CogY*sin(q6)*sin(q7)))) + cos(q2)*(-(sin(q3)*(cos(q5)*(KUKA_LBR_param_.dblLink7CogY*cos(q7) + KUKA_LBR_param_.dblLink7CogX*sin(q7)) + sin(q5)*(KUKA_LBR_param_.dblLink7CogX*cos(q6)*cos(q7) - KUKA_LBR_param_.dblLink7CogZ*sin(q6) - KUKA_LBR_param_.dblLink7CogY*cos(q6)*sin(q7)))) + cos(q3)*(sin(q4)*(KUKA_LBR_param_.dblLink45Len + KUKA_LBR_param_.dblLink7CogZ*cos(q6) + KUKA_LBR_param_.dblLink7CogX*cos(q7)*sin(q6) - KUKA_LBR_param_.dblLink7CogY*sin(q6)*sin(q7)) - cos(q4)*(sin(q5)*(KUKA_LBR_param_.dblLink7CogY*cos(q7) + KUKA_LBR_param_.dblLink7CogX*sin(q7)) + cos(q5)*(-(KUKA_LBR_param_.dblLink7CogX*cos(q6)*cos(q7)) + KUKA_LBR_param_.dblLink7CogZ*sin(q6) + KUKA_LBR_param_.dblLink7CogY*cos(q6)*sin(q7)))))) + KUKA_LBR_param_.dblLink7Mass*sin(q1)*(KUKA_LBR_param_.dblLink7CogZ*cos(q5)*cos(q6)*sin(q1)*sin(q2)*sin(q4) - KUKA_LBR_param_.dblLink7CogX*cos(q1)*cos(q6)*cos(q7)*sin(q3)*sin(q4) + KUKA_LBR_param_.dblLink7CogZ*cos(q1)*cos(q3)*cos(q6)*sin(q5) + KUKA_LBR_param_.dblLink7CogX*cos(q5)*cos(q7)*sin(q1)*sin(q2)*sin(q4)*sin(q6) + KUKA_LBR_param_.dblLink7CogZ*cos(q1)*sin(q3)*sin(q4)*sin(q6) + KUKA_LBR_param_.dblLink7CogX*cos(q1)*cos(q3)*cos(q7)*sin(q5)*sin(q6) + KUKA_LBR_param_.dblLink7CogY*cos(q1)*cos(q6)*sin(q3)*sin(q4)*sin(q7) - KUKA_LBR_param_.dblLink7CogY*cos(q5)*sin(q1)*sin(q2)*sin(q4)*sin(q6)*sin(q7) - KUKA_LBR_param_.dblLink7CogY*cos(q1)*cos(q3)*sin(q5)*sin(q6)*sin(q7) + cos(q4)*(cos(q6)*(KUKA_LBR_param_.dblLink7CogX*cos(q7)*sin(q1)*sin(q2) + KUKA_LBR_param_.dblLink7CogZ*cos(q1)*cos(q5)*sin(q3) - KUKA_LBR_param_.dblLink7CogY*sin(q1)*sin(q2)*sin(q7)) - sin(q6)*(KUKA_LBR_param_.dblLink7CogZ*sin(q1)*sin(q2) + cos(q1)*cos(q5)*sin(q3)*(-(KUKA_LBR_param_.dblLink7CogX*cos(q7)) + KUKA_LBR_param_.dblLink7CogY*sin(q7)))) + cos(q2)*sin(q1)*(-(sin(q3)*sin(q5)*(KUKA_LBR_param_.dblLink7CogZ*cos(q6) + sin(q6)*(KUKA_LBR_param_.dblLink7CogX*cos(q7) - KUKA_LBR_param_.dblLink7CogY*sin(q7)))) + cos(q3)*(sin(q4)*(-(KUKA_LBR_param_.dblLink7CogX*cos(q6)*cos(q7)) + KUKA_LBR_param_.dblLink7CogZ*sin(q6) + KUKA_LBR_param_.dblLink7CogY*cos(q6)*sin(q7)) + cos(q4)*cos(q5)*(KUKA_LBR_param_.dblLink7CogZ*cos(q6) + KUKA_LBR_param_.dblLink7CogX*cos(q7)*sin(q6) - KUKA_LBR_param_.dblLink7CogY*sin(q6)*sin(q7)))))*(cos(q2)*(KUKA_LBR_param_.dblLink23Len + KUKA_LBR_param_.dblLink7CogY*cos(q7)*sin(q4)*sin(q5) + KUKA_LBR_param_.dblLink7CogX*sin(q4)*sin(q5)*sin(q7) + cos(q5)*sin(q4)*(-(KUKA_LBR_param_.dblLink7CogX*cos(q6)*cos(q7)) + KUKA_LBR_param_.dblLink7CogZ*sin(q6) + KUKA_LBR_param_.dblLink7CogY*cos(q6)*sin(q7)) + cos(q4)*(KUKA_LBR_param_.dblLink45Len + KUKA_LBR_param_.dblLink7CogZ*cos(q6) + KUKA_LBR_param_.dblLink7CogX*cos(q7)*sin(q6) - KUKA_LBR_param_.dblLink7CogY*sin(q6)*sin(q7))) + sin(q2)*(-(sin(q3)*(cos(q5)*(KUKA_LBR_param_.dblLink7CogY*cos(q7) + KUKA_LBR_param_.dblLink7CogX*sin(q7)) + sin(q5)*(KUKA_LBR_param_.dblLink7CogX*cos(q6)*cos(q7) - KUKA_LBR_param_.dblLink7CogZ*sin(q6) - KUKA_LBR_param_.dblLink7CogY*cos(q6)*sin(q7)))) + cos(q3)*(sin(q4)*(KUKA_LBR_param_.dblLink45Len + KUKA_LBR_param_.dblLink7CogZ*cos(q6) + KUKA_LBR_param_.dblLink7CogX*cos(q7)*sin(q6) - KUKA_LBR_param_.dblLink7CogY*sin(q6)*sin(q7)) - cos(q4)*(sin(q5)*(KUKA_LBR_param_.dblLink7CogY*cos(q7) + KUKA_LBR_param_.dblLink7CogX*sin(q7)) + cos(q5)*(-(KUKA_LBR_param_.dblLink7CogX*cos(q6)*cos(q7)) + KUKA_LBR_param_.dblLink7CogZ*sin(q6) + KUKA_LBR_param_.dblLink7CogY*cos(q6)*sin(q7)))))) - KUKA_LBR_param_.dblLink7Mass*cos(q1)*(cos(q2)*(KUKA_LBR_param_.dblLink23Len + KUKA_LBR_param_.dblLink7CogY*cos(q7)*sin(q4)*sin(q5) + KUKA_LBR_param_.dblLink7CogX*sin(q4)*sin(q5)*sin(q7) + cos(q5)*sin(q4)*(-(KUKA_LBR_param_.dblLink7CogX*cos(q6)*cos(q7)) + KUKA_LBR_param_.dblLink7CogZ*sin(q6) + KUKA_LBR_param_.dblLink7CogY*cos(q6)*sin(q7)) + cos(q4)*(KUKA_LBR_param_.dblLink45Len + KUKA_LBR_param_.dblLink7CogZ*cos(q6) + KUKA_LBR_param_.dblLink7CogX*cos(q7)*sin(q6) - KUKA_LBR_param_.dblLink7CogY*sin(q6)*sin(q7))) + sin(q2)*(-(sin(q3)*(cos(q5)*(KUKA_LBR_param_.dblLink7CogY*cos(q7) + KUKA_LBR_param_.dblLink7CogX*sin(q7)) + sin(q5)*(KUKA_LBR_param_.dblLink7CogX*cos(q6)*cos(q7) - KUKA_LBR_param_.dblLink7CogZ*sin(q6) - KUKA_LBR_param_.dblLink7CogY*cos(q6)*sin(q7)))) + cos(q3)*(sin(q4)*(KUKA_LBR_param_.dblLink45Len + KUKA_LBR_param_.dblLink7CogZ*cos(q6) + KUKA_LBR_param_.dblLink7CogX*cos(q7)*sin(q6) - KUKA_LBR_param_.dblLink7CogY*sin(q6)*sin(q7)) - cos(q4)*(sin(q5)*(KUKA_LBR_param_.dblLink7CogY*cos(q7) + KUKA_LBR_param_.dblLink7CogX*sin(q7)) + cos(q5)*(-(KUKA_LBR_param_.dblLink7CogX*cos(q6)*cos(q7)) + KUKA_LBR_param_.dblLink7CogZ*sin(q6) + KUKA_LBR_param_.dblLink7CogY*cos(q6)*sin(q7))))))*(sin(q1)*(cos(q6)*(-(KUKA_LBR_param_.dblLink7CogX*cos(q7)*sin(q3)*sin(q4)) + KUKA_LBR_param_.dblLink7CogZ*cos(q3)*sin(q5) + KUKA_LBR_param_.dblLink7CogY*sin(q3)*sin(q4)*sin(q7)) + sin(q6)*(KUKA_LBR_param_.dblLink7CogZ*sin(q3)*sin(q4) + cos(q3)*sin(q5)*(KUKA_LBR_param_.dblLink7CogX*cos(q7) - KUKA_LBR_param_.dblLink7CogY*sin(q7))) + cos(q4)*cos(q5)*sin(q3)*(KUKA_LBR_param_.dblLink7CogZ*cos(q6) + sin(q6)*(KUKA_LBR_param_.dblLink7CogX*cos(q7) - KUKA_LBR_param_.dblLink7CogY*sin(q7)))) - cos(q1)*(sin(q2)*(cos(q4)*(KUKA_LBR_param_.dblLink7CogX*cos(q6)*cos(q7) - KUKA_LBR_param_.dblLink7CogZ*sin(q6) - KUKA_LBR_param_.dblLink7CogY*cos(q6)*sin(q7)) + cos(q5)*sin(q4)*(KUKA_LBR_param_.dblLink7CogZ*cos(q6) + KUKA_LBR_param_.dblLink7CogX*cos(q7)*sin(q6) - KUKA_LBR_param_.dblLink7CogY*sin(q6)*sin(q7))) + cos(q2)*(-(sin(q3)*sin(q5)*(KUKA_LBR_param_.dblLink7CogZ*cos(q6) + sin(q6)*(KUKA_LBR_param_.dblLink7CogX*cos(q7) - KUKA_LBR_param_.dblLink7CogY*sin(q7)))) + cos(q3)*(sin(q4)*(-(KUKA_LBR_param_.dblLink7CogX*cos(q6)*cos(q7)) + KUKA_LBR_param_.dblLink7CogZ*sin(q6) + KUKA_LBR_param_.dblLink7CogY*cos(q6)*sin(q7)) + cos(q4)*cos(q5)*(KUKA_LBR_param_.dblLink7CogZ*cos(q6) + KUKA_LBR_param_.dblLink7CogX*cos(q7)*sin(q6) - KUKA_LBR_param_.dblLink7CogY*sin(q6)*sin(q7))))));
dblMassInertFullRow6Col3 = cos(q1)*sin(q2)*(KUKA_LBR_param_.dblLink7InertXZ*(cos(q5)*sin(q2)*sin(q3) + (cos(q3)*cos(q4)*sin(q2) - cos(q2)*sin(q4))*sin(q5)) + KUKA_LBR_param_.dblLink7InertXX*(-(cos(q5)*(cos(q3)*sin(q1) + cos(q1)*cos(q2)*sin(q3))) + (cos(q4)*sin(q1)*sin(q3) - cos(q1)*(cos(q2)*cos(q3)*cos(q4) + sin(q2)*sin(q4)))*sin(q5)) + KUKA_LBR_param_.dblLink7InertXY*(cos(q1)*(cos(q3)*cos(q5) - cos(q4)*sin(q3)*sin(q5)) - sin(q1)*(sin(q2)*sin(q4)*sin(q5) + cos(q2)*(cos(q5)*sin(q3) + cos(q3)*cos(q4)*sin(q5))))) + sin(q1)*sin(q2)*(KUKA_LBR_param_.dblLink7InertYZ*(cos(q5)*sin(q2)*sin(q3) + (cos(q3)*cos(q4)*sin(q2) - cos(q2)*sin(q4))*sin(q5)) + KUKA_LBR_param_.dblLink7InertXY*(-(cos(q5)*(cos(q3)*sin(q1) + cos(q1)*cos(q2)*sin(q3))) + (cos(q4)*sin(q1)*sin(q3) - cos(q1)*(cos(q2)*cos(q3)*cos(q4) + sin(q2)*sin(q4)))*sin(q5)) + KUKA_LBR_param_.dblLink7InertYY*(cos(q1)*(cos(q3)*cos(q5) - cos(q4)*sin(q3)*sin(q5)) - sin(q1)*(sin(q2)*sin(q4)*sin(q5) + cos(q2)*(cos(q5)*sin(q3) + cos(q3)*cos(q4)*sin(q5))))) + cos(q2)*(KUKA_LBR_param_.dblLink7InertZZ*(cos(q5)*sin(q2)*sin(q3) + (cos(q3)*cos(q4)*sin(q2) - cos(q2)*sin(q4))*sin(q5)) + KUKA_LBR_param_.dblLink7InertXZ*(-(cos(q5)*(cos(q3)*sin(q1) + cos(q1)*cos(q2)*sin(q3))) + (cos(q4)*sin(q1)*sin(q3) - cos(q1)*(cos(q2)*cos(q3)*cos(q4) + sin(q2)*sin(q4)))*sin(q5)) + KUKA_LBR_param_.dblLink7InertYZ*(cos(q1)*(cos(q3)*cos(q5) - cos(q4)*sin(q3)*sin(q5)) - sin(q1)*(sin(q2)*sin(q4)*sin(q5) + cos(q2)*(cos(q5)*sin(q3) + cos(q3)*cos(q4)*sin(q5))))) + (-4*KUKA_LBR_param_.dblLink6InertXZ*cos(q2)*cos(q3)*cos(q5)*sin(q1) - 4*KUKA_LBR_param_.dblLink6InertXY*cos(q3)*cos(q5)*power(sin(q1),2)*sin(q2) - 4*KUKA_LBR_param_.dblLink6InertYZ*power(cos(q2),2)*cos(q5)*sin(q1)*sin(q3) - 2*KUKA_LBR_param_.dblLink6InertXX*cos(q2)*cos(q5)*sin(q2)*sin(q3) - 2*KUKA_LBR_param_.dblLink6InertYY*cos(q2)*cos(q5)*sin(q2)*sin(q3) + 4*KUKA_LBR_param_.dblLink6InertZZ*cos(q2)*cos(q5)*sin(q2)*sin(q3) - 2*KUKA_LBR_param_.dblLink6InertYY*cos(q2)*cos(q5)*power(sin(q1),2)*sin(q2)*sin(q3) + 4*KUKA_LBR_param_.dblLink6InertYZ*cos(q5)*sin(q1)*power(sin(q2),2)*sin(q3) + KUKA_LBR_param_.dblLink6InertXX*cos(q5)*power(sin(q1),2)*sin(2*q2)*sin(q3) + 4*KUKA_LBR_param_.dblLink6CogX*KUKA_LBR_param_.dblLink6CogZ*KUKA_LBR_param_.dblLink6Mass*cos(q5)*cos(q6)*sin(q4) - KUKA_LBR_param_.dblLink6InertXX*sin(q4)*sin(q5) - KUKA_LBR_param_.dblLink6InertYY*sin(q4)*sin(q5) - 2*KUKA_LBR_param_.dblLink6InertZZ*sin(q4)*sin(q5) - 4*power(KUKA_LBR_param_.dblLink6CogX,2)*KUKA_LBR_param_.dblLink6Mass*sin(q4)*sin(q5) - 4*power(KUKA_LBR_param_.dblLink6CogY,2)*KUKA_LBR_param_.dblLink6Mass*sin(q4)*sin(q5) + KUKA_LBR_param_.dblLink6InertXX*power(cos(q2),2)*sin(q4)*sin(q5) + KUKA_LBR_param_.dblLink6InertYY*power(cos(q2),2)*sin(q4)*sin(q5) - 2*KUKA_LBR_param_.dblLink6InertZZ*power(cos(q2),2)*sin(q4)*sin(q5) - 4*KUKA_LBR_param_.dblLink45Len*KUKA_LBR_param_.dblLink6CogY*KUKA_LBR_param_.dblLink6Mass*cos(q6)*sin(q4)*sin(q5) + KUKA_LBR_param_.dblLink6InertXX*power(sin(q1),2)*sin(q4)*sin(q5) - KUKA_LBR_param_.dblLink6InertYY*power(sin(q1),2)*sin(q4)*sin(q5) - KUKA_LBR_param_.dblLink6InertXX*power(cos(q2),2)*power(sin(q1),2)*sin(q4)*sin(q5) + KUKA_LBR_param_.dblLink6InertYY*power(cos(q2),2)*power(sin(q1),2)*sin(q4)*sin(q5) - 8*KUKA_LBR_param_.dblLink6InertYZ*cos(q2)*sin(q1)*sin(q2)*sin(q4)*sin(q5) - KUKA_LBR_param_.dblLink6InertXX*power(sin(q2),2)*sin(q4)*sin(q5) - KUKA_LBR_param_.dblLink6InertYY*power(sin(q2),2)*sin(q4)*sin(q5) + 2*KUKA_LBR_param_.dblLink6InertZZ*power(sin(q2),2)*sin(q4)*sin(q5) + KUKA_LBR_param_.dblLink6InertXX*power(sin(q1),2)*power(sin(q2),2)*sin(q4)*sin(q5) - KUKA_LBR_param_.dblLink6InertYY*power(sin(q1),2)*power(sin(q2),2)*sin(q4)*sin(q5) + power(cos(q1),2)*(-2*KUKA_LBR_param_.dblLink6InertXX*cos(q2)*cos(q5)*sin(q2)*sin(q3) + KUKA_LBR_param_.dblLink6InertYY*cos(q5)*sin(2*q2)*sin(q3) - 4*KUKA_LBR_param_.dblLink6InertXY*cos(q4)*sin(q2)*sin(q3)*sin(q5) - KUKA_LBR_param_.dblLink6InertXX*sin(q4)*sin(q5) + KUKA_LBR_param_.dblLink6InertYY*sin(q4)*sin(q5) + (KUKA_LBR_param_.dblLink6InertXX - KUKA_LBR_param_.dblLink6InertYY)*power(cos(q2),2)*sin(q4)*sin(q5) - KUKA_LBR_param_.dblLink6InertXX*power(sin(q2),2)*sin(q4)*sin(q5) + KUKA_LBR_param_.dblLink6InertYY*power(sin(q2),2)*sin(q4)*sin(q5) + cos(q3)*(4*KUKA_LBR_param_.dblLink6InertXY*cos(q5)*sin(q2) + (-KUKA_LBR_param_.dblLink6InertXX + KUKA_LBR_param_.dblLink6InertYY)*cos(q4)*sin(2*q2)*sin(q5))) + 4*cos(q1)*(KUKA_LBR_param_.dblLink6InertXZ*cos(q5)*power(sin(q2),2)*sin(q3) + KUKA_LBR_param_.dblLink6InertXX*cos(q4)*sin(q1)*sin(q2)*sin(q3)*sin(q5) - KUKA_LBR_param_.dblLink6InertYY*cos(q4)*sin(q1)*sin(q2)*sin(q3)*sin(q5) - KUKA_LBR_param_.dblLink6InertXY*sin(q1)*sin(q4)*sin(q5) - KUKA_LBR_param_.dblLink6InertXY*sin(q1)*power(sin(q2),2)*sin(q4)*sin(q5) + cos(q3)*sin(q2)*(-((KUKA_LBR_param_.dblLink6InertXX - KUKA_LBR_param_.dblLink6InertYY)*cos(q5)*sin(q1)) + KUKA_LBR_param_.dblLink6InertXZ*cos(q4)*sin(q2)*sin(q5)) - power(cos(q2),2)*(KUKA_LBR_param_.dblLink6InertXZ*cos(q5)*sin(q3) + (KUKA_LBR_param_.dblLink6InertXZ*cos(q3)*cos(q4) - KUKA_LBR_param_.dblLink6InertXY*sin(q1)*sin(q4))*sin(q5)) - cos(q2)*(2*KUKA_LBR_param_.dblLink6InertXY*cos(q5)*sin(q1)*sin(q2)*sin(q3) + KUKA_LBR_param_.dblLink6InertYZ*cos(q4)*sin(q3)*sin(q5) + 2*KUKA_LBR_param_.dblLink6InertXZ*sin(q2)*sin(q4)*sin(q5) + cos(q3)*(-(KUKA_LBR_param_.dblLink6InertYZ*cos(q5)) + 2*KUKA_LBR_param_.dblLink6InertXY*cos(q4)*sin(q1)*sin(q2)*sin(q5)))) - 4*KUKA_LBR_param_.dblLink6CogY*KUKA_LBR_param_.dblLink6CogZ*KUKA_LBR_param_.dblLink6Mass*cos(q5)*sin(q4)*sin(q6) - 4*KUKA_LBR_param_.dblLink45Len*KUKA_LBR_param_.dblLink6CogX*KUKA_LBR_param_.dblLink6Mass*sin(q4)*sin(q5)*sin(q6) + cos(q4)*(-4*KUKA_LBR_param_.dblLink6CogY*KUKA_LBR_param_.dblLink6CogZ*KUKA_LBR_param_.dblLink6Mass*cos(q6) - 4*KUKA_LBR_param_.dblLink6InertYZ*power(cos(q2),2)*cos(q3)*sin(q1)*sin(q5) + 4*KUKA_LBR_param_.dblLink6InertYZ*cos(q3)*sin(q1)*power(sin(q2),2)*sin(q5) + KUKA_LBR_param_.dblLink6InertXX*cos(q3)*power(sin(q1),2)*sin(2*q2)*sin(q5) + 4*KUKA_LBR_param_.dblLink6InertXY*power(sin(q1),2)*sin(q2)*sin(q3)*sin(q5) - 2*cos(q2)*(cos(q3)*(KUKA_LBR_param_.dblLink6InertXX + KUKA_LBR_param_.dblLink6InertYY - 2*KUKA_LBR_param_.dblLink6InertZZ + KUKA_LBR_param_.dblLink6InertYY*power(sin(q1),2))*sin(q2) - 2*KUKA_LBR_param_.dblLink6InertXZ*sin(q1)*sin(q3))*sin(q5) - 4*KUKA_LBR_param_.dblLink6CogX*KUKA_LBR_param_.dblLink6CogZ*KUKA_LBR_param_.dblLink6Mass*sin(q6)))/4.0 + KUKA_LBR_param_.dblLink7Mass*sin(q2)*(cos(q3)*(cos(q5)*(KUKA_LBR_param_.dblLink7CogY*cos(q7) + KUKA_LBR_param_.dblLink7CogX*sin(q7)) + sin(q5)*(KUKA_LBR_param_.dblLink7CogX*cos(q6)*cos(q7) - KUKA_LBR_param_.dblLink7CogZ*sin(q6) - KUKA_LBR_param_.dblLink7CogY*cos(q6)*sin(q7))) + sin(q3)*(sin(q4)*(KUKA_LBR_param_.dblLink45Len + KUKA_LBR_param_.dblLink7CogZ*cos(q6) + KUKA_LBR_param_.dblLink7CogX*cos(q7)*sin(q6) - KUKA_LBR_param_.dblLink7CogY*sin(q6)*sin(q7)) - cos(q4)*(sin(q5)*(KUKA_LBR_param_.dblLink7CogY*cos(q7) + KUKA_LBR_param_.dblLink7CogX*sin(q7)) + cos(q5)*(-(KUKA_LBR_param_.dblLink7CogX*cos(q6)*cos(q7)) + KUKA_LBR_param_.dblLink7CogZ*sin(q6) + KUKA_LBR_param_.dblLink7CogY*cos(q6)*sin(q7)))))*(cos(q2)*(cos(q4)*(-(KUKA_LBR_param_.dblLink7CogX*cos(q6)*cos(q7)) + KUKA_LBR_param_.dblLink7CogZ*sin(q6) + KUKA_LBR_param_.dblLink7CogY*cos(q6)*sin(q7)) - cos(q5)*sin(q4)*(KUKA_LBR_param_.dblLink7CogZ*cos(q6) + KUKA_LBR_param_.dblLink7CogX*cos(q7)*sin(q6) - KUKA_LBR_param_.dblLink7CogY*sin(q6)*sin(q7))) + sin(q2)*(-(sin(q3)*sin(q5)*(KUKA_LBR_param_.dblLink7CogZ*cos(q6) + sin(q6)*(KUKA_LBR_param_.dblLink7CogX*cos(q7) - KUKA_LBR_param_.dblLink7CogY*sin(q7)))) + cos(q3)*(sin(q4)*(-(KUKA_LBR_param_.dblLink7CogX*cos(q6)*cos(q7)) + KUKA_LBR_param_.dblLink7CogZ*sin(q6) + KUKA_LBR_param_.dblLink7CogY*cos(q6)*sin(q7)) + cos(q4)*cos(q5)*(KUKA_LBR_param_.dblLink7CogZ*cos(q6) + KUKA_LBR_param_.dblLink7CogX*cos(q7)*sin(q6) - KUKA_LBR_param_.dblLink7CogY*sin(q6)*sin(q7))))) + KUKA_LBR_param_.dblLink7Mass*(KUKA_LBR_param_.dblLink7CogZ*cos(q5)*cos(q6)*sin(q1)*sin(q2)*sin(q4) - KUKA_LBR_param_.dblLink7CogX*cos(q1)*cos(q6)*cos(q7)*sin(q3)*sin(q4) + KUKA_LBR_param_.dblLink7CogZ*cos(q1)*cos(q3)*cos(q6)*sin(q5) + KUKA_LBR_param_.dblLink7CogX*cos(q5)*cos(q7)*sin(q1)*sin(q2)*sin(q4)*sin(q6) + KUKA_LBR_param_.dblLink7CogZ*cos(q1)*sin(q3)*sin(q4)*sin(q6) + KUKA_LBR_param_.dblLink7CogX*cos(q1)*cos(q3)*cos(q7)*sin(q5)*sin(q6) + KUKA_LBR_param_.dblLink7CogY*cos(q1)*cos(q6)*sin(q3)*sin(q4)*sin(q7) - KUKA_LBR_param_.dblLink7CogY*cos(q5)*sin(q1)*sin(q2)*sin(q4)*sin(q6)*sin(q7) - KUKA_LBR_param_.dblLink7CogY*cos(q1)*cos(q3)*sin(q5)*sin(q6)*sin(q7) + cos(q4)*(cos(q6)*(KUKA_LBR_param_.dblLink7CogX*cos(q7)*sin(q1)*sin(q2) + KUKA_LBR_param_.dblLink7CogZ*cos(q1)*cos(q5)*sin(q3) - KUKA_LBR_param_.dblLink7CogY*sin(q1)*sin(q2)*sin(q7)) - sin(q6)*(KUKA_LBR_param_.dblLink7CogZ*sin(q1)*sin(q2) + cos(q1)*cos(q5)*sin(q3)*(-(KUKA_LBR_param_.dblLink7CogX*cos(q7)) + KUKA_LBR_param_.dblLink7CogY*sin(q7)))) + cos(q2)*sin(q1)*(-(sin(q3)*sin(q5)*(KUKA_LBR_param_.dblLink7CogZ*cos(q6) + sin(q6)*(KUKA_LBR_param_.dblLink7CogX*cos(q7) - KUKA_LBR_param_.dblLink7CogY*sin(q7)))) + cos(q3)*(sin(q4)*(-(KUKA_LBR_param_.dblLink7CogX*cos(q6)*cos(q7)) + KUKA_LBR_param_.dblLink7CogZ*sin(q6) + KUKA_LBR_param_.dblLink7CogY*cos(q6)*sin(q7)) + cos(q4)*cos(q5)*(KUKA_LBR_param_.dblLink7CogZ*cos(q6) + KUKA_LBR_param_.dblLink7CogX*cos(q7)*sin(q6) - KUKA_LBR_param_.dblLink7CogY*sin(q6)*sin(q7)))))*(cos(q2)*sin(q1)*(cos(q3)*(cos(q5)*(KUKA_LBR_param_.dblLink7CogY*cos(q7) + KUKA_LBR_param_.dblLink7CogX*sin(q7)) + sin(q5)*(KUKA_LBR_param_.dblLink7CogX*cos(q6)*cos(q7) - KUKA_LBR_param_.dblLink7CogZ*sin(q6) - KUKA_LBR_param_.dblLink7CogY*cos(q6)*sin(q7))) + sin(q3)*(sin(q4)*(KUKA_LBR_param_.dblLink45Len + KUKA_LBR_param_.dblLink7CogZ*cos(q6) + KUKA_LBR_param_.dblLink7CogX*cos(q7)*sin(q6) - KUKA_LBR_param_.dblLink7CogY*sin(q6)*sin(q7)) - cos(q4)*(sin(q5)*(KUKA_LBR_param_.dblLink7CogY*cos(q7) + KUKA_LBR_param_.dblLink7CogX*sin(q7)) + cos(q5)*(-(KUKA_LBR_param_.dblLink7CogX*cos(q6)*cos(q7)) + KUKA_LBR_param_.dblLink7CogZ*sin(q6) + KUKA_LBR_param_.dblLink7CogY*cos(q6)*sin(q7))))) + cos(q1)*(sin(q3)*(cos(q5)*(KUKA_LBR_param_.dblLink7CogY*cos(q7) + KUKA_LBR_param_.dblLink7CogX*sin(q7)) + sin(q5)*(KUKA_LBR_param_.dblLink7CogX*cos(q6)*cos(q7) - KUKA_LBR_param_.dblLink7CogZ*sin(q6) - KUKA_LBR_param_.dblLink7CogY*cos(q6)*sin(q7))) + cos(q3)*(-(sin(q4)*(KUKA_LBR_param_.dblLink45Len + KUKA_LBR_param_.dblLink7CogZ*cos(q6) + KUKA_LBR_param_.dblLink7CogX*cos(q7)*sin(q6) - KUKA_LBR_param_.dblLink7CogY*sin(q6)*sin(q7))) + cos(q4)*(sin(q5)*(KUKA_LBR_param_.dblLink7CogY*cos(q7) + KUKA_LBR_param_.dblLink7CogX*sin(q7)) + cos(q5)*(-(KUKA_LBR_param_.dblLink7CogX*cos(q6)*cos(q7)) + KUKA_LBR_param_.dblLink7CogZ*sin(q6) + KUKA_LBR_param_.dblLink7CogY*cos(q6)*sin(q7)))))) + KUKA_LBR_param_.dblLink7Mass*(sin(q1)*(-(sin(q3)*(cos(q5)*(KUKA_LBR_param_.dblLink7CogY*cos(q7) + KUKA_LBR_param_.dblLink7CogX*sin(q7)) + sin(q5)*(KUKA_LBR_param_.dblLink7CogX*cos(q6)*cos(q7) - KUKA_LBR_param_.dblLink7CogZ*sin(q6) - KUKA_LBR_param_.dblLink7CogY*cos(q6)*sin(q7)))) + cos(q3)*(sin(q4)*(KUKA_LBR_param_.dblLink45Len + KUKA_LBR_param_.dblLink7CogZ*cos(q6) + KUKA_LBR_param_.dblLink7CogX*cos(q7)*sin(q6) - KUKA_LBR_param_.dblLink7CogY*sin(q6)*sin(q7)) - cos(q4)*(sin(q5)*(KUKA_LBR_param_.dblLink7CogY*cos(q7) + KUKA_LBR_param_.dblLink7CogX*sin(q7)) + cos(q5)*(-(KUKA_LBR_param_.dblLink7CogX*cos(q6)*cos(q7)) + KUKA_LBR_param_.dblLink7CogZ*sin(q6) + KUKA_LBR_param_.dblLink7CogY*cos(q6)*sin(q7))))) + cos(q1)*cos(q2)*(cos(q3)*(cos(q5)*(KUKA_LBR_param_.dblLink7CogY*cos(q7) + KUKA_LBR_param_.dblLink7CogX*sin(q7)) + sin(q5)*(KUKA_LBR_param_.dblLink7CogX*cos(q6)*cos(q7) - KUKA_LBR_param_.dblLink7CogZ*sin(q6) - KUKA_LBR_param_.dblLink7CogY*cos(q6)*sin(q7))) + sin(q3)*(sin(q4)*(KUKA_LBR_param_.dblLink45Len + KUKA_LBR_param_.dblLink7CogZ*cos(q6) + KUKA_LBR_param_.dblLink7CogX*cos(q7)*sin(q6) - KUKA_LBR_param_.dblLink7CogY*sin(q6)*sin(q7)) - cos(q4)*(sin(q5)*(KUKA_LBR_param_.dblLink7CogY*cos(q7) + KUKA_LBR_param_.dblLink7CogX*sin(q7)) + cos(q5)*(-(KUKA_LBR_param_.dblLink7CogX*cos(q6)*cos(q7)) + KUKA_LBR_param_.dblLink7CogZ*sin(q6) + KUKA_LBR_param_.dblLink7CogY*cos(q6)*sin(q7))))))*(-(sin(q1)*(cos(q6)*(-(KUKA_LBR_param_.dblLink7CogX*cos(q7)*sin(q3)*sin(q4)) + KUKA_LBR_param_.dblLink7CogZ*cos(q3)*sin(q5) + KUKA_LBR_param_.dblLink7CogY*sin(q3)*sin(q4)*sin(q7)) + sin(q6)*(KUKA_LBR_param_.dblLink7CogZ*sin(q3)*sin(q4) + cos(q3)*sin(q5)*(KUKA_LBR_param_.dblLink7CogX*cos(q7) - KUKA_LBR_param_.dblLink7CogY*sin(q7))) + cos(q4)*cos(q5)*sin(q3)*(KUKA_LBR_param_.dblLink7CogZ*cos(q6) + sin(q6)*(KUKA_LBR_param_.dblLink7CogX*cos(q7) - KUKA_LBR_param_.dblLink7CogY*sin(q7))))) + cos(q1)*(sin(q2)*(cos(q4)*(KUKA_LBR_param_.dblLink7CogX*cos(q6)*cos(q7) - KUKA_LBR_param_.dblLink7CogZ*sin(q6) - KUKA_LBR_param_.dblLink7CogY*cos(q6)*sin(q7)) + cos(q5)*sin(q4)*(KUKA_LBR_param_.dblLink7CogZ*cos(q6) + KUKA_LBR_param_.dblLink7CogX*cos(q7)*sin(q6) - KUKA_LBR_param_.dblLink7CogY*sin(q6)*sin(q7))) + cos(q2)*(-(sin(q3)*sin(q5)*(KUKA_LBR_param_.dblLink7CogZ*cos(q6) + sin(q6)*(KUKA_LBR_param_.dblLink7CogX*cos(q7) - KUKA_LBR_param_.dblLink7CogY*sin(q7)))) + cos(q3)*(sin(q4)*(-(KUKA_LBR_param_.dblLink7CogX*cos(q6)*cos(q7)) + KUKA_LBR_param_.dblLink7CogZ*sin(q6) + KUKA_LBR_param_.dblLink7CogY*cos(q6)*sin(q7)) + cos(q4)*cos(q5)*(KUKA_LBR_param_.dblLink7CogZ*cos(q6) + KUKA_LBR_param_.dblLink7CogX*cos(q7)*sin(q6) - KUKA_LBR_param_.dblLink7CogY*sin(q6)*sin(q7))))));
